simulink model "DYN_01x"  (R2018b)
(part 13 of 13)

 2*I6xy*de1*cos(e2)^2 - I6xy*de1 + 2*I6xy*de1*cos(e3)^2 + I6xy*de1*cos(e4)^2 + 2*I6xy*de1*cos(e6)^2 - (I6xx*de1*sin(2*e6))/2 + (I6yy*de1*sin(2*e6))/2 - de1*m6*x6*y6 + (de1*m6*x6^2*sin(2*e6))/2 - (de1*m6*y6^2*sin(2*e6))/2 - 4*I6xy*de1*cos(e2)^2*cos(e3)^2 - I6xy*de1*cos(e2)^2*cos(e4)^2 - I6xy*de1*cos(e2)^2*cos(e5)^2 - I6xy*de1*cos(e3)^2*cos(e4)^2 - 4*I6xy*de1*cos(e2)^2*cos(e6)^2 - I6xy*de1*cos(e3)^2*cos(e5)^2 - 4*I6xy*de1*cos(e3)^2*cos(e6)^2 + I6xy*de1*cos(e4)^2*cos(e5)^2 - 2*I6xy*de1*cos(e4)^2*cos(e6)^2 - I6xy*de4*cos(e2)*sin(e3) - I6xy*de4*cos(e3)*sin(e2) + 2*de1*m6*x6*y6*cos(e2)^2 + 2*de1*m6*x6*y6*cos(e3)^2 + de1*m6*x6*y6*cos(e4)^2 + 2*de1*m6*x6*y6*cos(e6)^2 + (I6xx*de2*cos(e2)*cos(e3)*cos(e5))/2 + (I6xx*de3*cos(e2)*cos(e3)*cos(e5))/2 - (I6yy*de2*cos(e2)*cos(e3)*cos(e5))/2 - (I6yy*de3*cos(e2)*cos(e3)*cos(e5))/2 - (I6zz*de2*cos(e2)*cos(e3)*cos(e5))/2 - (I6zz*de3*cos(e2)*cos(e3)*cos(e5))/2 - I6xx*de1*cos(e4)*cos(e5)*sin(e4) - I6xy*de5*cos(e2)*cos(e3)*sin(e4) + I6yy*de1*cos(e4)*cos(e5)*sin(e4) + 2*I6xy*de1*cos(e2)^2*cos(e3)^2*cos(e4)^2 + 2*I6xy*de1*cos(e2)^2*cos(e3)^2*cos(e5)^2 + 8*I6xy*de1*cos(e2)^2*cos(e3)^2*cos(e6)^2 - I6xy*de1*cos(e2)^2*cos(e4)^2*cos(e5)^2 + 2*I6xy*de1*cos(e2)^2*cos(e4)^2*cos(e6)^2 - I6xy*de1*cos(e3)^2*cos(e4)^2*cos(e5)^2 + 2*I6xy*de1*cos(e2)^2*cos(e5)^2*cos(e6)^2 + 2*I6xy*de1*cos(e3)^2*cos(e4)^2*cos(e6)^2 + 2*I6xy*de1*cos(e3)^2*cos(e5)^2*cos(e6)^2 - 2*I6xy*de1*cos(e4)^2*cos(e5)^2*cos(e6)^2 - (I6xx*de2*cos(e5)*sin(e2)*sin(e3))/2 - (I6xx*de3*cos(e5)*sin(e2)*sin(e3))/2 + (I6xx*de5*cos(e2)*sin(e3)*sin(e5))/2 + (I6xx*de5*cos(e3)*sin(e2)*sin(e5))/2 + (I6yy*de2*cos(e5)*sin(e2)*sin(e3))/2 + (I6yy*de3*cos(e5)*sin(e2)*sin(e3))/2 - (I6yy*de5*cos(e2)*sin(e3)*sin(e5))/2 - (I6yy*de5*cos(e3)*sin(e2)*sin(e5))/2 + (I6zz*de2*cos(e5)*sin(e2)*sin(e3))/2 + (I6zz*de3*cos(e5)*sin(e2)*sin(e3))/2 + (I6zz*de5*cos(e2)*sin(e3)*sin(e5))/2 + (I6zz*de5*cos(e3)*sin(e2)*sin(e5))/2 + I6xy*de5*sin(e2)*sin(e3)*sin(e4) + 2*I6xx*de1*cos(e2)^2*cos(e6)*sin(e6) + I6xy*de4*cos(e2)*cos(e5)^2*sin(e3) + I6xy*de4*cos(e3)*cos(e5)^2*sin(e2) + 2*I6xx*de1*cos(e3)^2*cos(e6)*sin(e6) + 2*I6xy*de4*cos(e2)*cos(e6)^2*sin(e3) + 2*I6xy*de4*cos(e3)*cos(e6)^2*sin(e2) + I6xx*de1*cos(e4)^2*cos(e6)*sin(e6) - 2*I6yy*de1*cos(e2)^2*cos(e6)*sin(e6) - 2*I6yy*de1*cos(e3)^2*cos(e6)*sin(e6) - I6yy*de1*cos(e4)^2*cos(e6)*sin(e6) - (I6xx*de5*cos(e2)*cos(e3)*cos(e4)*cos(e5))/2 + (I6yy*de5*cos(e2)*cos(e3)*cos(e4)*cos(e5))/2 + I6yz*de4*cos(e2)*cos(e3)*cos(e4)*cos(e6) - (I6zz*de5*cos(e2)*cos(e3)*cos(e4)*cos(e5))/2 - I6xy*de2*cos(e2)*cos(e3)*cos(e4)*sin(e4) - I6xy*de3*cos(e2)*cos(e3)*cos(e4)*sin(e4) + I6yz*de1*cos(e2)*cos(e4)*cos(e6)*sin(e2) + I6yz*de1*cos(e3)*cos(e4)*cos(e6)*sin(e3) + I6zx*de4*cos(e2)*cos(e3)*cos(e4)*sin(e6) + I6zx*de5*cos(e2)*cos(e5)*cos(e6)*sin(e3) + I6zx*de5*cos(e3)*cos(e5)*cos(e6)*sin(e2) + 4*I6xy*de1*cos(e2)*cos(e3)*sin(e2)*sin(e3) + (I6xx*de2*cos(e2)*cos(e4)*sin(e3)*sin(e5))/2 + (I6xx*de2*cos(e3)*cos(e4)*sin(e2)*sin(e5))/2 + (I6xx*de3*cos(e2)*cos(e4)*sin(e3)*sin(e5))/2 + (I6xx*de3*cos(e3)*cos(e4)*sin(e2)*sin(e5))/2 - (I6xx*de4*cos(e2)*cos(e3)*sin(e4)*sin(e5))/2 + (I6xx*de5*cos(e4)*cos(e5)*sin(e2)*sin(e3))/2 - I6xx*de4*cos(e2)*cos(e6)*sin(e3)*sin(e6) - I6xx*de4*cos(e3)*cos(e6)*sin(e2)*sin(e6) - (I6yy*de2*cos(e2)*cos(e4)*sin(e3)*sin(e5))/2 - (I6yy*de2*cos(e3)*cos(e4)*sin(e2)*sin(e5))/2 - (I6yy*de3*cos(e2)*cos(e4)*sin(e3)*sin(e5))/2 - (I6yy*de3*cos(e3)*cos(e4)*sin(e2)*sin(e5))/2 + (I6yy*de4*cos(e2)*cos(e3)*sin(e4)*sin(e5))/2 - (I6yy*de5*cos(e4)*cos(e5)*sin(e2)*sin(e3))/2 - I6yz*de4*cos(e4)*cos(e6)*sin(e2)*sin(e3) + I6yy*de4*cos(e2)*cos(e6)*sin(e3)*sin(e6) + I6yy*de4*cos(e3)*cos(e6)*sin(e2)*sin(e6) - I6yz*de5*cos(e2)*cos(e5)*sin(e3)*sin(e6) - I6yz*de5*cos(e3)*cos(e5)*sin(e2)*sin(e6) + I6zx*de1*cos(e2)*cos(e4)*sin(e2)*sin(e6) + I6zx*de1*cos(e3)*cos(e4)*sin(e3)*sin(e6) + (I6zz*de2*cos(e2)*cos(e4)*sin(e3)*sin(e5))/2 + (I6zz*de2*cos(e3)*cos(e4)*sin(e2)*sin(e5))/2 + (I6zz*de3*cos(e2)*cos(e4)*sin(e3)*sin(e5))/2 + (I6zz*de3*cos(e3)*cos(e4)*sin(e2)*sin(e5))/2 + I6zx*de1*cos(e4)*cos(e6)*sin(e4)*sin(e5) + (I6zz*de4*cos(e2)*cos(e3)*sin(e4)*sin(e5))/2 + (I6zz*de5*cos(e4)*cos(e5)*sin(e2)*sin(e3))/2 - I6xx*de1*cos(e2)*sin(e2)*sin(e4)*sin(e5) - I6xx*de1*cos(e3)*sin(e3)*sin(e4)*sin(e5) + I6xy*de2*cos(e4)*sin(e2)*sin(e3)*sin(e4) + I6xy*de3*cos(e4)*sin(e2)*sin(e3)*sin(e4) + I6yy*de1*cos(e2)*sin(e2)*sin(e4)*sin(e5) + I6yy*de1*cos(e3)*sin(e3)*sin(e4)*sin(e5) - I6yz*de1*cos(e4)*sin(e4)*sin(e5)*sin(e6) - I6zx*de4*cos(e4)*sin(e2)*sin(e3)*sin(e6) - de2*m6*x6^2*cos(e2)*cos(e3)*cos(e5) - de3*m6*x6^2*cos(e2)*cos(e3)*cos(e5) + (I6xx*de4*sin(e2)*sin(e3)*sin(e4)*sin(e5))/2 - (I6yy*de4*sin(e2)*sin(e3)*sin(e4)*sin(e5))/2 - (I6zz*de4*sin(e2)*sin(e3)*sin(e4)*sin(e5))/2 + de1*m6*x6^2*cos(e4)*cos(e5)*sin(e4) - 4*de1*m6*x6*y6*cos(e2)^2*cos(e3)^2 - de1*m6*x6*y6*cos(e2)^2*cos(e4)^2 - de1*m6*x6*y6*cos(e2)^2*cos(e5)^2 - de1*m6*x6*y6*cos(e3)^2*cos(e4)^2 - 4*de1*m6*x6*y6*cos(e2)^2*cos(e6)^2 - de1*m6*x6*y6*cos(e3)^2*cos(e5)^2 - 4*de1*m6*x6*y6*cos(e3)^2*cos(e6)^2 + de1*m6*x6*y6*cos(e4)^2*cos(e5)^2 - 2*de1*m6*x6*y6*cos(e4)^2*cos(e6)^2 - de1*m6*y6^2*cos(e4)*cos(e5)*sin(e4) + de2*m6*x6^2*cos(e5)*sin(e2)*sin(e3) + de3*m6*x6^2*cos(e5)*sin(e2)*sin(e3) + de5*m6*y6^2*cos(e2)*sin(e3)*sin(e5) + de5*m6*y6^2*cos(e3)*sin(e2)*sin(e5) - I6xx*de2*cos(e2)*cos(e3)*cos(e4)^2*cos(e5) - I6xx*de3*cos(e2)*cos(e3)*cos(e4)^2*cos(e5) - I6xx*de2*cos(e2)*cos(e3)*cos(e5)*cos(e6)^2 - I6xx*de3*cos(e2)*cos(e3)*cos(e5)*cos(e6)^2 + I6yy*de2*cos(e2)*cos(e3)*cos(e4)^2*cos(e5) + I6yy*de3*cos(e2)*cos(e3)*cos(e4)^2*cos(e5) + I6yy*de2*cos(e2)*cos(e3)*cos(e5)*cos(e6)^2 + I6yy*de3*cos(e2)*cos(e3)*cos(e5)*cos(e6)^2 + I6xx*de1*cos(e2)^2*cos(e4)*cos(e5)*sin(e4) + I6xx*de1*cos(e3)^2*cos(e4)*cos(e5)*sin(e4) + 2*I6xx*de1*cos(e4)*cos(e5)*cos(e6)^2*sin(e4) + 2*I6xy*de5*cos(e2)*cos(e3)*cos(e6)^2*sin(e4) - I6yy*de1*cos(e2)^2*cos(e4)*cos(e5)*sin(e4) - I6yy*de1*cos(e3)^2*cos(e4)*cos(e5)*sin(e4) - 2*I6yy*de1*cos(e4)*cos(e5)*cos(e6)^2*sin(e4) - I6yz*de1*cos(e2)^2*cos(e5)*cos(e6)*sin(e5) - I6yz*de1*cos(e3)^2*cos(e5)*cos(e6)*sin(e5) + I6yz*de1*cos(e4)^2*cos(e5)*cos(e6)*sin(e5) + 2*I6xy*de1*cos(e2)^2*cos(e3)^2*cos(e4)^2*cos(e5)^2 - 4*I6xy*de1*cos(e2)^2*cos(e3)^2*cos(e4)^2*cos(e6)^2 - 4*I6xy*de1*cos(e2)^2*cos(e3)^2*cos(e5)^2*cos(e6)^2 + 2*I6xy*de1*cos(e2)^2*cos(e4)^2*cos(e5)^2*cos(e6)^2 + 2*I6xy*de1*cos(e3)^2*cos(e4)^2*cos(e5)^2*cos(e6)^2 + I6xx*de2*cos(e4)^2*cos(e5)*sin(e2)*sin(e3) + I6xx*de3*cos(e4)^2*cos(e5)*sin(e2)*sin(e3) + I6xx*de2*cos(e5)*cos(e6)^2*sin(e2)*sin(e3) + I6xx*de3*cos(e5)*cos(e6)^2*sin(e2)*sin(e3) - I6xx*de5*cos(e2)*cos(e6)^2*sin(e3)*sin(e5) - I6xx*de5*cos(e3)*cos(e6)^2*sin(e2)*sin(e5) - I6yy*de2*cos(e4)^2*cos(e5)*sin(e2)*sin(e3) - I6yy*de3*cos(e4)^2*cos(e5)*sin(e2)*sin(e3) - I6yy*de2*cos(e5)*cos(e6)^2*sin(e2)*sin(e3) - I6yy*de3*cos(e5)*cos(e6)^2*sin(e2)*sin(e3) + I6yy*de5*cos(e2)*cos(e6)^2*sin(e3)*sin(e5) + I6yy*de5*cos(e3)*cos(e6)^2*sin(e2)*sin(e5) - I6zx*de1*cos(e2)^2*cos(e5)*sin(e5)*sin(e6) - I6zx*de1*cos(e3)^2*cos(e5)*sin(e5)*sin(e6) + I6zx*de1*cos(e4)^2*cos(e5)*sin(e5)*sin(e6) + d4*de1*m6*y6*cos(e6)*sin(e5) + d4*de1*m6*x6*sin(e5)*sin(e6) - 2*I6xy*de5*cos(e6)^2*sin(e2)*sin(e3)*sin(e4) - de4*m6*x6*y6*cos(e2)*sin(e3) - de4*m6*x6*y6*cos(e3)*sin(e2) - 2*de1*m6*x6^2*cos(e2)^2*cos(e6)*sin(e6) - 2*de1*m6*x6^2*cos(e3)^2*cos(e6)*sin(e6) - de1*m6*x6^2*cos(e4)^2*cos(e6)*sin(e6) + 2*de1*m6*y6^2*cos(e2)^2*cos(e6)*sin(e6) + 2*de1*m6*y6^2*cos(e3)^2*cos(e6)*sin(e6) + de1*m6*y6^2*cos(e4)^2*cos(e6)*sin(e6) - 4*I6xx*de1*cos(e2)^2*cos(e3)^2*cos(e6)*sin(e6) - I6xx*de1*cos(e2)^2*cos(e4)^2*cos(e6)*sin(e6) - I6xx*de1*cos(e2)^2*cos(e5)^2*cos(e6)*sin(e6) - I6xx*de1*cos(e3)^2*cos(e4)^2*cos(e6)*sin(e6) - I6xx*de1*cos(e3)^2*cos(e5)^2*cos(e6)*sin(e6) - 2*I6xy*de4*cos(e2)*cos(e5)^2*cos(e6)^2*sin(e3) - 2*I6xy*de4*cos(e3)*cos(e5)^2*cos(e6)^2*sin(e2) + I6xx*de1*cos(e4)^2*cos(e5)^2*cos(e6)*sin(e6) + 4*I6yy*de1*cos(e2)^2*cos(e3)^2*cos(e6)*sin(e6) + I6yy*de1*cos(e2)^2*cos(e4)^2*cos(e6)*sin(e6) + I6yy*de1*cos(e2)^2*cos(e5)^2*cos(e6)*sin(e6) + I6yy*de1*cos(e3)^2*cos(e4)^2*cos(e6)*sin(e6) + I6yy*de1*cos(e3)^2*cos(e5)^2*cos(e6)*sin(e6) - I6yy*de1*cos(e4)^2*cos(e5)^2*cos(e6)*sin(e6) + I6xy*de4*cos(e2)*cos(e3)*cos(e4)*cos(e5)*sin(e5) - 2*I6xy*de2*cos(e2)*cos(e3)*cos(e5)*cos(e6)*sin(e6) - 2*I6xy*de3*cos(e2)*cos(e3)*cos(e5)*cos(e6)*sin(e6) + I6zx*de2*cos(e2)*cos(e4)*cos(e5)*cos(e6)*sin(e3) + I6zx*de2*cos(e3)*cos(e4)*cos(e5)*cos(e6)*sin(e2) + I6zx*de3*cos(e2)*cos(e4)*cos(e5)*cos(e6)*sin(e3) + I6zx*de3*cos(e3)*cos(e4)*cos(e5)*cos(e6)*sin(e2) + I6zx*de5*cos(e2)*cos(e3)*cos(e4)*cos(e6)*sin(e5) + 2*I6xy*de1*cos(e2)*cos(e4)*cos(e5)*sin(e2)*sin(e5) + 2*I6xy*de1*cos(e3)*cos(e4)*cos(e5)*sin(e3)*sin(e5) - I6xx*de5*cos(e2)*cos(e3)*cos(e6)*sin(e4)*sin(e6) + 4*I6xy*de1*cos(e4)*cos(e5)*cos(e6)*sin(e4)*sin(e6) - I6yz*de2*cos(e2)*cos(e4)*cos(e5)*sin(e3)*sin(e6) - I6yz*de2*cos(e3)*cos(e4)*cos(e5)*sin(e2)*sin(e6) - I6yz*de3*cos(e2)*cos(e4)*cos(e5)*sin(e3)*sin(e6) - I6yz*de3*cos(e3)*cos(e4)*cos(e5)*sin(e2)*sin(e6) + I6yy*de5*cos(e2)*cos(e3)*cos(e6)*sin(e4)*sin(e6) + I6yz*de4*cos(e2)*cos(e5)*cos(e6)*sin(e3)*sin(e5) + I6yz*de4*cos(e3)*cos(e5)*cos(e6)*sin(e2)*sin(e5) - I6yz*de5*cos(e2)*cos(e3)*cos(e4)*sin(e5)*sin(e6) - I6zx*de1*cos(e2)*cos(e5)*cos(e6)*sin(e2)*sin(e4) - I6zx*de1*cos(e3)*cos(e5)*cos(e6)*sin(e3)*sin(e4) + 2*I6xx*de1*cos(e2)^2*cos(e3)^2*cos(e4)^2*cos(e6)*sin(e6) + 2*I6xx*de1*cos(e2)^2*cos(e3)^2*cos(e5)^2*cos(e6)*sin(e6) - I6xx*de1*cos(e2)^2*cos(e4)^2*cos(e5)^2*cos(e6)*sin(e6) - I6xx*de1*cos(e3)^2*cos(e4)^2*cos(e5)^2*cos(e6)*sin(e6) - 2*I6yy*de1*cos(e2)^2*cos(e3)^2*cos(e4)^2*cos(e6)*sin(e6) - 2*I6yy*de1*cos(e2)^2*cos(e3)^2*cos(e5)^2*cos(e6)*sin(e6) + I6yy*de1*cos(e2)^2*cos(e4)^2*cos(e5)^2*cos(e6)*sin(e6) + I6yy*de1*cos(e3)^2*cos(e4)^2*cos(e5)^2*cos(e6)*sin(e6) + I6xy*de2*cos(e2)*cos(e5)*sin(e3)*sin(e4)*sin(e5) + I6xy*de2*cos(e3)*cos(e5)*sin(e2)*sin(e4)*sin(e5) + I6xy*de3*cos(e2)*cos(e5)*sin(e3)*sin(e4)*sin(e5) + I6xy*de3*cos(e3)*cos(e5)*sin(e2)*sin(e4)*sin(e5) - I6xy*de4*cos(e4)*cos(e5)*sin(e2)*sin(e3)*sin(e5) + 2*I6xy*de2*cos(e5)*cos(e6)*sin(e2)*sin(e3)*sin(e6) + 2*I6xy*de3*cos(e5)*cos(e6)*sin(e2)*sin(e3)*sin(e6) - 2*I6xy*de5*cos(e2)*cos(e6)*sin(e3)*sin(e5)*sin(e6) - 2*I6xy*de5*cos(e3)*cos(e6)*sin(e2)*sin(e5)*sin(e6) + I6yz*de1*cos(e2)*cos(e5)*sin(e2)*sin(e4)*sin(e6) + I6yz*de1*cos(e3)*cos(e5)*sin(e3)*sin(e4)*sin(e6) + I6zx*de4*cos(e2)*cos(e5)*sin(e3)*sin(e5)*sin(e6) + I6zx*de4*cos(e3)*cos(e5)*sin(e2)*sin(e5)*sin(e6) - I6zx*de5*cos(e4)*cos(e6)*sin(e2)*sin(e3)*sin(e5) - de5*m6*y6^2*cos(e2)*cos(e3)*cos(e4)*cos(e5) + I6xx*de5*cos(e6)*sin(e2)*sin(e3)*sin(e4)*sin(e6) - I6yy*de5*cos(e6)*sin(e2)*sin(e3)*sin(e4)*sin(e6) + I6yz*de5*cos(e4)*sin(e2)*sin(e3)*sin(e5)*sin(e6) + de4*m6*x6^2*cos(e2)*cos(e3)*sin(e4)*sin(e5) + de4*m6*x6^2*cos(e2)*cos(e6)*sin(e3)*sin(e6) + de4*m6*x6^2*cos(e3)*cos(e6)*sin(e2)*sin(e6) + de2*m6*y6^2*cos(e2)*cos(e4)*sin(e3)*sin(e5) + de2*m6*y6^2*cos(e3)*cos(e4)*sin(e2)*sin(e5) + de3*m6*y6^2*cos(e2)*cos(e4)*sin(e3)*sin(e5) + de3*m6*y6^2*cos(e3)*cos(e4)*sin(e2)*sin(e5) + de5*m6*y6^2*cos(e4)*cos(e5)*sin(e2)*sin(e3) - de4*m6*y6^2*cos(e2)*cos(e6)*sin(e3)*sin(e6) - de4*m6*y6^2*cos(e3)*cos(e6)*sin(e2)*sin(e6) + I6xx*de5*cos(e2)*cos(e3)*cos(e4)*cos(e5)*cos(e6)^2 - I6yy*de5*cos(e2)*cos(e3)*cos(e4)*cos(e5)*cos(e6)^2 - I6yz*de4*cos(e2)*cos(e3)*cos(e4)*cos(e5)^2*cos(e6) + de1*m6*x6^2*cos(e2)*sin(e2)*sin(e4)*sin(e5) + de1*m6*x6^2*cos(e3)*sin(e3)*sin(e4)*sin(e5) - de1*m6*y6^2*cos(e2)*sin(e2)*sin(e4)*sin(e5) - de1*m6*y6^2*cos(e3)*sin(e3)*sin(e4)*sin(e5) - a2*de2*m6*x6*cos(e2)*cos(e4)*cos(e6) - I6xy*de2*cos(e2)*cos(e3)*cos(e4)*cos(e5)^2*sin(e4) + 2*I6xy*de2*cos(e2)*cos(e3)*cos(e4)*cos(e6)^2*sin(e4) - I6xy*de3*cos(e2)*cos(e3)*cos(e4)*cos(e5)^2*sin(e4) + 2*I6xy*de3*cos(e2)*cos(e3)*cos(e4)*cos(e6)^2*sin(e4) - 2*I6yz*de1*cos(e2)*cos(e3)^2*cos(e4)*cos(e6)*sin(e2) - 2*I6yz*de1*cos(e2)^2*cos(e3)*cos(e4)*cos(e6)*sin(e3) - 2*I6yz*de1*cos(e2)*cos(e4)*cos(e5)^2*cos(e6)*sin(e2) - 2*I6yz*de1*cos(e3)*cos(e4)*cos(e5)^2*cos(e6)*sin(e3) + I6zx*de2*cos(e2)*cos(e3)*cos(e4)^2*cos(e6)*sin(e5) + I6zx*de3*cos(e2)*cos(e3)*cos(e4)^2*cos(e6)*sin(e5) - I6zx*de4*cos(e2)*cos(e3)*cos(e4)*cos(e5)^2*sin(e6) - de4*m6*x6^2*sin(e2)*sin(e3)*sin(e4)*sin(e5) + a2*de1*m6*x6*cos(e3)*cos(e6)*sin(e4) + a2*de2*m6*y6*cos(e2)*cos(e4)*sin(e6) - 2*I6xy*de1*cos(e2)*cos(e3)*cos(e4)^2*sin(e2)*sin(e3) - 2*I6xy*de1*cos(e2)*cos(e3)*cos(e5)^2*sin(e2)*sin(e3) - 8*I6xy*de1*cos(e2)*cos(e3)*cos(e6)^2*sin(e2)*sin(e3) - I6xx*de2*cos(e2)*cos(e4)*cos(e6)^2*sin(e3)*sin(e5) - I6xx*de2*cos(e3)*cos(e4)*cos(e6)^2*sin(e2)*sin(e5) - I6xx*de3*cos(e2)*cos(e4)*cos(e6)^2*sin(e3)*sin(e5) - I6xx*de3*cos(e3)*cos(e4)*cos(e6)^2*sin(e2)*sin(e5) + I6xx*de4*cos(e2)*cos(e3)*cos(e6)^2*sin(e4)*sin(e5) - I6xx*de5*cos(e4)*cos(e5)*cos(e6)^2*sin(e2)*sin(e3) + I6xx*de4*cos(e2)*cos(e5)^2*cos(e6)*sin(e3)*sin(e6) + I6xx*de4*cos(e3)*cos(e5)^2*cos(e6)*sin(e2)*sin(e6) + I6yy*de2*cos(e2)*cos(e4)*cos(e6)^2*sin(e3)*sin(e5) + I6yy*de2*cos(e3)*cos(e4)*cos(e6)^2*sin(e2)*sin(e5) + I6yy*de3*cos(e2)*cos(e4)*cos(e6)^2*sin(e3)*sin(e5) + I6yy*de3*cos(e3)*cos(e4)*cos(e6)^2*sin(e2)*sin(e5) - I6yz*de2*cos(e2)*cos(e3)*cos(e4)^2*sin(e5)*sin(e6) - I6yz*de2*cos(e2)*cos(e5)^2*cos(e6)*sin(e3)*sin(e4) - I6yz*de2*cos(e3)*cos(e5)^2*cos(e6)*sin(e2)*sin(e4) - I6yy*de4*cos(e2)*cos(e3)*cos(e6)^2*sin(e4)*sin(e5) - I6yz*de3*cos(e2)*cos(e3)*cos(e4)^2*sin(e5)*sin(e6) - I6yz*de3*cos(e2)*cos(e5)^2*cos(e6)*sin(e3)*sin(e4) - I6yz*de3*cos(e3)*cos(e5)^2*cos(e6)*sin(e2)*sin(e4) + I6yy*de5*cos(e4)*cos(e5)*cos(e6)^2*sin(e2)*sin(e3) + I6yz*de4*cos(e4)*cos(e5)^2*cos(e6)*sin(e2)*sin(e3) - I6yy*de4*cos(e2)*cos(e5)^2*cos(e6)*sin(e3)*sin(e6) - I6yy*de4*cos(e3)*cos(e5)^2*cos(e6)*sin(e2)*sin(e6) - 2*I6zx*de1*cos(e2)*cos(e3)^2*cos(e4)*sin(e2)*sin(e6) - 2*I6zx*de1*cos(e2)^2*cos(e3)*cos(e4)*sin(e3)*sin(e6) - 2*I6zx*de1*cos(e2)*cos(e4)*cos(e5)^2*sin(e2)*sin(e6) - 2*I6zx*de1*cos(e3)*cos(e4)*cos(e5)^2*sin(e3)*sin(e6) - I6zx*de1*cos(e2)^2*cos(e4)*cos(e6)*sin(e4)*sin(e5) - I6zx*de1*cos(e3)^2*cos(e4)*cos(e6)*sin(e4)*sin(e5) - a2*de1*m6*y6*cos(e3)*sin(e4)*sin(e6) - a2*de1*m6*y6*cos(e6)*sin(e3)*sin(e5) + 2*I6xx*de1*cos(e2)*cos(e3)^2*sin(e2)*sin(e4)*sin(e5) + 2*I6xx*de1*cos(e2)^2*cos(e3)*sin(e3)*sin(e4)*sin(e5) + 2*I6xx*de1*cos(e2)*cos(e6)^2*sin(e2)*sin(e4)*sin(e5) + I6xy*de2*cos(e4)*cos(e5)^2*sin(e2)*sin(e3)*sin(e4) + 2*I6xx*de1*cos(e3)*cos(e6)^2*sin(e3)*sin(e4)*sin(e5) - 2*I6xy*de2*cos(e4)*cos(e6)^2*sin(e2)*sin(e3)*sin(e4) + I6xy*de3*cos(e4)*cos(e5)^2*sin(e2)*sin(e3)*sin(e4) - 2*I6xy*de3*cos(e4)*cos(e6)^2*sin(e2)*sin(e3)*sin(e4) - 2*I6yy*de1*cos(e2)*cos(e3)^2*sin(e2)*sin(e4)*sin(e5) - 2*I6yy*de1*cos(e2)^2*cos(e3)*sin(e3)*sin(e4)*sin(e5) - 2*I6yy*de1*cos(e2)*cos(e6)^2*sin(e2)*sin(e4)*sin(e5) - 2*I6yy*de1*cos(e3)*cos(e6)^2*sin(e3)*sin(e4)*sin(e5) + I6yz*de1*cos(e2)^2*cos(e4)*sin(e4)*sin(e5)*sin(e6) + I6yz*de1*cos(e3)^2*cos(e4)*sin(e4)*sin(e5)*sin(e6) - I6zx*de2*cos(e2)*cos(e5)^2*sin(e3)*sin(e4)*sin(e6) - I6zx*de2*cos(e3)*cos(e5)^2*sin(e2)*sin(e4)*sin(e6) - I6zx*de2*cos(e4)^2*cos(e6)*sin(e2)*sin(e3)*sin(e5) - I6zx*de3*cos(e2)*cos(e5)^2*sin(e3)*sin(e4)*sin(e6) - I6zx*de3*cos(e3)*cos(e5)^2*sin(e2)*sin(e4)*sin(e6) - I6zx*de3*cos(e4)^2*cos(e6)*sin(e2)*sin(e3)*sin(e5) + I6zx*de4*cos(e4)*cos(e5)^2*sin(e2)*sin(e3)*sin(e6) + de2*m6*x6^2*cos(e2)*cos(e3)*cos(e4)^2*cos(e5) + de3*m6*x6^2*cos(e2)*cos(e3)*cos(e4)^2*cos(e5) + de2*m6*x6^2*cos(e2)*cos(e3)*cos(e5)*cos(e6)^2 + de3*m6*x6^2*cos(e2)*cos(e3)*cos(e5)*cos(e6)^2 - de2*m6*y6^2*cos(e2)*cos(e3)*cos(e4)^2*cos(e5) - de3*m6*y6^2*cos(e2)*cos(e3)*cos(e4)^2*cos(e5) - de2*m6*y6^2*cos(e2)*cos(e3)*cos(e5)*cos(e6)^2 - de3*m6*y6^2*cos(e2)*cos(e3)*cos(e5)*cos(e6)^2 - de5*m6*x6*y6*cos(e2)*cos(e3)*sin(e4) - a2*de1*m6*x6*sin(e3)*sin(e5)*sin(e6) - I6xx*de4*cos(e6)^2*sin(e2)*sin(e3)*sin(e4)*sin(e5) + I6yz*de2*cos(e4)^2*sin(e2)*sin(e3)*sin(e5)*sin(e6) + I6yy*de4*cos(e6)^2*sin(e2)*sin(e3)*sin(e4)*sin(e5) + I6yz*de3*cos(e4)^2*sin(e2)*sin(e3)*sin(e5)*sin(e6) - de1*m6*x6^2*cos(e2)^2*cos(e4)*cos(e5)*sin(e4) - de1*m6*x6^2*cos(e3)^2*cos(e4)*cos(e5)*sin(e4) - 2*de1*m6*x6^2*cos(e4)*cos(e5)*cos(e6)^2*sin(e4) + 2*de1*m6*x6*y6*cos(e2)^2*cos(e3)^2*cos(e4)^2 + 2*de1*m6*x6*y6*cos(e2)^2*cos(e3)^2*cos(e5)^2 + 8*de1*m6*x6*y6*cos(e2)^2*cos(e3)^2*cos(e6)^2 - de1*m6*x6*y6*cos(e2)^2*cos(e4)^2*cos(e5)^2 + 2*de1*m6*x6*y6*cos(e2)^2*cos(e4)^2*cos(e6)^2 - de1*m6*x6*y6*cos(e3)^2*cos(e4)^2*cos(e5)^2 + 2*de1*m6*x6*y6*cos(e2)^2*cos(e5)^2*cos(e6)^2 + 2*de1*m6*x6*y6*cos(e3)^2*cos(e4)^2*cos(e6)^2 + 2*de1*m6*x6*y6*cos(e3)^2*cos(e5)^2*cos(e6)^2 - 2*de1*m6*x6*y6*cos(e4)^2*cos(e5)^2*cos(e6)^2 + de1*m6*y6^2*cos(e2)^2*cos(e4)*cos(e5)*sin(e4) + de1*m6*y6^2*cos(e3)^2*cos(e4)*cos(e5)*sin(e4) + 2*de1*m6*y6^2*cos(e4)*cos(e5)*cos(e6)^2*sin(e4) - de2*m6*x6^2*cos(e4)^2*cos(e5)*sin(e2)*sin(e3) - de3*m6*x6^2*cos(e4)^2*cos(e5)*sin(e2)*sin(e3) - de2*m6*x6^2*cos(e5)*cos(e6)^2*sin(e2)*sin(e3) - de3*m6*x6^2*cos(e5)*cos(e6)^2*sin(e2)*sin(e3) + de5*m6*x6^2*cos(e2)*cos(e6)^2*sin(e3)*sin(e5) + de5*m6*x6^2*cos(e3)*cos(e6)^2*sin(e2)*sin(e5) + de2*m6*y6^2*cos(e4)^2*cos(e5)*sin(e2)*sin(e3) + de3*m6*y6^2*cos(e4)^2*cos(e5)*sin(e2)*sin(e3) + de2*m6*y6^2*cos(e5)*cos(e6)^2*sin(e2)*sin(e3) + de3*m6*y6^2*cos(e5)*cos(e6)^2*sin(e2)*sin(e3) - de5*m6*y6^2*cos(e2)*cos(e6)^2*sin(e3)*sin(e5) - de5*m6*y6^2*cos(e3)*cos(e6)^2*sin(e2)*sin(e5) + de5*m6*x6*y6*sin(e2)*sin(e3)*sin(e4) + 2*I6xx*de2*cos(e2)*cos(e3)*cos(e4)^2*cos(e5)*cos(e6)^2 + 2*I6xx*de3*cos(e2)*cos(e3)*cos(e4)^2*cos(e5)*cos(e6)^2 - 2*I6yy*de2*cos(e2)*cos(e3)*cos(e4)^2*cos(e5)*cos(e6)^2 - 2*I6yy*de3*cos(e2)*cos(e3)*cos(e4)^2*cos(e5)*cos(e6)^2 - 2*I6xx*de1*cos(e2)^2*cos(e3)^2*cos(e4)*cos(e5)*sin(e4) - 2*I6xx*de1*cos(e2)^2*cos(e4)*cos(e5)*cos(e6)^2*sin(e4) - 2*I6xx*de1*cos(e3)^2*cos(e4)*cos(e5)*cos(e6)^2*sin(e4) + 2*I6yy*de1*cos(e2)^2*cos(e3)^2*cos(e4)*cos(e5)*sin(e4) + 2*I6yy*de1*cos(e2)^2*cos(e4)*cos(e5)*cos(e6)^2*sin(e4) + 2*I6yy*de1*cos(e3)^2*cos(e4)*cos(e5)*cos(e6)^2*sin(e4) + 2*I6yz*de1*cos(e2)^2*cos(e3)^2*cos(e5)*cos(e6)*sin(e5) - I6yz*de1*cos(e2)^2*cos(e4)^2*cos(e5)*cos(e6)*sin(e5) - I6yz*de1*cos(e3)^2*cos(e4)^2*cos(e5)*cos(e6)*sin(e5) + a3*de1*m6*x6*cos(e2)^2*cos(e6)*sin(e4) + a3*de1*m6*x6*cos(e3)^2*cos(e6)*sin(e4) - 4*I6xy*de1*cos(e2)^2*cos(e3)^2*cos(e4)^2*cos(e5)^2*cos(e6)^2 - 2*I6xx*de2*cos(e4)^2*cos(e5)*cos(e6)^2*sin(e2)*sin(e3) - 2*I6xx*de3*cos(e4)^2*cos(e5)*cos(e6)^2*sin(e2)*sin(e3) + 2*I6yy*de2*cos(e4)^2*cos(e5)*cos(e6)^2*sin(e2)*sin(e3) + 2*I6yy*de3*cos(e4)^2*cos(e5)*cos(e6)^2*sin(e2)*sin(e3) + 2*I6zx*de1*cos(e2)^2*cos(e3)^2*cos(e5)*sin(e5)*sin(e6) - I6zx*de1*cos(e2)^2*cos(e4)^2*cos(e5)*sin(e5)*sin(e6) - I6zx*de1*cos(e3)^2*cos(e4)^2*cos(e5)*sin(e5)*sin(e6) - d4*de1*m6*y6*cos(e2)^2*cos(e6)*sin(e5) - d4*de1*m6*y6*cos(e3)^2*cos(e6)*sin(e5) - a3*de1*m6*y6*cos(e2)^2*sin(e4)*sin(e6) - a3*de1*m6*y6*cos(e3)^2*sin(e4)*sin(e6) - d4*de1*m6*x6*cos(e2)^2*sin(e5)*sin(e6) - d4*de1*m6*x6*cos(e3)^2*sin(e5)*sin(e6) + de4*m6*x6*y6*cos(e2)*cos(e5)^2*sin(e3) + de4*m6*x6*y6*cos(e3)*cos(e5)^2*sin(e2) + 2*de4*m6*x6*y6*cos(e2)*cos(e6)^2*sin(e3) + 2*de4*m6*x6*y6*cos(e3)*cos(e6)^2*sin(e2) + 4*de1*m6*x6^2*cos(e2)^2*cos(e3)^2*cos(e6)*sin(e6) + de1*m6*x6^2*cos(e2)^2*cos(e4)^2*cos(e6)*sin(e6) + de1*m6*x6^2*cos(e2)^2*cos(e5)^2*cos(e6)*sin(e6) + de1*m6*x6^2*cos(e3)^2*cos(e4)^2*cos(e6)*sin(e6) + de1*m6*x6^2*cos(e3)^2*cos(e5)^2*cos(e6)*sin(e6) - de1*m6*x6^2*cos(e4)^2*cos(e5)^2*cos(e6)*sin(e6) - 4*de1*m6*y6^2*cos(e2)^2*cos(e3)^2*cos(e6)*sin(e6) - de1*m6*y6^2*cos(e2)^2*cos(e4)^2*cos(e6)*sin(e6) - de1*m6*y6^2*cos(e2)^2*cos(e5)^2*cos(e6)*sin(e6) - de1*m6*y6^2*cos(e3)^2*cos(e4)^2*cos(e6)*sin(e6) - de1*m6*y6^2*cos(e3)^2*cos(e5)^2*cos(e6)*sin(e6) + de1*m6*y6^2*cos(e4)^2*cos(e5)^2*cos(e6)*sin(e6) + 2*a3*de1*m6*y6*cos(e2)^2*cos(e3)^2*sin(e4)*sin(e6) + 2*d4*de1*m6*x6*cos(e2)^2*cos(e3)^2*sin(e5)*sin(e6) - 2*I6xy*de4*cos(e6)*sin(e2)*sin(e3)*sin(e4)*sin(e5)*sin(e6) + de5*m6*x6^2*cos(e2)*cos(e3)*cos(e6)*sin(e4)*sin(e6) - 2*de4*m6*x6*y6*cos(e2)*cos(e5)^2*cos(e6)^2*sin(e3) - 2*de4*m6*x6*y6*cos(e3)*cos(e5)^2*cos(e6)^2*sin(e2) - de5*m6*y6^2*cos(e2)*cos(e3)*cos(e6)*sin(e4)*sin(e6) - 2*de1*m6*x6^2*cos(e2)^2*cos(e3)^2*cos(e4)^2*cos(e6)*sin(e6) - 2*de1*m6*x6^2*cos(e2)^2*cos(e3)^2*cos(e5)^2*cos(e6)*sin(e6) + de1*m6*x6^2*cos(e2)^2*cos(e4)^2*cos(e5)^2*cos(e6)*sin(e6) + de1*m6*x6^2*cos(e3)^2*cos(e4)^2*cos(e5)^2*cos(e6)*sin(e6) + 2*de1*m6*y6^2*cos(e2)^2*cos(e3)^2*cos(e4)^2*cos(e6)*sin(e6) + 2*de1*m6*y6^2*cos(e2)^2*cos(e3)^2*cos(e5)^2*cos(e6)*sin(e6) - de1*m6*y6^2*cos(e2)^2*cos(e4)^2*cos(e5)^2*cos(e6)*sin(e6) - de1*m6*y6^2*cos(e3)^2*cos(e4)^2*cos(e5)^2*cos(e6)*sin(e6) - a3*de2*m6*x6*cos(e2)*cos(e3)*cos(e4)*cos(e6) - a3*de3*m6*x6*cos(e2)*cos(e3)*cos(e4)*cos(e6) + a2*de1*m6*y6*cos(e3)*cos(e4)*cos(e5)*cos(e6) + 4*I6xy*de2*cos(e2)*cos(e3)*cos(e4)^2*cos(e5)*cos(e6)*sin(e6) + 4*I6xy*de3*cos(e2)*cos(e3)*cos(e4)^2*cos(e5)*cos(e6)*sin(e6) - 2*I6xy*de4*cos(e2)*cos(e3)*cos(e4)*cos(e5)*cos(e6)^2*sin(e5) - de5*m6*x6^2*cos(e6)*sin(e2)*sin(e3)*sin(e4)*sin(e6) + de5*m6*y6^2*cos(e6)*sin(e2)*sin(e3)*sin(e4)*sin(e6) + a2*de1*m6*x6*cos(e3)*cos(e4)*cos(e5)*sin(e6) + a1*de1*m6*y6*cos(e2)*cos(e3)*cos(e6)*sin(e5) + a3*de2*m6*y6*cos(e2)*cos(e3)*cos(e4)*sin(e6) + a2*de2*m6*y6*cos(e2)*cos(e5)*cos(e6)*sin(e4) + a3*de3*m6*y6*cos(e2)*cos(e3)*cos(e4)*sin(e6) + d4*de2*m6*x6*cos(e2)*cos(e4)*cos(e6)*sin(e3) + d4*de2*m6*x6*cos(e3)*cos(e4)*cos(e6)*sin(e2) + d4*de3*m6*x6*cos(e2)*cos(e4)*cos(e6)*sin(e3) + d4*de3*m6*x6*cos(e3)*cos(e4)*cos(e6)*sin(e2) - 4*I6xy*de1*cos(e2)*cos(e3)^2*cos(e4)*cos(e5)*sin(e2)*sin(e5) - 4*I6xy*de1*cos(e2)^2*cos(e3)*cos(e4)*cos(e5)*sin(e3)*sin(e5) - 4*I6xy*de1*cos(e2)*cos(e4)*cos(e5)*cos(e6)^2*sin(e2)*sin(e5) - 4*I6xy*de1*cos(e3)*cos(e4)*cos(e5)*cos(e6)^2*sin(e3)*sin(e5) - 4*I6xy*de1*cos(e2)^2*cos(e4)*cos(e5)*cos(e6)*sin(e4)*sin(e6) - 4*I6xy*de1*cos(e3)^2*cos(e4)*cos(e5)*cos(e6)*sin(e4)*sin(e6) + 2*I6zx*de1*cos(e2)*cos(e3)^2*cos(e5)*cos(e6)*sin(e2)*sin(e4) + 2*I6zx*de1*cos(e2)^2*cos(e3)*cos(e5)*cos(e6)*sin(e3)*sin(e4) + de4*m6*y6*z6*cos(e2)*cos(e3)*cos(e4)*cos(e6) + a1*de1*m6*x6*cos(e2)*cos(e6)*sin(e3)*sin(e4) + a1*de1*m6*x6*cos(e3)*cos(e6)*sin(e2)*sin(e4) + a1*de1*m6*x6*cos(e2)*cos(e3)*sin(e5)*sin(e6) + a3*de2*m6*x6*cos(e4)*cos(e6)*sin(e2)*sin(e3) + a2*de2*m6*x6*cos(e2)*cos(e5)*sin(e4)*sin(e6) + a3*de3*m6*x6*cos(e4)*cos(e6)*sin(e2)*sin(e3) - a3*de1*m6*y6*cos(e2)*cos(e6)*sin(e2)*sin(e5) - a3*de1*m6*y6*cos(e3)*cos(e6)*sin(e3)*sin(e5) + 2*I6xx*de1*cos(e2)^2*cos(e3)^2*cos(e4)^2*cos(e5)^2*cos(e6)*sin(e6) - 2*I6yy*de1*cos(e2)^2*cos(e3)^2*cos(e4)^2*cos(e5)^2*cos(e6)*sin(e6) - d4*de1*m6*x6*cos(e2)*cos(e6)*sin(e2)*sin(e4) - d4*de1*m6*x6*cos(e3)*cos(e6)*sin(e3)*sin(e4) - 2*I6xy*de2*cos(e2)*cos(e5)*cos(e6)^2*sin(e3)*sin(e4)*sin(e5) - 2*I6xy*de2*cos(e3)*cos(e5)*cos(e6)^2*sin(e2)*sin(e4)*sin(e5) - 4*I6xy*de2*cos(e4)^2*cos(e5)*cos(e6)*sin(e2)*sin(e3)*sin(e6) - 2*I6xy*de3*cos(e2)*cos(e5)*cos(e6)^2*sin(e3)*sin(e4)*sin(e5) - 2*I6xy*de3*cos(e3)*cos(e5)*cos(e6)^2*sin(e2)*sin(e4)*sin(e5) - 4*I6xy*de3*cos(e4)^2*cos(e5)*cos(e6)*sin(e2)*sin(e3)*sin(e6) + 2*I6xy*de4*cos(e4)*cos(e5)*cos(e6)^2*sin(e2)*sin(e3)*sin(e5) - 2*I6yz*de1*cos(e2)*cos(e3)^2*cos(e5)*sin(e2)*sin(e4)*sin(e6) - 2*I6yz*de1*cos(e2)^2*cos(e3)*cos(e5)*sin(e3)*sin(e4)*sin(e6) - d4*de2*m6*y6*cos(e2)*cos(e4)*sin(e3)*sin(e6) - d4*de2*m6*y6*cos(e3)*cos(e4)*sin(e2)*sin(e6) - d4*de3*m6*y6*cos(e2)*cos(e4)*sin(e3)*sin(e6) - d4*de3*m6*y6*cos(e3)*cos(e4)*sin(e2)*sin(e6) - de5*m6*x6^2*cos(e2)*cos(e3)*cos(e4)*cos(e5)*cos(e6)^2 + de5*m6*y6^2*cos(e2)*cos(e3)*cos(e4)*cos(e5)*cos(e6)^2 - de2*m6*x6*y6*cos(e2)*cos(e3)*cos(e4)*sin(e4) - de3*m6*x6*y6*cos(e2)*cos(e3)*cos(e4)*sin(e4) + de4*m6*x6*z6*cos(e2)*cos(e3)*cos(e4)*sin(e6) + de5*m6*x6*z6*cos(e2)*cos(e5)*cos(e6)*sin(e3) + de5*m6*x6*z6*cos(e3)*cos(e5)*cos(e6)*sin(e2) + de1*m6*y6*z6*cos(e2)*cos(e4)*cos(e6)*sin(e2) + de1*m6*y6*z6*cos(e3)*cos(e4)*cos(e6)*sin(e3) - a3*de1*m6*x6*cos(e2)*sin(e2)*sin(e5)*sin(e6) - a3*de1*m6*x6*cos(e3)*sin(e3)*sin(e5)*sin(e6) - a1*de1*m6*y6*cos(e2)*sin(e3)*sin(e4)*sin(e6) - a1*de1*m6*y6*cos(e3)*sin(e2)*sin(e4)*sin(e6) - a1*de1*m6*y6*cos(e6)*sin(e2)*sin(e3)*sin(e5) - a3*de2*m6*y6*cos(e4)*sin(e2)*sin(e3)*sin(e6) - a3*de3*m6*y6*cos(e4)*sin(e2)*sin(e3)*sin(e6) + d4*de1*m6*y6*cos(e2)*sin(e2)*sin(e4)*sin(e6) + d4*de1*m6*y6*cos(e3)*sin(e3)*sin(e4)*sin(e6) + 4*de1*m6*x6*y6*cos(e2)*cos(e3)*sin(e2)*sin(e3) + de1*m6*x6*z6*cos(e2)*cos(e4)*sin(e2)*sin(e6) + de1*m6*x6*z6*cos(e3)*cos(e4)*sin(e3)*sin(e6) + de1*m6*x6*z6*cos(e4)*cos(e6)*sin(e4)*sin(e5) - de4*m6*y6*z6*cos(e4)*cos(e6)*sin(e2)*sin(e3) - de5*m6*y6*z6*cos(e2)*cos(e5)*sin(e3)*sin(e6) - de5*m6*y6*z6*cos(e3)*cos(e5)*sin(e2)*sin(e6) - a1*de1*m6*x6*sin(e2)*sin(e3)*sin(e5)*sin(e6) + de2*m6*x6^2*cos(e2)*cos(e4)*cos(e6)^2*sin(e3)*sin(e5) + de2*m6*x6^2*cos(e3)*cos(e4)*cos(e6)^2*sin(e2)*sin(e5) + de3*m6*x6^2*cos(e2)*cos(e4)*cos(e6)^2*sin(e3)*sin(e5) + de3*m6*x6^2*cos(e3)*cos(e4)*cos(e6)^2*sin(e2)*sin(e5) - de4*m6*x6^2*cos(e2)*cos(e3)*cos(e6)^2*sin(e4)*sin(e5) + de5*m6*x6^2*cos(e4)*cos(e5)*cos(e6)^2*sin(e2)*sin(e3) - de4*m6*x6^2*cos(e2)*cos(e5)^2*cos(e6)*sin(e3)*sin(e6) - de4*m6*x6^2*cos(e3)*cos(e5)^2*cos(e6)*sin(e2)*sin(e6) - de2*m6*y6^2*cos(e2)*cos(e4)*cos(e6)^2*sin(e3)*sin(e5) - de2*m6*y6^2*cos(e3)*cos(e4)*cos(e6)^2*sin(e2)*sin(e5) - de3*m6*y6^2*cos(e2)*cos(e4)*cos(e6)^2*sin(e3)*sin(e5) - de3*m6*y6^2*cos(e3)*cos(e4)*cos(e6)^2*sin(e2)*sin(e5) + de4*m6*y6^2*cos(e2)*cos(e3)*cos(e6)^2*sin(e4)*sin(e5) - de5*m6*y6^2*cos(e4)*cos(e5)*cos(e6)^2*sin(e2)*sin(e3) + de4*m6*y6^2*cos(e2)*cos(e5)^2*cos(e6)*sin(e3)*sin(e6) + de4*m6*y6^2*cos(e3)*cos(e5)^2*cos(e6)*sin(e2)*sin(e6) + de2*m6*x6*y6*cos(e4)*sin(e2)*sin(e3)*sin(e4) + de3*m6*x6*y6*cos(e4)*sin(e2)*sin(e3)*sin(e4) - de4*m6*x6*z6*cos(e4)*sin(e2)*sin(e3)*sin(e6) - de1*m6*y6*z6*cos(e4)*sin(e4)*sin(e5)*sin(e6) - 2*de1*m6*x6^2*cos(e2)*cos(e3)^2*sin(e2)*sin(e4)*sin(e5) - 2*de1*m6*x6^2*cos(e2)^2*cos(e3)*sin(e3)*sin(e4)*sin(e5) - 2*de1*m6*x6^2*cos(e2)*cos(e6)^2*sin(e2)*sin(e4)*sin(e5) - 2*de1*m6*x6^2*cos(e3)*cos(e6)^2*sin(e3)*sin(e4)*sin(e5) + 2*de1*m6*y6^2*cos(e2)*cos(e3)^2*sin(e2)*sin(e4)*sin(e5) + 2*de1*m6*y6^2*cos(e2)^2*cos(e3)*sin(e3)*sin(e4)*sin(e5) + 2*de1*m6*y6^2*cos(e2)*cos(e6)^2*sin(e2)*sin(e4)*sin(e5) + 2*de1*m6*y6^2*cos(e3)*cos(e6)^2*sin(e3)*sin(e4)*sin(e5) + a3*de1*m6*y6*cos(e2)^2*cos(e4)*cos(e5)*cos(e6) + a3*de1*m6*y6*cos(e3)^2*cos(e4)*cos(e5)*cos(e6) + 2*I6xy*de2*cos(e2)*cos(e3)*cos(e4)*cos(e5)^2*cos(e6)^2*sin(e4) + 2*I6xy*de3*cos(e2)*cos(e3)*cos(e4)*cos(e5)^2*cos(e6)^2*sin(e4) + 4*I6yz*de1*cos(e2)*cos(e3)^2*cos(e4)*cos(e5)^2*cos(e6)*sin(e2) + 4*I6yz*de1*cos(e2)^2*cos(e3)*cos(e4)*cos(e5)^2*cos(e6)*sin(e3) + de4*m6*x6^2*cos(e6)^2*sin(e2)*sin(e3)*sin(e4)*sin(e5) - de4*m6*y6^2*cos(e6)^2*sin(e2)*sin(e3)*sin(e4)*sin(e5) - a2*de1*m6*x6*cos(e2)^2*cos(e3)*cos(e6)*sin(e4) + a3*de1*m6*x6*cos(e2)^2*cos(e4)*cos(e5)*sin(e6) + a3*de1*m6*x6*cos(e3)^2*cos(e4)*cos(e5)*sin(e6) - 2*I6xy*de1*cos(e2)*cos(e3)*cos(e4)^2*cos(e5)^2*sin(e2)*sin(e3) + 4*I6xy*de1*cos(e2)*cos(e3)*cos(e4)^2*cos(e6)^2*sin(e2)*sin(e3) + 4*I6xy*de1*cos(e2)*cos(e3)*cos(e5)^2*cos(e6)^2*sin(e2)*sin(e3) + 4*I6zx*de1*cos(e2)*cos(e3)^2*cos(e4)*cos(e5)^2*sin(e2)*sin(e6) + 4*I6zx*de1*cos(e2)^2*cos(e3)*cos(e4)*cos(e5)^2*sin(e3)*sin(e6) + 2*I6zx*de1*cos(e2)^2*cos(e3)^2*cos(e4)*cos(e6)*sin(e4)*sin(e5) + a2*de1*m6*y6*cos(e2)^2*cos(e3)*sin(e4)*sin(e6) + a2*de1*m6*y6*cos(e2)^2*cos(e6)*sin(e3)*sin(e5) - 4*I6xx*de1*cos(e2)*cos(e3)^2*cos(e6)^2*sin(e2)*sin(e4)*sin(e5) - 4*I6xx*de1*cos(e2)^2*cos(e3)*cos(e6)^2*sin(e3)*sin(e4)*sin(e5) - 2*I6xy*de2*cos(e4)*cos(e5)^2*cos(e6)^2*sin(e2)*sin(e3)*sin(e4) - 2*I6xy*de3*cos(e4)*cos(e5)^2*cos(e6)^2*sin(e2)*sin(e3)*sin(e4) + 4*I6yy*de1*cos(e2)*cos(e3)^2*cos(e6)^2*sin(e2)*sin(e4)*sin(e5) + 4*I6yy*de1*cos(e2)^2*cos(e3)*cos(e6)^2*sin(e3)*sin(e4)*sin(e5) - 2*I6yz*de1*cos(e2)^2*cos(e3)^2*cos(e4)*sin(e4)*sin(e5)*sin(e6) - 2*de2*m6*x6^2*cos(e2)*cos(e3)*cos(e4)^2*cos(e5)*cos(e6)^2 - 2*de3*m6*x6^2*cos(e2)*cos(e3)*cos(e4)^2*cos(e5)*cos(e6)^2 + 2*de2*m6*y6^2*cos(e2)*cos(e3)*cos(e4)^2*cos(e5)*cos(e6)^2 + 2*de3*m6*y6^2*cos(e2)*cos(e3)*cos(e4)^2*cos(e5)*cos(e6)^2 + 2*de5*m6*x6*y6*cos(e2)*cos(e3)*cos(e6)^2*sin(e4) - de1*m6*y6*z6*cos(e2)^2*cos(e5)*cos(e6)*sin(e5) - de1*m6*y6*z6*cos(e3)^2*cos(e5)*cos(e6)*sin(e5) + de1*m6*y6*z6*cos(e4)^2*cos(e5)*cos(e6)*sin(e5) + a2*de1*m6*x6*cos(e2)^2*sin(e3)*sin(e5)*sin(e6) + 2*de1*m6*x6^2*cos(e2)^2*cos(e3)^2*cos(e4)*cos(e5)*sin(e4) + 2*de1*m6*x6^2*cos(e2)^2*cos(e4)*cos(e5)*cos(e6)^2*sin(e4) + 2*de1*m6*x6^2*cos(e3)^2*cos(e4)*cos(e5)*cos(e6)^2*sin(e4) + 2*de1*m6*x6*y6*cos(e2)^2*cos(e3)^2*cos(e4)^2*cos(e5)^2 - 4*de1*m6*x6*y6*cos(e2)^2*cos(e3)^2*cos(e4)^2*cos(e6)^2 - 4*de1*m6*x6*y6*cos(e2)^2*cos(e3)^2*cos(e5)^2*cos(e6)^2 + 2*de1*m6*x6*y6*cos(e2)^2*cos(e4)^2*cos(e5)^2*cos(e6)^2 + 2*de1*m6*x6*y6*cos(e3)^2*cos(e4)^2*cos(e5)^2*cos(e6)^2 - 2*de1*m6*y6^2*cos(e2)^2*cos(e3)^2*cos(e4)*cos(e5)*sin(e4) - 2*de1*m6*y6^2*cos(e2)^2*cos(e4)*cos(e5)*cos(e6)^2*sin(e4) - 2*de1*m6*y6^2*cos(e3)^2*cos(e4)*cos(e5)*cos(e6)^2*sin(e4) - de1*m6*x6*z6*cos(e2)^2*cos(e5)*sin(e5)*sin(e6) - de1*m6*x6*z6*cos(e3)^2*cos(e5)*sin(e5)*sin(e6) + de1*m6*x6*z6*cos(e4)^2*cos(e5)*sin(e5)*sin(e6) + 2*I6xy*de5*cos(e2)*cos(e3)*cos(e4)*cos(e5)*cos(e6)*sin(e6) + 2*de2*m6*x6^2*cos(e4)^2*cos(e5)*cos(e6)^2*sin(e2)*sin(e3) + 2*de3*m6*x6^2*cos(e4)^2*cos(e5)*cos(e6)^2*sin(e2)*sin(e3) - 2*de2*m6*y6^2*cos(e4)^2*cos(e5)*cos(e6)^2*sin(e2)*sin(e3) - 2*de3*m6*y6^2*cos(e4)^2*cos(e5)*cos(e6)^2*sin(e2)*sin(e3) - 2*de5*m6*x6*y6*cos(e6)^2*sin(e2)*sin(e3)*sin(e4) - I6xx*de2*cos(e2)*cos(e3)*cos(e4)*cos(e6)*sin(e4)*sin(e6) - I6xx*de3*cos(e2)*cos(e3)*cos(e4)*cos(e6)*sin(e4)*sin(e6) + I6yy*de2*cos(e2)*cos(e3)*cos(e4)*cos(e6)*sin(e4)*sin(e6) + I6yy*de3*cos(e2)*cos(e3)*cos(e4)*cos(e6)*sin(e4)*sin(e6) + 4*I6xx*de1*cos(e2)^2*cos(e3)^2*cos(e4)*cos(e5)*cos(e6)^2*sin(e4) - 4*I6yy*de1*cos(e2)^2*cos(e3)^2*cos(e4)*cos(e5)*cos(e6)^2*sin(e4) + 2*I6yz*de1*cos(e2)^2*cos(e3)^2*cos(e4)^2*cos(e5)*cos(e6)*sin(e5) + 4*I6xx*de1*cos(e2)*cos(e3)*cos(e6)*sin(e2)*sin(e3)*sin(e6) - 2*I6xy*de2*cos(e2)*cos(e4)*cos(e6)*sin(e3)*sin(e5)*sin(e6) - 2*I6xy*de2*cos(e3)*cos(e4)*cos(e6)*sin(e2)*sin(e5)*sin(e6) - 2*I6xy*de3*cos(e2)*cos(e4)*cos(e6)*sin(e3)*sin(e5)*sin(e6) - 2*I6xy*de3*cos(e3)*cos(e4)*cos(e6)*sin(e2)*sin(e5)*sin(e6) + 2*I6xy*de4*cos(e2)*cos(e3)*cos(e6)*sin(e4)*sin(e5)*sin(e6) - 2*I6xy*de5*cos(e4)*cos(e5)*cos(e6)*sin(e2)*sin(e3)*sin(e6) - 4*I6yy*de1*cos(e2)*cos(e3)*cos(e6)*sin(e2)*sin(e3)*sin(e6) - 2*a3*de1*m6*x6*cos(e2)^2*cos(e3)^2*cos(e6)*sin(e4) + 2*I6zx*de1*cos(e2)^2*cos(e3)^2*cos(e4)^2*cos(e5)*sin(e5)*sin(e6) + 2*d4*de1*m6*y6*cos(e2)^2*cos(e3)^2*cos(e6)*sin(e5) + I6xx*de2*cos(e4)*cos(e6)*sin(e2)*sin(e3)*sin(e4)*sin(e6) + 4*I6xy*de1*cos(e2)*cos(e6)*sin(e2)*sin(e4)*sin(e5)*sin(e6) + I6xx*de3*cos(e4)*cos(e6)*sin(e2)*sin(e3)*sin(e4)*sin(e6) + 4*I6xy*de1*cos(e3)*cos(e6)*sin(e3)*sin(e4)*sin(e5)*sin(e6) - I6yy*de2*cos(e4)*cos(e6)*sin(e2)*sin(e3)*sin(e4)*sin(e6) - I6yy*de3*cos(e4)*cos(e6)*sin(e2)*sin(e3)*sin(e4)*sin(e6) + a1*de1*m6*y6*cos(e2)*cos(e4)*cos(e5)*cos(e6)*sin(e3) + a1*de1*m6*y6*cos(e3)*cos(e4)*cos(e5)*cos(e6)*sin(e2) + a3*de2*m6*y6*cos(e2)*cos(e3)*cos(e5)*cos(e6)*sin(e4) + a3*de3*m6*y6*cos(e2)*cos(e3)*cos(e5)*cos(e6)*sin(e4) - I6xx*de2*cos(e2)*cos(e3)*cos(e4)*cos(e5)^2*cos(e6)*sin(e4)*sin(e6) - I6xx*de3*cos(e2)*cos(e3)*cos(e4)*cos(e5)^2*cos(e6)*sin(e4)*sin(e6) + I6yy*de2*cos(e2)*cos(e3)*cos(e4)*cos(e5)^2*cos(e6)*sin(e4)*sin(e6) + I6yy*de3*cos(e2)*cos(e3)*cos(e4)*cos(e5)^2*cos(e6)*sin(e4)*sin(e6) - d4*de1*m6*y6*cos(e2)*cos(e4)*cos(e5)*cos(e6)*sin(e2) - d4*de1*m6*y6*cos(e3)*cos(e4)*cos(e5)*cos(e6)*sin(e3) + a1*de1*m6*x6*cos(e2)*cos(e4)*cos(e5)*sin(e3)*sin(e6) + a1*de1*m6*x6*cos(e3)*cos(e4)*cos(e5)*sin(e2)*sin(e6) + a3*de2*m6*x6*cos(e2)*cos(e3)*cos(e5)*sin(e4)*sin(e6) + a3*de3*m6*x6*cos(e2)*cos(e3)*cos(e5)*sin(e4)*sin(e6) + a2*de1*m6*y6*cos(e2)*cos(e3)*cos(e6)*sin(e2)*sin(e5) - d4*de1*m6*x6*cos(e2)*cos(e4)*cos(e5)*sin(e2)*sin(e6) - d4*de1*m6*x6*cos(e3)*cos(e4)*cos(e5)*sin(e3)*sin(e6) - 2*I6xx*de1*cos(e2)*cos(e3)*cos(e4)^2*cos(e6)*sin(e2)*sin(e3)*sin(e6) - 2*I6xx*de1*cos(e2)*cos(e3)*cos(e5)^2*cos(e6)*sin(e2)*sin(e3)*sin(e6) + 2*I6yy*de1*cos(e2)*cos(e3)*cos(e4)^2*cos(e6)*sin(e2)*sin(e3)*sin(e6) + 2*I6yy*de1*cos(e2)*cos(e3)*cos(e5)^2*cos(e6)*sin(e2)*sin(e3)*sin(e6) - d4*de2*m6*y6*cos(e2)*cos(e5)*cos(e6)*sin(e3)*sin(e4) - d4*de2*m6*y6*cos(e3)*cos(e5)*cos(e6)*sin(e2)*sin(e4) - d4*de3*m6*y6*cos(e2)*cos(e5)*cos(e6)*sin(e3)*sin(e4) - d4*de3*m6*y6*cos(e3)*cos(e5)*cos(e6)*sin(e2)*sin(e4) + de4*m6*x6*y6*cos(e2)*cos(e3)*cos(e4)*cos(e5)*sin(e5) - 2*de2*m6*x6*y6*cos(e2)*cos(e3)*cos(e5)*cos(e6)*sin(e6) - 2*de3*m6*x6*y6*cos(e2)*cos(e3)*cos(e5)*cos(e6)*sin(e6) + de2*m6*x6*z6*cos(e2)*cos(e4)*cos(e5)*cos(e6)*sin(e3) + de2*m6*x6*z6*cos(e3)*cos(e4)*cos(e5)*cos(e6)*sin(e2) + de3*m6*x6*z6*cos(e2)*cos(e4)*cos(e5)*cos(e6)*sin(e3) + de3*m6*x6*z6*cos(e3)*cos(e4)*cos(e5)*cos(e6)*sin(e2) + de5*m6*x6*z6*cos(e2)*cos(e3)*cos(e4)*cos(e6)*sin(e5) + a2*de1*m6*x6*cos(e2)*cos(e6)*sin(e2)*sin(e3)*sin(e4) + a2*de1*m6*x6*cos(e2)*cos(e3)*sin(e2)*sin(e5)*sin(e6) - a3*de2*m6*y6*cos(e5)*cos(e6)*sin(e2)*sin(e3)*sin(e4) - a3*de3*m6*y6*cos(e5)*cos(e6)*sin(e2)*sin(e3)*sin(e4) - d4*de2*m6*x6*cos(e2)*cos(e5)*sin(e3)*sin(e4)*sin(e6) - d4*de2*m6*x6*cos(e3)*cos(e5)*sin(e2)*sin(e4)*sin(e6) - d4*de3*m6*x6*cos(e2)*cos(e5)*sin(e3)*sin(e4)*sin(e6) - d4*de3*m6*x6*cos(e3)*cos(e5)*sin(e2)*sin(e4)*sin(e6) - 8*I6xy*de1*cos(e2)*cos(e3)^2*cos(e6)*sin(e2)*sin(e4)*sin(e5)*sin(e6) - 8*I6xy*de1*cos(e2)^2*cos(e3)*cos(e6)*sin(e3)*sin(e4)*sin(e5)*sin(e6) + I6xx*de2*cos(e4)*cos(e5)^2*cos(e6)*sin(e2)*sin(e3)*sin(e4)*sin(e6) + I6xx*de3*cos(e4)*cos(e5)^2*cos(e6)*sin(e2)*sin(e3)*sin(e4)*sin(e6) - I6yy*de2*cos(e4)*cos(e5)^2*cos(e6)*sin(e2)*sin(e3)*sin(e4)*sin(e6) - I6yy*de3*cos(e4)*cos(e5)^2*cos(e6)*sin(e2)*sin(e3)*sin(e4)*sin(e6) + 2*de1*m6*x6*y6*cos(e2)*cos(e4)*cos(e5)*sin(e2)*sin(e5) + 2*de1*m6*x6*y6*cos(e3)*cos(e4)*cos(e5)*sin(e3)*sin(e5) + 4*de1*m6*x6*y6*cos(e4)*cos(e5)*cos(e6)*sin(e4)*sin(e6) - de1*m6*x6*z6*cos(e2)*cos(e5)*cos(e6)*sin(e2)*sin(e4) - de1*m6*x6*z6*cos(e3)*cos(e5)*cos(e6)*sin(e3)*sin(e4) - de2*m6*y6*z6*cos(e2)*cos(e4)*cos(e5)*sin(e3)*sin(e6) - de2*m6*y6*z6*cos(e3)*cos(e4)*cos(e5)*sin(e2)*sin(e6) - de3*m6*y6*z6*cos(e2)*cos(e4)*cos(e5)*sin(e3)*sin(e6) - de3*m6*y6*z6*cos(e3)*cos(e4)*cos(e5)*sin(e2)*sin(e6) + de4*m6*y6*z6*cos(e2)*cos(e5)*cos(e6)*sin(e3)*sin(e5) + de4*m6*y6*z6*cos(e3)*cos(e5)*cos(e6)*sin(e2)*sin(e5) - de5*m6*y6*z6*cos(e2)*cos(e3)*cos(e4)*sin(e5)*sin(e6) - a3*de2*m6*x6*cos(e5)*sin(e2)*sin(e3)*sin(e4)*sin(e6) - a3*de3*m6*x6*cos(e5)*sin(e2)*sin(e3)*sin(e4)*sin(e6) - a2*de1*m6*y6*cos(e2)*sin(e2)*sin(e3)*sin(e4)*sin(e6) + de2*m6*x6*y6*cos(e2)*cos(e5)*sin(e3)*sin(e4)*sin(e5) + de2*m6*x6*y6*cos(e3)*cos(e5)*sin(e2)*sin(e4)*sin(e5) + de3*m6*x6*y6*cos(e2)*cos(e5)*sin(e3)*sin(e4)*sin(e5) + de3*m6*x6*y6*cos(e3)*cos(e5)*sin(e2)*sin(e4)*sin(e5) - de4*m6*x6*y6*cos(e4)*cos(e5)*sin(e2)*sin(e3)*sin(e5) + 2*de2*m6*x6*y6*cos(e5)*cos(e6)*sin(e2)*sin(e3)*sin(e6) + 2*de3*m6*x6*y6*cos(e5)*cos(e6)*sin(e2)*sin(e3)*sin(e6) - 2*de5*m6*x6*y6*cos(e2)*cos(e6)*sin(e3)*sin(e5)*sin(e6) - 2*de5*m6*x6*y6*cos(e3)*cos(e6)*sin(e2)*sin(e5)*sin(e6) + de4*m6*x6*z6*cos(e2)*cos(e5)*sin(e3)*sin(e5)*sin(e6) + de4*m6*x6*z6*cos(e3)*cos(e5)*sin(e2)*sin(e5)*sin(e6) - de5*m6*x6*z6*cos(e4)*cos(e6)*sin(e2)*sin(e3)*sin(e5) + de1*m6*y6*z6*cos(e2)*cos(e5)*sin(e2)*sin(e4)*sin(e6) + de1*m6*y6*z6*cos(e3)*cos(e5)*sin(e3)*sin(e4)*sin(e6) - 2*de1*m6*x6^2*cos(e2)^2*cos(e3)^2*cos(e4)^2*cos(e5)^2*cos(e6)*sin(e6) + 2*de1*m6*y6^2*cos(e2)^2*cos(e3)^2*cos(e4)^2*cos(e5)^2*cos(e6)*sin(e6) + de5*m6*y6*z6*cos(e4)*sin(e2)*sin(e3)*sin(e5)*sin(e6) - a2*de1*m6*y6*cos(e2)^2*cos(e3)*cos(e4)*cos(e5)*cos(e6) - a2*de1*m6*x6*cos(e2)^2*cos(e3)*cos(e4)*cos(e5)*sin(e6) + 8*I6xy*de1*cos(e2)*cos(e3)^2*cos(e4)*cos(e5)*cos(e6)^2*sin(e2)*sin(e5) + 8*I6xy*de1*cos(e2)^2*cos(e3)*cos(e4)*cos(e5)*cos(e6)^2*sin(e3)*sin(e5) + 8*I6xy*de1*cos(e2)^2*cos(e3)^2*cos(e4)*cos(e5)*cos(e6)*sin(e4)*sin(e6) - de4*m6*y6*z6*cos(e2)*cos(e3)*cos(e4)*cos(e5)^2*cos(e6) + 2*a3*de1*m6*y6*cos(e2)*cos(e3)^2*cos(e6)*sin(e2)*sin(e5) + 2*a3*de1*m6*y6*cos(e2)^2*cos(e3)*cos(e6)*sin(e3)*sin(e5) + 2*d4*de1*m6*x6*cos(e2)*cos(e3)^2*cos(e6)*sin(e2)*sin(e4) + 2*d4*de1*m6*x6*cos(e2)^2*cos(e3)*cos(e6)*sin(e3)*sin(e4) - de2*m6*x6*y6*cos(e2)*cos(e3)*cos(e4)*cos(e5)^2*sin(e4) + 2*de2*m6*x6*y6*cos(e2)*cos(e3)*cos(e4)*cos(e6)^2*sin(e4) - de3*m6*x6*y6*cos(e2)*cos(e3)*cos(e4)*cos(e5)^2*sin(e4) + 2*de3*m6*x6*y6*cos(e2)*cos(e3)*cos(e4)*cos(e6)^2*sin(e4) + de2*m6*x6*z6*cos(e2)*cos(e3)*cos(e4)^2*cos(e6)*sin(e5) + de3*m6*x6*z6*cos(e2)*cos(e3)*cos(e4)^2*cos(e6)*sin(e5) - de4*m6*x6*z6*cos(e2)*cos(e3)*cos(e4)*cos(e5)^2*sin(e6) - 2*de1*m6*y6*z6*cos(e2)*cos(e3)^2*cos(e4)*cos(e6)*sin(e2) - 2*de1*m6*y6*z6*cos(e2)^2*cos(e3)*cos(e4)*cos(e6)*sin(e3) - 2*de1*m6*y6*z6*cos(e2)*cos(e4)*cos(e5)^2*cos(e6)*sin(e2) - 2*de1*m6*y6*z6*cos(e3)*cos(e4)*cos(e5)^2*cos(e6)*sin(e3) + 2*a3*de1*m6*x6*cos(e2)*cos(e3)^2*sin(e2)*sin(e5)*sin(e6) + 2*a3*de1*m6*x6*cos(e2)^2*cos(e3)*sin(e3)*sin(e5)*sin(e6) - 2*d4*de1*m6*y6*cos(e2)*cos(e3)^2*sin(e2)*sin(e4)*sin(e6) - 2*d4*de1*m6*y6*cos(e2)^2*cos(e3)*sin(e3)*sin(e4)*sin(e6) - 2*de1*m6*x6*y6*cos(e2)*cos(e3)*cos(e4)^2*sin(e2)*sin(e3) - 2*de1*m6*x6*y6*cos(e2)*cos(e3)*cos(e5)^2*sin(e2)*sin(e3) - 8*de1*m6*x6*y6*cos(e2)*cos(e3)*cos(e6)^2*sin(e2)*sin(e3) - 2*de1*m6*x6*z6*cos(e2)*cos(e3)^2*cos(e4)*sin(e2)*sin(e6) - 2*de1*m6*x6*z6*cos(e2)^2*cos(e3)*cos(e4)*sin(e3)*sin(e6) - 2*de1*m6*x6*z6*cos(e2)*cos(e4)*cos(e5)^2*sin(e2)*sin(e6) - 2*de1*m6*x6*z6*cos(e3)*cos(e4)*cos(e5)^2*sin(e3)*sin(e6) - de1*m6*x6*z6*cos(e2)^2*cos(e4)*cos(e6)*sin(e4)*sin(e5) - de1*m6*x6*z6*cos(e3)^2*cos(e4)*cos(e6)*sin(e4)*sin(e5) - de2*m6*y6*z6*cos(e2)*cos(e3)*cos(e4)^2*sin(e5)*sin(e6) - de2*m6*y6*z6*cos(e2)*cos(e5)^2*cos(e6)*sin(e3)*sin(e4) - de2*m6*y6*z6*cos(e3)*cos(e5)^2*cos(e6)*sin(e2)*sin(e4) - de3*m6*y6*z6*cos(e2)*cos(e3)*cos(e4)^2*sin(e5)*sin(e6) - de3*m6*y6*z6*cos(e2)*cos(e5)^2*cos(e6)*sin(e3)*sin(e4) - de3*m6*y6*z6*cos(e3)*cos(e5)^2*cos(e6)*sin(e2)*sin(e4) + de4*m6*y6*z6*cos(e4)*cos(e5)^2*cos(e6)*sin(e2)*sin(e3) + de2*m6*x6*y6*cos(e4)*cos(e5)^2*sin(e2)*sin(e3)*sin(e4) - 2*de2*m6*x6*y6*cos(e4)*cos(e6)^2*sin(e2)*sin(e3)*sin(e4) + de3*m6*x6*y6*cos(e4)*cos(e5)^2*sin(e2)*sin(e3)*sin(e4) - 2*de3*m6*x6*y6*cos(e4)*cos(e6)^2*sin(e2)*sin(e3)*sin(e4) - de2*m6*x6*z6*cos(e2)*cos(e5)^2*sin(e3)*sin(e4)*sin(e6) - de2*m6*x6*z6*cos(e3)*cos(e5)^2*sin(e2)*sin(e4)*sin(e6) - de2*m6*x6*z6*cos(e4)^2*cos(e6)*sin(e2)*sin(e3)*sin(e5) - de3*m6*x6*z6*cos(e2)*cos(e5)^2*sin(e3)*sin(e4)*sin(e6) - de3*m6*x6*z6*cos(e3)*cos(e5)^2*sin(e2)*sin(e4)*sin(e6) - de3*m6*x6*z6*cos(e4)^2*cos(e6)*sin(e2)*sin(e3)*sin(e5) + de4*m6*x6*z6*cos(e4)*cos(e5)^2*sin(e2)*sin(e3)*sin(e6) + de1*m6*y6*z6*cos(e2)^2*cos(e4)*sin(e4)*sin(e5)*sin(e6) + de1*m6*y6*z6*cos(e3)^2*cos(e4)*sin(e4)*sin(e5)*sin(e6) + I6xx*de4*cos(e2)*cos(e3)*cos(e4)*cos(e5)*cos(e6)*sin(e5)*sin(e6) - I6yz*de2*cos(e2)*cos(e3)*cos(e4)*cos(e5)*cos(e6)*sin(e4)*sin(e5) - I6yz*de3*cos(e2)*cos(e3)*cos(e4)*cos(e5)*cos(e6)*sin(e4)*sin(e5) - I6yy*de4*cos(e2)*cos(e3)*cos(e4)*cos(e5)*cos(e6)*sin(e5)*sin(e6) + 4*de1*m6*x6^2*cos(e2)*cos(e3)^2*cos(e6)^2*sin(e2)*sin(e4)*sin(e5) + 4*de1*m6*x6^2*cos(e2)^2*cos(e3)*cos(e6)^2*sin(e3)*sin(e4)*sin(e5) - 4*de1*m6*y6^2*cos(e2)*cos(e3)^2*cos(e6)^2*sin(e2)*sin(e4)*sin(e5) - 4*de1*m6*y6^2*cos(e2)^2*cos(e3)*cos(e6)^2*sin(e3)*sin(e4)*sin(e5) + de2*m6*y6*z6*cos(e4)^2*sin(e2)*sin(e3)*sin(e5)*sin(e6) + de3*m6*y6*z6*cos(e4)^2*sin(e2)*sin(e3)*sin(e5)*sin(e6) - 2*a3*de1*m6*y6*cos(e2)^2*cos(e3)^2*cos(e4)*cos(e5)*cos(e6) + 2*I6xx*de1*cos(e2)*cos(e3)*cos(e4)*cos(e5)*sin(e2)*sin(e3)*sin(e4) + 2*I6xx*de1*cos(e2)*cos(e4)*cos(e5)*cos(e6)*sin(e2)*sin(e5)*sin(e6) + 2*I6xx*de1*cos(e3)*cos(e4)*cos(e5)*cos(e6)*sin(e3)*sin(e5)*sin(e6) - 2*I6yy*de1*cos(e2)*cos(e3)*cos(e4)*cos(e5)*sin(e2)*sin(e3)*sin(e4) - 2*I6yz*de1*cos(e2)*cos(e3)*cos(e5)*cos(e6)*sin(e2)*sin(e3)*sin(e5) - 2*I6yy*de1*cos(e2)*cos(e4)*cos(e5)*cos(e6)*sin(e2)*sin(e5)*sin(e6) - 2*I6yy*de1*cos(e3)*cos(e4)*cos(e5)*cos(e6)*sin(e3)*sin(e5)*sin(e6) - I6zx*de2*cos(e2)*cos(e3)*cos(e4)*cos(e5)*sin(e4)*sin(e5)*sin(e6) - I6zx*de3*cos(e2)*cos(e3)*cos(e4)*cos(e5)*sin(e4)*sin(e5)*sin(e6) - 2*a3*de1*m6*x6*cos(e2)^2*cos(e3)^2*cos(e4)*cos(e5)*sin(e6) + 4*I6xy*de1*cos(e2)*cos(e3)*cos(e4)^2*cos(e5)^2*cos(e6)^2*sin(e2)*sin(e3) + I6xx*de2*cos(e2)*cos(e5)*cos(e6)*sin(e3)*sin(e4)*sin(e5)*sin(e6) + I6xx*de2*cos(e3)*cos(e5)*cos(e6)*sin(e2)*sin(e4)*sin(e5)*sin(e6) + I6xx*de3*cos(e2)*cos(e5)*cos(e6)*sin(e3)*sin(e4)*sin(e5)*sin(e6) + I6xx*de3*cos(e3)*cos(e5)*cos(e6)*sin(e2)*sin(e4)*sin(e5)*sin(e6) - I6xx*de4*cos(e4)*cos(e5)*cos(e6)*sin(e2)*sin(e3)*sin(e5)*sin(e6) + I6yz*de2*cos(e4)*cos(e5)*cos(e6)*sin(e2)*sin(e3)*sin(e4)*sin(e5) - I6yy*de2*cos(e2)*cos(e5)*cos(e6)*sin(e3)*sin(e4)*sin(e5)*sin(e6) - I6yy*de2*cos(e3)*cos(e5)*cos(e6)*sin(e2)*sin(e4)*sin(e5)*sin(e6) + I6yz*de3*cos(e4)*cos(e5)*cos(e6)*sin(e2)*sin(e3)*sin(e4)*sin(e5) - I6yy*de3*cos(e2)*cos(e5)*cos(e6)*sin(e3)*sin(e4)*sin(e5)*sin(e6) - I6yy*de3*cos(e3)*cos(e5)*cos(e6)*sin(e2)*sin(e4)*sin(e5)*sin(e6) + I6yy*de4*cos(e4)*cos(e5)*cos(e6)*sin(e2)*sin(e3)*sin(e5)*sin(e6) - 2*I6zx*de1*cos(e2)*cos(e3)*cos(e5)*sin(e2)*sin(e3)*sin(e5)*sin(e6) + I6zx*de2*cos(e4)*cos(e5)*sin(e2)*sin(e3)*sin(e4)*sin(e5)*sin(e6) + I6zx*de3*cos(e4)*cos(e5)*sin(e2)*sin(e3)*sin(e4)*sin(e5)*sin(e6) + de2*m6*x6^2*cos(e2)*cos(e3)*cos(e4)*cos(e6)*sin(e4)*sin(e6) + de3*m6*x6^2*cos(e2)*cos(e3)*cos(e4)*cos(e6)*sin(e4)*sin(e6) - de2*m6*y6^2*cos(e2)*cos(e3)*cos(e4)*cos(e6)*sin(e4)*sin(e6) - de3*m6*y6^2*cos(e2)*cos(e3)*cos(e4)*cos(e6)*sin(e4)*sin(e6) + 2*de1*m6*y6*z6*cos(e2)^2*cos(e3)^2*cos(e5)*cos(e6)*sin(e5) - de1*m6*y6*z6*cos(e2)^2*cos(e4)^2*cos(e5)*cos(e6)*sin(e5) - de1*m6*y6*z6*cos(e3)^2*cos(e4)^2*cos(e5)*cos(e6)*sin(e5) - 4*de1*m6*x6^2*cos(e2)^2*cos(e3)^2*cos(e4)*cos(e5)*cos(e6)^2*sin(e4) - 4*de1*m6*x6*y6*cos(e2)^2*cos(e3)^2*cos(e4)^2*cos(e5)^2*cos(e6)^2 + 4*de1*m6*y6^2*cos(e2)^2*cos(e3)^2*cos(e4)*cos(e5)*cos(e6)^2*sin(e4) - 4*de1*m6*x6^2*cos(e2)*cos(e3)*cos(e6)*sin(e2)*sin(e3)*sin(e6) + 4*de1*m6*y6^2*cos(e2)*cos(e3)*cos(e6)*sin(e2)*sin(e3)*sin(e6) + 2*de1*m6*x6*z6*cos(e2)^2*cos(e3)^2*cos(e5)*sin(e5)*sin(e6) - de1*m6*x6*z6*cos(e2)^2*cos(e4)^2*cos(e5)*sin(e5)*sin(e6) - de1*m6*x6*z6*cos(e3)^2*cos(e4)^2*cos(e5)*sin(e5)*sin(e6) - de2*m6*x6^2*cos(e4)*cos(e6)*sin(e2)*sin(e3)*sin(e4)*sin(e6) - de3*m6*x6^2*cos(e4)*cos(e6)*sin(e2)*sin(e3)*sin(e4)*sin(e6) + de2*m6*y6^2*cos(e4)*cos(e6)*sin(e2)*sin(e3)*sin(e4)*sin(e6) + de3*m6*y6^2*cos(e4)*cos(e6)*sin(e2)*sin(e3)*sin(e4)*sin(e6) + de2*m6*x6^2*cos(e2)*cos(e3)*cos(e4)*cos(e5)^2*cos(e6)*sin(e4)*sin(e6) + de3*m6*x6^2*cos(e2)*cos(e3)*cos(e4)*cos(e5)^2*cos(e6)*sin(e4)*sin(e6) - de2*m6*y6^2*cos(e2)*cos(e3)*cos(e4)*cos(e5)^2*cos(e6)*sin(e4)*sin(e6) - de3*m6*y6^2*cos(e2)*cos(e3)*cos(e4)*cos(e5)^2*cos(e6)*sin(e4)*sin(e6) - 2*de2*m6*x6*y6*cos(e2)*cos(e4)*cos(e6)*sin(e3)*sin(e5)*sin(e6) - 2*de2*m6*x6*y6*cos(e3)*cos(e4)*cos(e6)*sin(e2)*sin(e5)*sin(e6) - 2*de3*m6*x6*y6*cos(e2)*cos(e4)*cos(e6)*sin(e3)*sin(e5)*sin(e6) - 2*de3*m6*x6*y6*cos(e3)*cos(e4)*cos(e6)*sin(e2)*sin(e5)*sin(e6) + 2*de4*m6*x6*y6*cos(e2)*cos(e3)*cos(e6)*sin(e4)*sin(e5)*sin(e6) - 2*de5*m6*x6*y6*cos(e4)*cos(e5)*cos(e6)*sin(e2)*sin(e3)*sin(e6) + 2*de1*m6*y6*z6*cos(e2)^2*cos(e3)^2*cos(e4)^2*cos(e5)*cos(e6)*sin(e5) + 2*de1*m6*x6^2*cos(e2)*cos(e3)*cos(e4)^2*cos(e6)*sin(e2)*sin(e3)*sin(e6) + 2*de1*m6*x6^2*cos(e2)*cos(e3)*cos(e5)^2*cos(e6)*sin(e2)*sin(e3)*sin(e6) - 2*de1*m6*y6^2*cos(e2)*cos(e3)*cos(e4)^2*cos(e6)*sin(e2)*sin(e3)*sin(e6) - 2*de1*m6*y6^2*cos(e2)*cos(e3)*cos(e5)^2*cos(e6)*sin(e2)*sin(e3)*sin(e6) + 2*de1*m6*x6*z6*cos(e2)^2*cos(e3)^2*cos(e4)^2*cos(e5)*sin(e5)*sin(e6) + 4*de1*m6*x6*y6*cos(e2)*cos(e6)*sin(e2)*sin(e4)*sin(e5)*sin(e6) + 4*de1*m6*x6*y6*cos(e3)*cos(e6)*sin(e3)*sin(e4)*sin(e5)*sin(e6) - de2*m6*x6^2*cos(e4)*cos(e5)^2*cos(e6)*sin(e2)*sin(e3)*sin(e4)*sin(e6) - de3*m6*x6^2*cos(e4)*cos(e5)^2*cos(e6)*sin(e2)*sin(e3)*sin(e4)*sin(e6) + de2*m6*y6^2*cos(e4)*cos(e5)^2*cos(e6)*sin(e2)*sin(e3)*sin(e4)*sin(e6) + de3*m6*y6^2*cos(e4)*cos(e5)^2*cos(e6)*sin(e2)*sin(e3)*sin(e4)*sin(e6) - 2*de4*m6*x6*y6*cos(e6)*sin(e2)*sin(e3)*sin(e4)*sin(e5)*sin(e6) + 2*d4*de1*m6*y6*cos(e2)*cos(e3)^2*cos(e4)*cos(e5)*cos(e6)*sin(e2) + 2*d4*de1*m6*y6*cos(e2)^2*cos(e3)*cos(e4)*cos(e5)*cos(e6)*sin(e3) + 2*d4*de1*m6*x6*cos(e2)*cos(e3)^2*cos(e4)*cos(e5)*sin(e2)*sin(e6) + 2*d4*de1*m6*x6*cos(e2)^2*cos(e3)*cos(e4)*cos(e5)*sin(e3)*sin(e6) - 2*I6xx*de1*cos(e2)*cos(e3)*cos(e4)^2*cos(e5)^2*cos(e6)*sin(e2)*sin(e3)*sin(e6) + 2*I6yy*de1*cos(e2)*cos(e3)*cos(e4)^2*cos(e5)^2*cos(e6)*sin(e2)*sin(e3)*sin(e6) + 4*de2*m6*x6*y6*cos(e2)*cos(e3)*cos(e4)^2*cos(e5)*cos(e6)*sin(e6) + 4*de3*m6*x6*y6*cos(e2)*cos(e3)*cos(e4)^2*cos(e5)*cos(e6)*sin(e6) - 2*de4*m6*x6*y6*cos(e2)*cos(e3)*cos(e4)*cos(e5)*cos(e6)^2*sin(e5) - 4*de1*m6*x6*y6*cos(e2)*cos(e3)^2*cos(e4)*cos(e5)*sin(e2)*sin(e5) - 4*de1*m6*x6*y6*cos(e2)^2*cos(e3)*cos(e4)*cos(e5)*sin(e3)*sin(e5) - 4*de1*m6*x6*y6*cos(e2)*cos(e4)*cos(e5)*cos(e6)^2*sin(e2)*sin(e5) - 4*de1*m6*x6*y6*cos(e3)*cos(e4)*cos(e5)*cos(e6)^2*sin(e3)*sin(e5) - 4*de1*m6*x6*y6*cos(e2)^2*cos(e4)*cos(e5)*cos(e6)*sin(e4)*sin(e6) - 4*de1*m6*x6*y6*cos(e3)^2*cos(e4)*cos(e5)*cos(e6)*sin(e4)*sin(e6) + 2*de1*m6*x6*z6*cos(e2)*cos(e3)^2*cos(e5)*cos(e6)*sin(e2)*sin(e4) + 2*de1*m6*x6*z6*cos(e2)^2*cos(e3)*cos(e5)*cos(e6)*sin(e3)*sin(e4) - 2*de2*m6*x6*y6*cos(e2)*cos(e5)*cos(e6)^2*sin(e3)*sin(e4)*sin(e5) - 2*de2*m6*x6*y6*cos(e3)*cos(e5)*cos(e6)^2*sin(e2)*sin(e4)*sin(e5) - 4*de2*m6*x6*y6*cos(e4)^2*cos(e5)*cos(e6)*sin(e2)*sin(e3)*sin(e6) - 2*de3*m6*x6*y6*cos(e2)*cos(e5)*cos(e6)^2*sin(e3)*sin(e4)*sin(e5) - 2*de3*m6*x6*y6*cos(e3)*cos(e5)*cos(e6)^2*sin(e2)*sin(e4)*sin(e5) - 4*de3*m6*x6*y6*cos(e4)^2*cos(e5)*cos(e6)*sin(e2)*sin(e3)*sin(e6) + 2*de4*m6*x6*y6*cos(e4)*cos(e5)*cos(e6)^2*sin(e2)*sin(e3)*sin(e5) - 2*de1*m6*y6*z6*cos(e2)*cos(e3)^2*cos(e5)*sin(e2)*sin(e4)*sin(e6) - 2*de1*m6*y6*z6*cos(e2)^2*cos(e3)*cos(e5)*sin(e3)*sin(e4)*sin(e6) - 2*I6zx*de1*cos(e2)*cos(e3)*cos(e4)*cos(e6)*sin(e2)*sin(e3)*sin(e4)*sin(e5) + 2*I6yz*de1*cos(e2)*cos(e3)*cos(e4)*sin(e2)*sin(e3)*sin(e4)*sin(e5)*sin(e6) - de4*m6*x6^2*cos(e2)*cos(e3)*cos(e4)*cos(e5)*cos(e6)*sin(e5)*sin(e6) + 2*de2*m6*x6*y6*cos(e2)*cos(e3)*cos(e4)*cos(e5)^2*cos(e6)^2*sin(e4) + 2*de3*m6*x6*y6*cos(e2)*cos(e3)*cos(e4)*cos(e5)^2*cos(e6)^2*sin(e4) + de4*m6*y6^2*cos(e2)*cos(e3)*cos(e4)*cos(e5)*cos(e6)*sin(e5)*sin(e6) + 4*de1*m6*y6*z6*cos(e2)*cos(e3)^2*cos(e4)*cos(e5)^2*cos(e6)*sin(e2) + 4*de1*m6*y6*z6*cos(e2)^2*cos(e3)*cos(e4)*cos(e5)^2*cos(e6)*sin(e3) - 2*de1*m6*x6^2*cos(e2)*cos(e3)*cos(e4)*cos(e5)*sin(e2)*sin(e3)*sin(e4) - 2*de1*m6*x6^2*cos(e2)*cos(e4)*cos(e5)*cos(e6)*sin(e2)*sin(e5)*sin(e6) - 2*de1*m6*x6^2*cos(e3)*cos(e4)*cos(e5)*cos(e6)*sin(e3)*sin(e5)*sin(e6) - 2*de1*m6*x6*y6*cos(e2)*cos(e3)*cos(e4)^2*cos(e5)^2*sin(e2)*sin(e3) + 4*de1*m6*x6*y6*cos(e2)*cos(e3)*cos(e4)^2*cos(e6)^2*sin(e2)*sin(e3) + 4*de1*m6*x6*y6*cos(e2)*cos(e3)*cos(e5)^2*cos(e6)^2*sin(e2)*sin(e3) + 2*de1*m6*y6^2*cos(e2)*cos(e3)*cos(e4)*cos(e5)*sin(e2)*sin(e3)*sin(e4) + 2*de1*m6*y6^2*cos(e2)*cos(e4)*cos(e5)*cos(e6)*sin(e2)*sin(e5)*sin(e6) + 2*de1*m6*y6^2*cos(e3)*cos(e4)*cos(e5)*cos(e6)*sin(e3)*sin(e5)*sin(e6) + 4*de1*m6*x6*z6*cos(e2)*cos(e3)^2*cos(e4)*cos(e5)^2*sin(e2)*sin(e6) + 4*de1*m6*x6*z6*cos(e2)^2*cos(e3)*cos(e4)*cos(e5)^2*sin(e3)*sin(e6) + 2*de1*m6*x6*z6*cos(e2)^2*cos(e3)^2*cos(e4)*cos(e6)*sin(e4)*sin(e5) - de2*m6*x6^2*cos(e2)*cos(e5)*cos(e6)*sin(e3)*sin(e4)*sin(e5)*sin(e6) - de2*m6*x6^2*cos(e3)*cos(e5)*cos(e6)*sin(e2)*sin(e4)*sin(e5)*sin(e6) - de3*m6*x6^2*cos(e2)*cos(e5)*cos(e6)*sin(e3)*sin(e4)*sin(e5)*sin(e6) - de3*m6*x6^2*cos(e3)*cos(e5)*cos(e6)*sin(e2)*sin(e4)*sin(e5)*sin(e6) + de4*m6*x6^2*cos(e4)*cos(e5)*cos(e6)*sin(e2)*sin(e3)*sin(e5)*sin(e6) - 2*de2*m6*x6*y6*cos(e4)*cos(e5)^2*cos(e6)^2*sin(e2)*sin(e3)*sin(e4) - 2*de3*m6*x6*y6*cos(e4)*cos(e5)^2*cos(e6)^2*sin(e2)*sin(e3)*sin(e4) + de2*m6*y6^2*cos(e2)*cos(e5)*cos(e6)*sin(e3)*sin(e4)*sin(e5)*sin(e6) + de2*m6*y6^2*cos(e3)*cos(e5)*cos(e6)*sin(e2)*sin(e4)*sin(e5)*sin(e6) + de3*m6*y6^2*cos(e2)*cos(e5)*cos(e6)*sin(e3)*sin(e4)*sin(e5)*sin(e6) + de3*m6*y6^2*cos(e3)*cos(e5)*cos(e6)*sin(e2)*sin(e4)*sin(e5)*sin(e6) - de4*m6*y6^2*cos(e4)*cos(e5)*cos(e6)*sin(e2)*sin(e3)*sin(e5)*sin(e6) - 2*de1*m6*y6*z6*cos(e2)^2*cos(e3)^2*cos(e4)*sin(e4)*sin(e5)*sin(e6) + a2*de1*m6*y6*cos(e2)*cos(e4)*cos(e5)*cos(e6)*sin(e2)*sin(e3) - 4*I6xx*de1*cos(e2)*cos(e3)*cos(e4)*cos(e5)*cos(e6)^2*sin(e2)*sin(e3)*sin(e4) - 4*I6xx*de1*cos(e2)*cos(e3)^2*cos(e4)*cos(e5)*cos(e6)*sin(e2)*sin(e5)*sin(e6) - 4*I6xx*de1*cos(e2)^2*cos(e3)*cos(e4)*cos(e5)*cos(e6)*sin(e3)*sin(e5)*sin(e6) + 4*I6yy*de1*cos(e2)*cos(e3)*cos(e4)*cos(e5)*cos(e6)^2*sin(e2)*sin(e3)*sin(e4) - 2*I6yz*de1*cos(e2)*cos(e3)*cos(e4)^2*cos(e5)*cos(e6)*sin(e2)*sin(e3)*sin(e5) + 4*I6yy*de1*cos(e2)*cos(e3)^2*cos(e4)*cos(e5)*cos(e6)*sin(e2)*sin(e5)*sin(e6) + 4*I6yy*de1*cos(e2)^2*cos(e3)*cos(e4)*cos(e5)*cos(e6)*sin(e3)*sin(e5)*sin(e6) + 2*de5*m6*x6*y6*cos(e2)*cos(e3)*cos(e4)*cos(e5)*cos(e6)*sin(e6) + 2*a3*de1*m6*x6*cos(e2)*cos(e3)*cos(e6)*sin(e2)*sin(e3)*sin(e4) + a2*de1*m6*x6*cos(e2)*cos(e4)*cos(e5)*sin(e2)*sin(e3)*sin(e6) - 2*I6zx*de1*cos(e2)*cos(e3)*cos(e4)^2*cos(e5)*sin(e2)*sin(e3)*sin(e5)*sin(e6) - 2*d4*de1*m6*y6*cos(e2)*cos(e3)*cos(e6)*sin(e2)*sin(e3)*sin(e5) - 2*a3*de1*m6*y6*cos(e2)*cos(e3)*sin(e2)*sin(e3)*sin(e4)*sin(e6) - 2*d4*de1*m6*x6*cos(e2)*cos(e3)*sin(e2)*sin(e3)*sin(e5)*sin(e6) + 2*de1*m6*x6^2*cos(e2)*cos(e3)*cos(e4)^2*cos(e5)^2*cos(e6)*sin(e2)*sin(e3)*sin(e6) - 2*de1*m6*y6^2*cos(e2)*cos(e3)*cos(e4)^2*cos(e5)^2*cos(e6)*sin(e2)*sin(e3)*sin(e6) - 8*de1*m6*x6*y6*cos(e2)*cos(e3)^2*cos(e6)*sin(e2)*sin(e4)*sin(e5)*sin(e6) - 8*de1*m6*x6*y6*cos(e2)^2*cos(e3)*cos(e6)*sin(e3)*sin(e4)*sin(e5)*sin(e6) - 8*I6xy*de1*cos(e2)*cos(e3)*cos(e4)*cos(e5)*cos(e6)*sin(e2)*sin(e3)*sin(e4)*sin(e6) + 8*de1*m6*x6*y6*cos(e2)*cos(e3)^2*cos(e4)*cos(e5)*cos(e6)^2*sin(e2)*sin(e5) + 8*de1*m6*x6*y6*cos(e2)^2*cos(e3)*cos(e4)*cos(e5)*cos(e6)^2*sin(e3)*sin(e5) + 8*de1*m6*x6*y6*cos(e2)^2*cos(e3)^2*cos(e4)*cos(e5)*cos(e6)*sin(e4)*sin(e6) + 2*a3*de1*m6*y6*cos(e2)*cos(e3)*cos(e4)*cos(e5)*cos(e6)*sin(e2)*sin(e3) + 2*a3*de1*m6*x6*cos(e2)*cos(e3)*cos(e4)*cos(e5)*sin(e2)*sin(e3)*sin(e6) - de2*m6*y6*z6*cos(e2)*cos(e3)*cos(e4)*cos(e5)*cos(e6)*sin(e4)*sin(e5) - de3*m6*y6*z6*cos(e2)*cos(e3)*cos(e4)*cos(e5)*cos(e6)*sin(e4)*sin(e5) - de2*m6*x6*z6*cos(e2)*cos(e3)*cos(e4)*cos(e5)*sin(e4)*sin(e5)*sin(e6) - de3*m6*x6*z6*cos(e2)*cos(e3)*cos(e4)*cos(e5)*sin(e4)*sin(e5)*sin(e6) - 2*de1*m6*y6*z6*cos(e2)*cos(e3)*cos(e5)*cos(e6)*sin(e2)*sin(e3)*sin(e5) + 4*de1*m6*x6^2*cos(e2)*cos(e3)*cos(e4)*cos(e5)*cos(e6)^2*sin(e2)*sin(e3)*sin(e4) + 4*de1*m6*x6^2*cos(e2)*cos(e3)^2*cos(e4)*cos(e5)*cos(e6)*sin(e2)*sin(e5)*sin(e6) + 4*de1*m6*x6^2*cos(e2)^2*cos(e3)*cos(e4)*cos(e5)*cos(e6)*sin(e3)*sin(e5)*sin(e6) + 4*de1*m6*x6*y6*cos(e2)*cos(e3)*cos(e4)^2*cos(e5)^2*cos(e6)^2*sin(e2)*sin(e3) - 4*de1*m6*y6^2*cos(e2)*cos(e3)*cos(e4)*cos(e5)*cos(e6)^2*sin(e2)*sin(e3)*sin(e4) - 4*de1*m6*y6^2*cos(e2)*cos(e3)^2*cos(e4)*cos(e5)*cos(e6)*sin(e2)*sin(e5)*sin(e6) - 4*de1*m6*y6^2*cos(e2)^2*cos(e3)*cos(e4)*cos(e5)*cos(e6)*sin(e3)*sin(e5)*sin(e6) - 2*de1*m6*x6*z6*cos(e2)*cos(e3)*cos(e5)*sin(e2)*sin(e3)*sin(e5)*sin(e6) + de2*m6*y6*z6*cos(e4)*cos(e5)*cos(e6)*sin(e2)*sin(e3)*sin(e4)*sin(e5) + de3*m6*y6*z6*cos(e4)*cos(e5)*cos(e6)*sin(e2)*sin(e3)*sin(e4)*sin(e5) + de2*m6*x6*z6*cos(e4)*cos(e5)*sin(e2)*sin(e3)*sin(e4)*sin(e5)*sin(e6) + de3*m6*x6*z6*cos(e4)*cos(e5)*sin(e2)*sin(e3)*sin(e4)*sin(e5)*sin(e6) - 2*de1*m6*x6*z6*cos(e2)*cos(e3)*cos(e4)^2*cos(e5)*sin(e2)*sin(e3)*sin(e5)*sin(e6) - 2*de1*m6*x6*z6*cos(e2)*cos(e3)*cos(e4)*cos(e6)*sin(e2)*sin(e3)*sin(e4)*sin(e5) + 2*de1*m6*y6*z6*cos(e2)*cos(e3)*cos(e4)*sin(e2)*sin(e3)*sin(e4)*sin(e5)*sin(e6) - 2*de1*m6*y6*z6*cos(e2)*cos(e3)*cos(e4)^2*cos(e5)*cos(e6)*sin(e2)*sin(e3)*sin(e5) - 8*de1*m6*x6*y6*cos(e2)*cos(e3)*cos(e4)*cos(e5)*cos(e6)*sin(e2)*sin(e3)*sin(e4)*sin(e6),I6xy*de2*cos(e5)^2 - I6xy*de2*cos(e4)^2 - I6xy*de3*cos(e4)^2 + I6xy*de3*cos(e5)^2 - I6xy*de5*cos(e4) - I6xy*de2*cos(e4)^2*cos(e5)^2 + 2*I6xy*de2*cos(e4)^2*cos(e6)^2 - I6xy*de3*cos(e4)^2*cos(e5)^2 - 2*I6xy*de2*cos(e5)^2*cos(e6)^2 + 2*I6xy*de3*cos(e4)^2*cos(e6)^2 - 2*I6xy*de3*cos(e5)^2*cos(e6)^2 - (I6xx*de4*cos(e4)*sin(e5))/2 + (I6xx*de5*cos(e5)*sin(e4))/2 + (I6yy*de4*cos(e4)*sin(e5))/2 - (I6yy*de5*cos(e5)*sin(e4))/2 - I6yz*de4*cos(e6)*sin(e4) + (I6zz*de4*cos(e4)*sin(e5))/2 + (I6zz*de5*cos(e5)*sin(e4))/2 - I6zx*de4*sin(e4)*sin(e6) + 2*I6xy*de5*cos(e4)*cos(e6)^2 - de2*m6*x6*y6*cos(e4)^2 + de2*m6*x6*y6*cos(e5)^2 - de3*m6*x6*y6*cos(e4)^2 + de3*m6*x6*y6*cos(e5)^2 + (I6xx*de1*cos(e2)*cos(e3)*cos(e5))/2 - (I6yy*de1*cos(e2)*cos(e3)*cos(e5))/2 - (I6zz*de1*cos(e2)*cos(e3)*cos(e5))/2 + I6xx*de2*cos(e4)*cos(e5)*sin(e4) + I6xx*de3*cos(e4)*cos(e5)*sin(e4) - I6xx*de5*cos(e4)*cos(e6)*sin(e6) - I6yy*de2*cos(e4)*cos(e5)*sin(e4) - I6yy*de3*cos(e4)*cos(e5)*sin(e4) + I6yz*de2*cos(e5)*cos(e6)*sin(e5) + I6yz*de3*cos(e5)*cos(e6)*sin(e5) + I6yy*de5*cos(e4)*cos(e6)*sin(e6) + 2*I6xy*de2*cos(e4)^2*cos(e5)^2*cos(e6)^2 + 2*I6xy*de3*cos(e4)^2*cos(e5)^2*cos(e6)^2 - (I6xx*de1*cos(e5)*sin(e2)*sin(e3))/2 - I6xy*de4*cos(e5)*sin(e4)*sin(e5) + (I6yy*de1*cos(e5)*sin(e2)*sin(e3))/2 + (I6zz*de1*cos(e5)*sin(e2)*sin(e3))/2 + I6zx*de2*cos(e5)*sin(e5)*sin(e6) + I6zx*de3*cos(e5)*sin(e5)*sin(e6) - I6zx*de5*cos(e6)*sin(e4)*sin(e5) + I6yz*de5*sin(e4)*sin(e5)*sin(e6) + de4*m6*x6^2*cos(e4)*sin(e5) + de5*m6*y6^2*cos(e5)*sin(e4) - I6xx*de2*cos(e4)^2*cos(e6)*sin(e6) + I6xx*de2*cos(e5)^2*cos(e6)*sin(e6) - I6xx*de3*cos(e4)^2*cos(e6)*sin(e6) + I6xx*de4*cos(e4)*cos(e6)^2*sin(e5) + I6xx*de3*cos(e5)^2*cos(e6)*sin(e6) - I6xx*de5*cos(e5)*cos(e6)^2*sin(e4) + I6yy*de2*cos(e4)^2*cos(e6)*sin(e6) - I6yy*de2*cos(e5)^2*cos(e6)*sin(e6) + I6yy*de3*cos(e4)^2*cos(e6)*sin(e6) - I6yy*de4*cos(e4)*cos(e6)^2*sin(e5) - I6yy*de3*cos(e5)^2*cos(e6)*sin(e6) + I6yy*de5*cos(e5)*cos(e6)^2*sin(e4) + I6yz*de4*cos(e5)^2*cos(e6)*sin(e4) + I6zx*de4*cos(e5)^2*sin(e4)*sin(e6) - de5*m6*x6*y6*cos(e4) + 2*de5*m6*x6*y6*cos(e4)*cos(e6)^2 - I6xy*de1*cos(e2)*cos(e3)*cos(e4)*sin(e4) + (I6xx*de1*cos(e2)*cos(e4)*sin(e3)*sin(e5))/2 + (I6xx*de1*cos(e3)*cos(e4)*sin(e2)*sin(e5))/2 + 2*I6xy*de4*cos(e4)*cos(e6)*sin(e5)*sin(e6) - 2*I6xy*de5*cos(e5)*cos(e6)*sin(e4)*sin(e6) - (I6yy*de1*cos(e2)*cos(e4)*sin(e3)*sin(e5))/2 - (I6yy*de1*cos(e3)*cos(e4)*sin(e2)*sin(e5))/2 + (I6zz*de1*cos(e2)*cos(e4)*sin(e3)*sin(e5))/2 + (I6zz*de1*cos(e3)*cos(e4)*sin(e2)*sin(e5))/2 - I6zx*de2*cos(e4)*cos(e6)*sin(e4)*sin(e5) - I6zx*de3*cos(e4)*cos(e6)*sin(e4)*sin(e5) + I6xy*de1*cos(e4)*sin(e2)*sin(e3)*sin(e4) + I6yz*de2*cos(e4)*sin(e4)*sin(e5)*sin(e6) + I6yz*de3*cos(e4)*sin(e4)*sin(e5)*sin(e6) - de1*m6*x6^2*cos(e2)*cos(e3)*cos(e5) - de2*m6*x6^2*cos(e4)*cos(e5)*sin(e4) - de3*m6*x6^2*cos(e4)*cos(e5)*sin(e4) + de5*m6*x6^2*cos(e4)*cos(e6)*sin(e6) - de2*m6*x6*y6*cos(e4)^2*cos(e5)^2 + 2*de2*m6*x6*y6*cos(e4)^2*cos(e6)^2 - de3*m6*x6*y6*cos(e4)^2*cos(e5)^2 - 2*de2*m6*x6*y6*cos(e5)^2*cos(e6)^2 + 2*de3*m6*x6*y6*cos(e4)^2*cos(e6)^2 - 2*de3*m6*x6*y6*cos(e5)^2*cos(e6)^2 + de2*m6*y6^2*cos(e4)*cos(e5)*sin(e4) + de3*m6*y6^2*cos(e4)*cos(e5)*sin(e4) - de5*m6*y6^2*cos(e4)*cos(e6)*sin(e6) + de1*m6*x6^2*cos(e5)*sin(e2)*sin(e3) - I6xx*de1*cos(e2)*cos(e3)*cos(e4)^2*cos(e5) - I6xx*de1*cos(e2)*cos(e3)*cos(e5)*cos(e6)^2 + I6yy*de1*cos(e2)*cos(e3)*cos(e4)^2*cos(e5) + I6yy*de1*cos(e2)*cos(e3)*cos(e5)*cos(e6)^2 - 2*I6xx*de2*cos(e4)*cos(e5)*cos(e6)^2*sin(e4) - 2*I6xx*de3*cos(e4)*cos(e5)*cos(e6)^2*sin(e4) + 2*I6yy*de2*cos(e4)*cos(e5)*cos(e6)^2*sin(e4) + 2*I6yy*de3*cos(e4)*cos(e5)*cos(e6)^2*sin(e4) - I6yz*de2*cos(e4)^2*cos(e5)*cos(e6)*sin(e5) - I6yz*de3*cos(e4)^2*cos(e5)*cos(e6)*sin(e5) + a3*de2*m6*x6*cos(e6)*sin(e4) + a3*de3*m6*x6*cos(e6)*sin(e4) + I6xx*de1*cos(e4)^2*cos(e5)*sin(e2)*sin(e3) + I6xx*de1*cos(e5)*cos(e6)^2*sin(e2)*sin(e3) + 2*I6xy*de4*cos(e5)*cos(e6)^2*sin(e4)*sin(e5) - I6yy*de1*cos(e4)^2*cos(e5)*sin(e2)*sin(e3) - I6yy*de1*cos(e5)*cos(e6)^2*sin(e2)*sin(e3) - I6zx*de2*cos(e4)^2*cos(e5)*sin(e5)*sin(e6) - I6zx*de3*cos(e4)^2*cos(e5)*sin(e5)*sin(e6) + d4*de2*m6*y6*cos(e6)*sin(e5) + d4*de3*m6*y6*cos(e6)*sin(e5) - a3*de2*m6*y6*sin(e4)*sin(e6) - a3*de3*m6*y6*sin(e4)*sin(e6) + d4*de2*m6*x6*sin(e5)*sin(e6) + d4*de3*m6*x6*sin(e5)*sin(e6) - de4*m6*y6*z6*cos(e6)*sin(e4) + de2*m6*x6^2*cos(e4)^2*cos(e6)*sin(e6) - de2*m6*x6^2*cos(e5)^2*cos(e6)*sin(e6) + de3*m6*x6^2*cos(e4)^2*cos(e6)*sin(e6) - de4*m6*x6^2*cos(e4)*cos(e6)^2*sin(e5) - de3*m6*x6^2*cos(e5)^2*cos(e6)*sin(e6) + de5*m6*x6^2*cos(e5)*cos(e6)^2*sin(e4) - de2*m6*y6^2*cos(e4)^2*cos(e6)*sin(e6) + de2*m6*y6^2*cos(e5)^2*cos(e6)*sin(e6) - de3*m6*y6^2*cos(e4)^2*cos(e6)*sin(e6) + de4*m6*y6^2*cos(e4)*cos(e6)^2*sin(e5) + de3*m6*y6^2*cos(e5)^2*cos(e6)*sin(e6) - de5*m6*y6^2*cos(e5)*cos(e6)^2*sin(e4) - de4*m6*x6*z6*sin(e4)*sin(e6) - I6xx*de2*cos(e4)^2*cos(e5)^2*cos(e6)*sin(e6) - I6xx*de3*cos(e4)^2*cos(e5)^2*cos(e6)*sin(e6) + I6yy*de2*cos(e4)^2*cos(e5)^2*cos(e6)*sin(e6) + I6yy*de3*cos(e4)^2*cos(e5)^2*cos(e6)*sin(e6) - 2*I6xy*de1*cos(e2)*cos(e3)*cos(e5)*cos(e6)*sin(e6) + I6zx*de1*cos(e2)*cos(e4)*cos(e5)*cos(e6)*sin(e3) + I6zx*de1*cos(e3)*cos(e4)*cos(e5)*cos(e6)*sin(e2) - 4*I6xy*de2*cos(e4)*cos(e5)*cos(e6)*sin(e4)*sin(e6) - 4*I6xy*de3*cos(e4)*cos(e5)*cos(e6)*sin(e4)*sin(e6) - I6yz*de1*cos(e2)*cos(e4)*cos(e5)*sin(e3)*sin(e6) - I6yz*de1*cos(e3)*cos(e4)*cos(e5)*sin(e2)*sin(e6) + I6xy*de1*cos(e2)*cos(e5)*sin(e3)*sin(e4)*sin(e5) + I6xy*de1*cos(e3)*cos(e5)*sin(e2)*sin(e4)*sin(e5) + 2*I6xy*de1*cos(e5)*cos(e6)*sin(e2)*sin(e3)*sin(e6) - I6xx*de4*cos(e5)*cos(e6)*sin(e4)*sin(e5)*sin(e6) + I6yy*de4*cos(e5)*cos(e6)*sin(e4)*sin(e5)*sin(e6) + de1*m6*y6^2*cos(e2)*cos(e4)*sin(e3)*sin(e5) + de1*m6*y6^2*cos(e3)*cos(e4)*sin(e2)*sin(e5) - a2*de1*m6*x6*cos(e2)*cos(e4)*cos(e6) + a3*de2*m6*y6*cos(e4)*cos(e5)*cos(e6) + a3*de3*m6*y6*cos(e4)*cos(e5)*cos(e6) - I6xy*de1*cos(e2)*cos(e3)*cos(e4)*cos(e5)^2*sin(e4) + 2*I6xy*de1*cos(e2)*cos(e3)*cos(e4)*cos(e6)^2*sin(e4) + I6zx*de1*cos(e2)*cos(e3)*cos(e4)^2*cos(e6)*sin(e5) + a2*de2*m6*x6*cos(e3)*cos(e6)*sin(e4) + a3*de2*m6*x6*cos(e4)*cos(e5)*sin(e6) + a3*de3*m6*x6*cos(e4)*cos(e5)*sin(e6) + a2*de1*m6*y6*cos(e2)*cos(e4)*sin(e6) - I6xx*de1*cos(e2)*cos(e4)*cos(e6)^2*sin(e3)*sin(e5) - I6xx*de1*cos(e3)*cos(e4)*cos(e6)^2*sin(e2)*sin(e5) + I6yy*de1*cos(e2)*cos(e4)*cos(e6)^2*sin(e3)*sin(e5) + I6yy*de1*cos(e3)*cos(e4)*cos(e6)^2*sin(e2)*sin(e5) - I6yz*de1*cos(e2)*cos(e3)*cos(e4)^2*sin(e5)*sin(e6) - I6yz*de1*cos(e2)*cos(e5)^2*cos(e6)*sin(e3)*sin(e4) - I6yz*de1*cos(e3)*cos(e5)^2*cos(e6)*sin(e2)*sin(e4) - a2*de2*m6*y6*cos(e3)*sin(e4)*sin(e6) - a2*de2*m6*y6*cos(e6)*sin(e3)*sin(e5) + I6xy*de1*cos(e4)*cos(e5)^2*sin(e2)*sin(e3)*sin(e4) - 2*I6xy*de1*cos(e4)*cos(e6)^2*sin(e2)*sin(e3)*sin(e4) - I6zx*de1*cos(e2)*cos(e5)^2*sin(e3)*sin(e4)*sin(e6) - I6zx*de1*cos(e3)*cos(e5)^2*sin(e2)*sin(e4)*sin(e6) - I6zx*de1*cos(e4)^2*cos(e6)*sin(e2)*sin(e3)*sin(e5) + de1*m6*x6^2*cos(e2)*cos(e3)*cos(e4)^2*cos(e5) + de1*m6*x6^2*cos(e2)*cos(e3)*cos(e5)*cos(e6)^2 - de1*m6*y6^2*cos(e2)*cos(e3)*cos(e4)^2*cos(e5) - de1*m6*y6^2*cos(e2)*cos(e3)*cos(e5)*cos(e6)^2 + de2*m6*y6*z6*cos(e5)*cos(e6)*sin(e5) + de3*m6*y6*z6*cos(e5)*cos(e6)*sin(e5) - a2*de2*m6*x6*sin(e3)*sin(e5)*sin(e6) + I6yz*de1*cos(e4)^2*sin(e2)*sin(e3)*sin(e5)*sin(e6) + 2*de2*m6*x6^2*cos(e4)*cos(e5)*cos(e6)^2*sin(e4) + 2*de3*m6*x6^2*cos(e4)*cos(e5)*cos(e6)^2*sin(e4) + 2*de2*m6*x6*y6*cos(e4)^2*cos(e5)^2*cos(e6)^2 + 2*de3*m6*x6*y6*cos(e4)^2*cos(e5)^2*cos(e6)^2 - 2*de2*m6*y6^2*cos(e4)*cos(e5)*cos(e6)^2*sin(e4) - 2*de3*m6*y6^2*cos(e4)*cos(e5)*cos(e6)^2*sin(e4) - de4*m6*x6*y6*cos(e5)*sin(e4)*sin(e5) + de2*m6*x6*z6*cos(e5)*sin(e5)*sin(e6) + de3*m6*x6*z6*cos(e5)*sin(e5)*sin(e6) - de5*m6*x6*z6*cos(e6)*sin(e4)*sin(e5) - de1*m6*x6^2*cos(e4)^2*cos(e5)*sin(e2)*sin(e3) - de1*m6*x6^2*cos(e5)*cos(e6)^2*sin(e2)*sin(e3) + de1*m6*y6^2*cos(e4)^2*cos(e5)*sin(e2)*sin(e3) + de1*m6*y6^2*cos(e5)*cos(e6)^2*sin(e2)*sin(e3) + de5*m6*y6*z6*sin(e4)*sin(e5)*sin(e6) + 2*I6xx*de1*cos(e2)*cos(e3)*cos(e4)^2*cos(e5)*cos(e6)^2 - 2*I6yy*de1*cos(e2)*cos(e3)*cos(e4)^2*cos(e5)*cos(e6)^2 - 2*I6xx*de1*cos(e4)^2*cos(e5)*cos(e6)^2*sin(e2)*sin(e3) + 2*I6yy*de1*cos(e4)^2*cos(e5)*cos(e6)^2*sin(e2)*sin(e3) + de4*m6*y6*z6*cos(e5)^2*cos(e6)*sin(e4) + de2*m6*x6^2*cos(e4)^2*cos(e5)^2*cos(e6)*sin(e6) + de3*m6*x6^2*cos(e4)^2*cos(e5)^2*cos(e6)*sin(e6) - de2*m6*y6^2*cos(e4)^2*cos(e5)^2*cos(e6)*sin(e6) - de3*m6*y6^2*cos(e4)^2*cos(e5)^2*cos(e6)*sin(e6) + de4*m6*x6*z6*cos(e5)^2*sin(e4)*sin(e6) + de4*m6*x6^2*cos(e5)*cos(e6)*sin(e4)*sin(e5)*sin(e6) - de4*m6*y6^2*cos(e5)*cos(e6)*sin(e4)*sin(e5)*sin(e6) - a3*de1*m6*x6*cos(e2)*cos(e3)*cos(e4)*cos(e6) + a2*de2*m6*y6*cos(e3)*cos(e4)*cos(e5)*cos(e6) + 4*I6xy*de1*cos(e2)*cos(e3)*cos(e4)^2*cos(e5)*cos(e6)*sin(e6) + a2*de2*m6*x6*cos(e3)*cos(e4)*cos(e5)*sin(e6) + a3*de1*m6*y6*cos(e2)*cos(e3)*cos(e4)*sin(e6) + a2*de1*m6*y6*cos(e2)*cos(e5)*cos(e6)*sin(e4) + d4*de1*m6*x6*cos(e2)*cos(e4)*cos(e6)*sin(e3) + d4*de1*m6*x6*cos(e3)*cos(e4)*cos(e6)*sin(e2) + a3*de1*m6*x6*cos(e4)*cos(e6)*sin(e2)*sin(e3) + a2*de1*m6*x6*cos(e2)*cos(e5)*sin(e4)*sin(e6) - 2*I6xy*de1*cos(e2)*cos(e5)*cos(e6)^2*sin(e3)*sin(e4)*sin(e5) - 2*I6xy*de1*cos(e3)*cos(e5)*cos(e6)^2*sin(e2)*sin(e4)*sin(e5) - 4*I6xy*de1*cos(e4)^2*cos(e5)*cos(e6)*sin(e2)*sin(e3)*sin(e6) - d4*de1*m6*y6*cos(e2)*cos(e4)*sin(e3)*sin(e6) - d4*de1*m6*y6*cos(e3)*cos(e4)*sin(e2)*sin(e6) - de1*m6*x6*y6*cos(e2)*cos(e3)*cos(e4)*sin(e4) - a3*de1*m6*y6*cos(e4)*sin(e2)*sin(e3)*sin(e6) + 2*de4*m6*x6*y6*cos(e4)*cos(e6)*sin(e5)*sin(e6) - 2*de5*m6*x6*y6*cos(e5)*cos(e6)*sin(e4)*sin(e6) - de2*m6*x6*z6*cos(e4)*cos(e6)*sin(e4)*sin(e5) - de3*m6*x6*z6*cos(e4)*cos(e6)*sin(e4)*sin(e5) + de1*m6*x6^2*cos(e2)*cos(e4)*cos(e6)^2*sin(e3)*sin(e5) + de1*m6*x6^2*cos(e3)*cos(e4)*cos(e6)^2*sin(e2)*sin(e5) - de1*m6*y6^2*cos(e2)*cos(e4)*cos(e6)^2*sin(e3)*sin(e5) - de1*m6*y6^2*cos(e3)*cos(e4)*cos(e6)^2*sin(e2)*sin(e5) + de1*m6*x6*y6*cos(e4)*sin(e2)*sin(e3)*sin(e4) + de2*m6*y6*z6*cos(e4)*sin(e4)*sin(e5)*sin(e6) + de3*m6*y6*z6*cos(e4)*sin(e4)*sin(e5)*sin(e6) + 2*I6xy*de1*cos(e2)*cos(e3)*cos(e4)*cos(e5)^2*cos(e6)^2*sin(e4) - 2*I6xy*de1*cos(e4)*cos(e5)^2*cos(e6)^2*sin(e2)*sin(e3)*sin(e4) - 2*de1*m6*x6^2*cos(e2)*cos(e3)*cos(e4)^2*cos(e5)*cos(e6)^2 + 2*de1*m6*y6^2*cos(e2)*cos(e3)*cos(e4)^2*cos(e5)*cos(e6)^2 - de2*m6*y6*z6*cos(e4)^2*cos(e5)*cos(e6)*sin(e5) - de3*m6*y6*z6*cos(e4)^2*cos(e5)*cos(e6)*sin(e5) + 2*de4*m6*x6*y6*cos(e5)*cos(e6)^2*sin(e4)*sin(e5) - de2*m6*x6*z6*cos(e4)^2*cos(e5)*sin(e5)*sin(e6) - de3*m6*x6*z6*cos(e4)^2*cos(e5)*sin(e5)*sin(e6) + 2*de1*m6*x6^2*cos(e4)^2*cos(e5)*cos(e6)^2*sin(e2)*sin(e3) - 2*de1*m6*y6^2*cos(e4)^2*cos(e5)*cos(e6)^2*sin(e2)*sin(e3) - I6xx*de1*cos(e2)*cos(e3)*cos(e4)*cos(e6)*sin(e4)*sin(e6) + I6yy*de1*cos(e2)*cos(e3)*cos(e4)*cos(e6)*sin(e4)*sin(e6) - 2*I6xy*de1*cos(e2)*cos(e4)*cos(e6)*sin(e3)*sin(e5)*sin(e6) - 2*I6xy*de1*cos(e3)*cos(e4)*cos(e6)*sin(e2)*sin(e5)*sin(e6) + I6xx*de1*cos(e4)*cos(e6)*sin(e2)*sin(e3)*sin(e4)*sin(e6) - I6yy*de1*cos(e4)*cos(e6)*sin(e2)*sin(e3)*sin(e4)*sin(e6) + a3*de1*m6*y6*cos(e2)*cos(e3)*cos(e5)*cos(e6)*sin(e4) - I6xx*de1*cos(e2)*cos(e3)*cos(e4)*cos(e5)^2*cos(e6)*sin(e4)*sin(e6) + I6yy*de1*cos(e2)*cos(e3)*cos(e4)*cos(e5)^2*cos(e6)*sin(e4)*sin(e6) + a3*de1*m6*x6*cos(e2)*cos(e3)*cos(e5)*sin(e4)*sin(e6) - d4*de1*m6*y6*cos(e2)*cos(e5)*cos(e6)*sin(e3)*sin(e4) - d4*de1*m6*y6*cos(e3)*cos(e5)*cos(e6)*sin(e2)*sin(e4) - 2*de1*m6*x6*y6*cos(e2)*cos(e3)*cos(e5)*cos(e6)*sin(e6) + de1*m6*x6*z6*cos(e2)*cos(e4)*cos(e5)*cos(e6)*sin(e3) + de1*m6*x6*z6*cos(e3)*cos(e4)*cos(e5)*cos(e6)*sin(e2) - a3*de1*m6*y6*cos(e5)*cos(e6)*sin(e2)*sin(e3)*sin(e4) - d4*de1*m6*x6*cos(e2)*cos(e5)*sin(e3)*sin(e4)*sin(e6) - d4*de1*m6*x6*cos(e3)*cos(e5)*sin(e2)*sin(e4)*sin(e6) + I6xx*de1*cos(e4)*cos(e5)^2*cos(e6)*sin(e2)*sin(e3)*sin(e4)*sin(e6) - I6yy*de1*cos(e4)*cos(e5)^2*cos(e6)*sin(e2)*sin(e3)*sin(e4)*sin(e6) - 4*de2*m6*x6*y6*cos(e4)*cos(e5)*cos(e6)*sin(e4)*sin(e6) - 4*de3*m6*x6*y6*cos(e4)*cos(e5)*cos(e6)*sin(e4)*sin(e6) - de1*m6*y6*z6*cos(e2)*cos(e4)*cos(e5)*sin(e3)*sin(e6) - de1*m6*y6*z6*cos(e3)*cos(e4)*cos(e5)*sin(e2)*sin(e6) - a3*de1*m6*x6*cos(e5)*sin(e2)*sin(e3)*sin(e4)*sin(e6) + de1*m6*x6*y6*cos(e2)*cos(e5)*sin(e3)*sin(e4)*sin(e5) + de1*m6*x6*y6*cos(e3)*cos(e5)*sin(e2)*sin(e4)*sin(e5) + 2*de1*m6*x6*y6*cos(e5)*cos(e6)*sin(e2)*sin(e3)*sin(e6) - de1*m6*x6*y6*cos(e2)*cos(e3)*cos(e4)*cos(e5)^2*sin(e4) + 2*de1*m6*x6*y6*cos(e2)*cos(e3)*cos(e4)*cos(e6)^2*sin(e4) + de1*m6*x6*z6*cos(e2)*cos(e3)*cos(e4)^2*cos(e6)*sin(e5) - de1*m6*y6*z6*cos(e2)*cos(e3)*cos(e4)^2*sin(e5)*sin(e6) - de1*m6*y6*z6*cos(e2)*cos(e5)^2*cos(e6)*sin(e3)*sin(e4) - de1*m6*y6*z6*cos(e3)*cos(e5)^2*cos(e6)*sin(e2)*sin(e4) + de1*m6*x6*y6*cos(e4)*cos(e5)^2*sin(e2)*sin(e3)*sin(e4) - 2*de1*m6*x6*y6*cos(e4)*cos(e6)^2*sin(e2)*sin(e3)*sin(e4) - de1*m6*x6*z6*cos(e2)*cos(e5)^2*sin(e3)*sin(e4)*sin(e6) - de1*m6*x6*z6*cos(e3)*cos(e5)^2*sin(e2)*sin(e4)*sin(e6) - de1*m6*x6*z6*cos(e4)^2*cos(e6)*sin(e2)*sin(e3)*sin(e5) - I6yz*de1*cos(e2)*cos(e3)*cos(e4)*cos(e5)*cos(e6)*sin(e4)*sin(e5) + de1*m6*y6*z6*cos(e4)^2*sin(e2)*sin(e3)*sin(e5)*sin(e6) - I6zx*de1*cos(e2)*cos(e3)*cos(e4)*cos(e5)*sin(e4)*sin(e5)*sin(e6) + I6xx*de1*cos(e2)*cos(e5)*cos(e6)*sin(e3)*sin(e4)*sin(e5)*sin(e6) + I6xx*de1*cos(e3)*cos(e5)*cos(e6)*sin(e2)*sin(e4)*sin(e5)*sin(e6) + I6yz*de1*cos(e4)*cos(e5)*cos(e6)*sin(e2)*sin(e3)*sin(e4)*sin(e5) - I6yy*de1*cos(e2)*cos(e5)*cos(e6)*sin(e3)*sin(e4)*sin(e5)*sin(e6) - I6yy*de1*cos(e3)*cos(e5)*cos(e6)*sin(e2)*sin(e4)*sin(e5)*sin(e6) + I6zx*de1*cos(e4)*cos(e5)*sin(e2)*sin(e3)*sin(e4)*sin(e5)*sin(e6) + de1*m6*x6^2*cos(e2)*cos(e3)*cos(e4)*cos(e6)*sin(e4)*sin(e6) - de1*m6*y6^2*cos(e2)*cos(e3)*cos(e4)*cos(e6)*sin(e4)*sin(e6) - de1*m6*x6^2*cos(e4)*cos(e6)*sin(e2)*sin(e3)*sin(e4)*sin(e6) + de1*m6*y6^2*cos(e4)*cos(e6)*sin(e2)*sin(e3)*sin(e4)*sin(e6) + de1*m6*x6^2*cos(e2)*cos(e3)*cos(e4)*cos(e5)^2*cos(e6)*sin(e4)*sin(e6) - de1*m6*y6^2*cos(e2)*cos(e3)*cos(e4)*cos(e5)^2*cos(e6)*sin(e4)*sin(e6) - 2*de1*m6*x6*y6*cos(e2)*cos(e4)*cos(e6)*sin(e3)*sin(e5)*sin(e6) - 2*de1*m6*x6*y6*cos(e3)*cos(e4)*cos(e6)*sin(e2)*sin(e5)*sin(e6) - de1*m6*x6^2*cos(e4)*cos(e5)^2*cos(e6)*sin(e2)*sin(e3)*sin(e4)*sin(e6) + de1*m6*y6^2*cos(e4)*cos(e5)^2*cos(e6)*sin(e2)*sin(e3)*sin(e4)*sin(e6) + 4*de1*m6*x6*y6*cos(e2)*cos(e3)*cos(e4)^2*cos(e5)*cos(e6)*sin(e6) - 2*de1*m6*x6*y6*cos(e2)*cos(e5)*cos(e6)^2*sin(e3)*sin(e4)*sin(e5) - 2*de1*m6*x6*y6*cos(e3)*cos(e5)*cos(e6)^2*sin(e2)*sin(e4)*sin(e5) - 4*de1*m6*x6*y6*cos(e4)^2*cos(e5)*cos(e6)*sin(e2)*sin(e3)*sin(e6) + 2*de1*m6*x6*y6*cos(e2)*cos(e3)*cos(e4)*cos(e5)^2*cos(e6)^2*sin(e4) - de1*m6*x6^2*cos(e2)*cos(e5)*cos(e6)*sin(e3)*sin(e4)*sin(e5)*sin(e6) - de1*m6*x6^2*cos(e3)*cos(e5)*cos(e6)*sin(e2)*sin(e4)*sin(e5)*sin(e6) - 2*de1*m6*x6*y6*cos(e4)*cos(e5)^2*cos(e6)^2*sin(e2)*sin(e3)*sin(e4) + de1*m6*y6^2*cos(e2)*cos(e5)*cos(e6)*sin(e3)*sin(e4)*sin(e5)*sin(e6) + de1*m6*y6^2*cos(e3)*cos(e5)*cos(e6)*sin(e2)*sin(e4)*sin(e5)*sin(e6) - de1*m6*y6*z6*cos(e2)*cos(e3)*cos(e4)*cos(e5)*cos(e6)*sin(e4)*sin(e5) - de1*m6*x6*z6*cos(e2)*cos(e3)*cos(e4)*cos(e5)*sin(e4)*sin(e5)*sin(e6) + de1*m6*y6*z6*cos(e4)*cos(e5)*cos(e6)*sin(e2)*sin(e3)*sin(e4)*sin(e5) + de1*m6*x6*z6*cos(e4)*cos(e5)*sin(e2)*sin(e3)*sin(e4)*sin(e5)*sin(e6),I6xy*de2*cos(e5)^2 - I6xy*de2*cos(e4)^2 - I6xy*de3*cos(e4)^2 + I6xy*de3*cos(e5)^2 - I6xy*de5*cos(e4) - I6xy*de2*cos(e4)^2*cos(e5)^2 + 2*I6xy*de2*cos(e4)^2*cos(e6)^2 - I6xy*de3*cos(e4)^2*cos(e5)^2 - 2*I6xy*de2*cos(e5)^2*cos(e6)^2 + 2*I6xy*de3*cos(e4)^2*cos(e6)^2 - 2*I6xy*de3*cos(e5)^2*cos(e6)^2 - (I6xx*de4*cos(e4)*sin(e5))/2 + (I6xx*de5*cos(e5)*sin(e4))/2 + (I6yy*de4*cos(e4)*sin(e5))/2 - (I6yy*de5*cos(e5)*sin(e4))/2 - I6yz*de4*cos(e6)*sin(e4) + (I6zz*de4*cos(e4)*sin(e5))/2 + (I6zz*de5*cos(e5)*sin(e4))/2 - I6zx*de4*sin(e4)*sin(e6) + 2*I6xy*de5*cos(e4)*cos(e6)^2 - de2*m6*x6*y6*cos(e4)^2 + de2*m6*x6*y6*cos(e5)^2 - de3*m6*x6*y6*cos(e4)^2 + de3*m6*x6*y6*cos(e5)^2 + (I6xx*de1*cos(e2)*cos(e3)*cos(e5))/2 - (I6yy*de1*cos(e2)*cos(e3)*cos(e5))/2 - (I6zz*de1*cos(e2)*cos(e3)*cos(e5))/2 + I6xx*de2*cos(e4)*cos(e5)*sin(e4) + I6xx*de3*cos(e4)*cos(e5)*sin(e4) - I6xx*de5*cos(e4)*cos(e6)*sin(e6) - I6yy*de2*cos(e4)*cos(e5)*sin(e4) - I6yy*de3*cos(e4)*cos(e5)*sin(e4) + I6yz*de2*cos(e5)*cos(e6)*sin(e5) + I6yz*de3*cos(e5)*cos(e6)*sin(e5) + I6yy*de5*cos(e4)*cos(e6)*sin(e6) + 2*I6xy*de2*cos(e4)^2*cos(e5)^2*cos(e6)^2 + 2*I6xy*de3*cos(e4)^2*cos(e5)^2*cos(e6)^2 - (I6xx*de1*cos(e5)*sin(e2)*sin(e3))/2 - I6xy*de4*cos(e5)*sin(e4)*sin(e5) + (I6yy*de1*cos(e5)*sin(e2)*sin(e3))/2 + (I6zz*de1*cos(e5)*sin(e2)*sin(e3))/2 + I6zx*de2*cos(e5)*sin(e5)*sin(e6) + I6zx*de3*cos(e5)*sin(e5)*sin(e6) - I6zx*de5*cos(e6)*sin(e4)*sin(e5) + I6yz*de5*sin(e4)*sin(e5)*sin(e6) + de4*m6*x6^2*cos(e4)*sin(e5) + de5*m6*y6^2*cos(e5)*sin(e4) - I6xx*de2*cos(e4)^2*cos(e6)*sin(e6) + I6xx*de2*cos(e5)^2*cos(e6)*sin(e6) - I6xx*de3*cos(e4)^2*cos(e6)*sin(e6) + I6xx*de4*cos(e4)*cos(e6)^2*sin(e5) + I6xx*de3*cos(e5)^2*cos(e6)*sin(e6) - I6xx*de5*cos(e5)*cos(e6)^2*sin(e4) + I6yy*de2*cos(e4)^2*cos(e6)*sin(e6) - I6yy*de2*cos(e5)^2*cos(e6)*sin(e6) + I6yy*de3*cos(e4)^2*cos(e6)*sin(e6) - I6yy*de4*cos(e4)*cos(e6)^2*sin(e5) - I6yy*de3*cos(e5)^2*cos(e6)*sin(e6) + I6yy*de5*cos(e5)*cos(e6)^2*sin(e4) + I6yz*de4*cos(e5)^2*cos(e6)*sin(e4) + I6zx*de4*cos(e5)^2*sin(e4)*sin(e6) - de5*m6*x6*y6*cos(e4) + 2*de5*m6*x6*y6*cos(e4)*cos(e6)^2 - I6xy*de1*cos(e2)*cos(e3)*cos(e4)*sin(e4) + (I6xx*de1*cos(e2)*cos(e4)*sin(e3)*sin(e5))/2 + (I6xx*de1*cos(e3)*cos(e4)*sin(e2)*sin(e5))/2 + 2*I6xy*de4*cos(e4)*cos(e6)*sin(e5)*sin(e6) - 2*I6xy*de5*cos(e5)*cos(e6)*sin(e4)*sin(e6) - (I6yy*de1*cos(e2)*cos(e4)*sin(e3)*sin(e5))/2 - (I6yy*de1*cos(e3)*cos(e4)*sin(e2)*sin(e5))/2 + (I6zz*de1*cos(e2)*cos(e4)*sin(e3)*sin(e5))/2 + (I6zz*de1*cos(e3)*cos(e4)*sin(e2)*sin(e5))/2 - I6zx*de2*cos(e4)*cos(e6)*sin(e4)*sin(e5) - I6zx*de3*cos(e4)*cos(e6)*sin(e4)*sin(e5) + I6xy*de1*cos(e4)*sin(e2)*sin(e3)*sin(e4) + I6yz*de2*cos(e4)*sin(e4)*sin(e5)*sin(e6) + I6yz*de3*cos(e4)*sin(e4)*sin(e5)*sin(e6) - de1*m6*x6^2*cos(e2)*cos(e3)*cos(e5) - de2*m6*x6^2*cos(e4)*cos(e5)*sin(e4) - de3*m6*x6^2*cos(e4)*cos(e5)*sin(e4) + de5*m6*x6^2*cos(e4)*cos(e6)*sin(e6) - de2*m6*x6*y6*cos(e4)^2*cos(e5)^2 + 2*de2*m6*x6*y6*cos(e4)^2*cos(e6)^2 - de3*m6*x6*y6*cos(e4)^2*cos(e5)^2 - 2*de2*m6*x6*y6*cos(e5)^2*cos(e6)^2 + 2*de3*m6*x6*y6*cos(e4)^2*cos(e6)^2 - 2*de3*m6*x6*y6*cos(e5)^2*cos(e6)^2 + de2*m6*y6^2*cos(e4)*cos(e5)*sin(e4) + de3*m6*y6^2*cos(e4)*cos(e5)*sin(e4) - de5*m6*y6^2*cos(e4)*cos(e6)*sin(e6) + de1*m6*x6^2*cos(e5)*sin(e2)*sin(e3) - I6xx*de1*cos(e2)*cos(e3)*cos(e4)^2*cos(e5) - I6xx*de1*cos(e2)*cos(e3)*cos(e5)*cos(e6)^2 + I6yy*de1*cos(e2)*cos(e3)*cos(e4)^2*cos(e5) + I6yy*de1*cos(e2)*cos(e3)*cos(e5)*cos(e6)^2 - 2*I6xx*de2*cos(e4)*cos(e5)*cos(e6)^2*sin(e4) - 2*I6xx*de3*cos(e4)*cos(e5)*cos(e6)^2*sin(e4) + 2*I6yy*de2*cos(e4)*cos(e5)*cos(e6)^2*sin(e4) + 2*I6yy*de3*cos(e4)*cos(e5)*cos(e6)^2*sin(e4) - I6yz*de2*cos(e4)^2*cos(e5)*cos(e6)*sin(e5) - I6yz*de3*cos(e4)^2*cos(e5)*cos(e6)*sin(e5) + a3*de2*m6*x6*cos(e6)*sin(e4) + a3*de3*m6*x6*cos(e6)*sin(e4) + I6xx*de1*cos(e4)^2*cos(e5)*sin(e2)*sin(e3) + I6xx*de1*cos(e5)*cos(e6)^2*sin(e2)*sin(e3) + 2*I6xy*de4*cos(e5)*cos(e6)^2*sin(e4)*sin(e5) - I6yy*de1*cos(e4)^2*cos(e5)*sin(e2)*sin(e3) - I6yy*de1*cos(e5)*cos(e6)^2*sin(e2)*sin(e3) - I6zx*de2*cos(e4)^2*cos(e5)*sin(e5)*sin(e6) - I6zx*de3*cos(e4)^2*cos(e5)*sin(e5)*sin(e6) + d4*de2*m6*y6*cos(e6)*sin(e5) + d4*de3*m6*y6*cos(e6)*sin(e5) - a3*de2*m6*y6*sin(e4)*sin(e6) - a3*de3*m6*y6*sin(e4)*sin(e6) + d4*de2*m6*x6*sin(e5)*sin(e6) + d4*de3*m6*x6*sin(e5)*sin(e6) - de4*m6*y6*z6*cos(e6)*sin(e4) + de2*m6*x6^2*cos(e4)^2*cos(e6)*sin(e6) - de2*m6*x6^2*cos(e5)^2*cos(e6)*sin(e6) + de3*m6*x6^2*cos(e4)^2*cos(e6)*sin(e6) - de4*m6*x6^2*cos(e4)*cos(e6)^2*sin(e5) - de3*m6*x6^2*cos(e5)^2*cos(e6)*sin(e6) + de5*m6*x6^2*cos(e5)*cos(e6)^2*sin(e4) - de2*m6*y6^2*cos(e4)^2*cos(e6)*sin(e6) + de2*m6*y6^2*cos(e5)^2*cos(e6)*sin(e6) - de3*m6*y6^2*cos(e4)^2*cos(e6)*sin(e6) + de4*m6*y6^2*cos(e4)*cos(e6)^2*sin(e5) + de3*m6*y6^2*cos(e5)^2*cos(e6)*sin(e6) - de5*m6*y6^2*cos(e5)*cos(e6)^2*sin(e4) - de4*m6*x6*z6*sin(e4)*sin(e6) - I6xx*de2*cos(e4)^2*cos(e5)^2*cos(e6)*sin(e6) - I6xx*de3*cos(e4)^2*cos(e5)^2*cos(e6)*sin(e6) + I6yy*de2*cos(e4)^2*cos(e5)^2*cos(e6)*sin(e6) + I6yy*de3*cos(e4)^2*cos(e5)^2*cos(e6)*sin(e6) - 2*I6xy*de1*cos(e2)*cos(e3)*cos(e5)*cos(e6)*sin(e6) + I6zx*de1*cos(e2)*cos(e4)*cos(e5)*cos(e6)*sin(e3) + I6zx*de1*cos(e3)*cos(e4)*cos(e5)*cos(e6)*sin(e2) - 4*I6xy*de2*cos(e4)*cos(e5)*cos(e6)*sin(e4)*sin(e6) - 4*I6xy*de3*cos(e4)*cos(e5)*cos(e6)*sin(e4)*sin(e6) - I6yz*de1*cos(e2)*cos(e4)*cos(e5)*sin(e3)*sin(e6) - I6yz*de1*cos(e3)*cos(e4)*cos(e5)*sin(e2)*sin(e6) + I6xy*de1*cos(e2)*cos(e5)*sin(e3)*sin(e4)*sin(e5) + I6xy*de1*cos(e3)*cos(e5)*sin(e2)*sin(e4)*sin(e5) + 2*I6xy*de1*cos(e5)*cos(e6)*sin(e2)*sin(e3)*sin(e6) - I6xx*de4*cos(e5)*cos(e6)*sin(e4)*sin(e5)*sin(e6) + I6yy*de4*cos(e5)*cos(e6)*sin(e4)*sin(e5)*sin(e6) + de1*m6*y6^2*cos(e2)*cos(e4)*sin(e3)*sin(e5) + de1*m6*y6^2*cos(e3)*cos(e4)*sin(e2)*sin(e5) + a3*de2*m6*y6*cos(e4)*cos(e5)*cos(e6) + a3*de3*m6*y6*cos(e4)*cos(e5)*cos(e6) - I6xy*de1*cos(e2)*cos(e3)*cos(e4)*cos(e5)^2*sin(e4) + 2*I6xy*de1*cos(e2)*cos(e3)*cos(e4)*cos(e6)^2*sin(e4) + I6zx*de1*cos(e2)*cos(e3)*cos(e4)^2*cos(e6)*sin(e5) + a3*de2*m6*x6*cos(e4)*cos(e5)*sin(e6) + a3*de3*m6*x6*cos(e4)*cos(e5)*sin(e6) - I6xx*de1*cos(e2)*cos(e4)*cos(e6)^2*sin(e3)*sin(e5) - I6xx*de1*cos(e3)*cos(e4)*cos(e6)^2*sin(e2)*sin(e5) + I6yy*de1*cos(e2)*cos(e4)*cos(e6)^2*sin(e3)*sin(e5) + I6yy*de1*cos(e3)*cos(e4)*cos(e6)^2*sin(e2)*sin(e5) - I6yz*de1*cos(e2)*cos(e3)*cos(e4)^2*sin(e5)*sin(e6) - I6yz*de1*cos(e2)*cos(e5)^2*cos(e6)*sin(e3)*sin(e4) - I6yz*de1*cos(e3)*cos(e5)^2*cos(e6)*sin(e2)*sin(e4) + I6xy*de1*cos(e4)*cos(e5)^2*sin(e2)*sin(e3)*sin(e4) - 2*I6xy*de1*cos(e4)*cos(e6)^2*sin(e2)*sin(e3)*sin(e4) - I6zx*de1*cos(e2)*cos(e5)^2*sin(e3)*sin(e4)*sin(e6) - I6zx*de1*cos(e3)*cos(e5)^2*sin(e2)*sin(e4)*sin(e6) - I6zx*de1*cos(e4)^2*cos(e6)*sin(e2)*sin(e3)*sin(e5) + de1*m6*x6^2*cos(e2)*cos(e3)*cos(e4)^2*cos(e5) + de1*m6*x6^2*cos(e2)*cos(e3)*cos(e5)*cos(e6)^2 - de1*m6*y6^2*cos(e2)*cos(e3)*cos(e4)^2*cos(e5) - de1*m6*y6^2*cos(e2)*cos(e3)*cos(e5)*cos(e6)^2 + de2*m6*y6*z6*cos(e5)*cos(e6)*sin(e5) + de3*m6*y6*z6*cos(e5)*cos(e6)*sin(e5) + I6yz*de1*cos(e4)^2*sin(e2)*sin(e3)*sin(e5)*sin(e6) + 2*de2*m6*x6^2*cos(e4)*cos(e5)*cos(e6)^2*sin(e4) + 2*de3*m6*x6^2*cos(e4)*cos(e5)*cos(e6)^2*sin(e4) + 2*de2*m6*x6*y6*cos(e4)^2*cos(e5)^2*cos(e6)^2 + 2*de3*m6*x6*y6*cos(e4)^2*cos(e5)^2*cos(e6)^2 - 2*de2*m6*y6^2*cos(e4)*cos(e5)*cos(e6)^2*sin(e4) - 2*de3*m6*y6^2*cos(e4)*cos(e5)*cos(e6)^2*sin(e4) - de4*m6*x6*y6*cos(e5)*sin(e4)*sin(e5) + de2*m6*x6*z6*cos(e5)*sin(e5)*sin(e6) + de3*m6*x6*z6*cos(e5)*sin(e5)*sin(e6) - de5*m6*x6*z6*cos(e6)*sin(e4)*sin(e5) - de1*m6*x6^2*cos(e4)^2*cos(e5)*sin(e2)*sin(e3) - de1*m6*x6^2*cos(e5)*cos(e6)^2*sin(e2)*sin(e3) + de1*m6*y6^2*cos(e4)^2*cos(e5)*sin(e2)*sin(e3) + de1*m6*y6^2*cos(e5)*cos(e6)^2*sin(e2)*sin(e3) + de5*m6*y6*z6*sin(e4)*sin(e5)*sin(e6) + 2*I6xx*de1*cos(e2)*cos(e3)*cos(e4)^2*cos(e5)*cos(e6)^2 - 2*I6yy*de1*cos(e2)*cos(e3)*cos(e4)^2*cos(e5)*cos(e6)^2 - 2*I6xx*de1*cos(e4)^2*cos(e5)*cos(e6)^2*sin(e2)*sin(e3) + 2*I6yy*de1*cos(e4)^2*cos(e5)*cos(e6)^2*sin(e2)*sin(e3) + de4*m6*y6*z6*cos(e5)^2*cos(e6)*sin(e4) + de2*m6*x6^2*cos(e4)^2*cos(e5)^2*cos(e6)*sin(e6) + de3*m6*x6^2*cos(e4)^2*cos(e5)^2*cos(e6)*sin(e6) - de2*m6*y6^2*cos(e4)^2*cos(e5)^2*cos(e6)*sin(e6) - de3*m6*y6^2*cos(e4)^2*cos(e5)^2*cos(e6)*sin(e6) + de4*m6*x6*z6*cos(e5)^2*sin(e4)*sin(e6) + de4*m6*x6^2*cos(e5)*cos(e6)*sin(e4)*sin(e5)*sin(e6) - de4*m6*y6^2*cos(e5)*cos(e6)*sin(e4)*sin(e5)*sin(e6) - a3*de1*m6*x6*cos(e2)*cos(e3)*cos(e4)*cos(e6) + 4*I6xy*de1*cos(e2)*cos(e3)*cos(e4)^2*cos(e5)*cos(e6)*sin(e6) + a3*de1*m6*y6*cos(e2)*cos(e3)*cos(e4)*sin(e6) + d4*de1*m6*x6*cos(e2)*cos(e4)*cos(e6)*sin(e3) + d4*de1*m6*x6*cos(e3)*cos(e4)*cos(e6)*sin(e2) + a3*de1*m6*x6*cos(e4)*cos(e6)*sin(e2)*sin(e3) - 2*I6xy*de1*cos(e2)*cos(e5)*cos(e6)^2*sin(e3)*sin(e4)*sin(e5) - 2*I6xy*de1*cos(e3)*cos(e5)*cos(e6)^2*sin(e2)*sin(e4)*sin(e5) - 4*I6xy*de1*cos(e4)^2*cos(e5)*cos(e6)*sin(e2)*sin(e3)*sin(e6) - d4*de1*m6*y6*cos(e2)*cos(e4)*sin(e3)*sin(e6) - d4*de1*m6*y6*cos(e3)*cos(e4)*sin(e2)*sin(e6) - de1*m6*x6*y6*cos(e2)*cos(e3)*cos(e4)*sin(e4) - a3*de1*m6*y6*cos(e4)*sin(e2)*sin(e3)*sin(e6) + 2*de4*m6*x6*y6*cos(e4)*cos(e6)*sin(e5)*sin(e6) - 2*de5*m6*x6*y6*cos(e5)*cos(e6)*sin(e4)*sin(e6) - de2*m6*x6*z6*cos(e4)*cos(e6)*sin(e4)*sin(e5) - de3*m6*x6*z6*cos(e4)*cos(e6)*sin(e4)*sin(e5) + de1*m6*x6^2*cos(e2)*cos(e4)*cos(e6)^2*sin(e3)*sin(e5) + de1*m6*x6^2*cos(e3)*cos(e4)*cos(e6)^2*sin(e2)*sin(e5) - de1*m6*y6^2*cos(e2)*cos(e4)*cos(e6)^2*sin(e3)*sin(e5) - de1*m6*y6^2*cos(e3)*cos(e4)*cos(e6)^2*sin(e2)*sin(e5) + de1*m6*x6*y6*cos(e4)*sin(e2)*sin(e3)*sin(e4) + de2*m6*y6*z6*cos(e4)*sin(e4)*sin(e5)*sin(e6) + de3*m6*y6*z6*cos(e4)*sin(e4)*sin(e5)*sin(e6) + 2*I6xy*de1*cos(e2)*cos(e3)*cos(e4)*cos(e5)^2*cos(e6)^2*sin(e4) - 2*I6xy*de1*cos(e4)*cos(e5)^2*cos(e6)^2*sin(e2)*sin(e3)*sin(e4) - 2*de1*m6*x6^2*cos(e2)*cos(e3)*cos(e4)^2*cos(e5)*cos(e6)^2 + 2*de1*m6*y6^2*cos(e2)*cos(e3)*cos(e4)^2*cos(e5)*cos(e6)^2 - de2*m6*y6*z6*cos(e4)^2*cos(e5)*cos(e6)*sin(e5) - de3*m6*y6*z6*cos(e4)^2*cos(e5)*cos(e6)*sin(e5) + 2*de4*m6*x6*y6*cos(e5)*cos(e6)^2*sin(e4)*sin(e5) - de2*m6*x6*z6*cos(e4)^2*cos(e5)*sin(e5)*sin(e6) - de3*m6*x6*z6*cos(e4)^2*cos(e5)*sin(e5)*sin(e6) + 2*de1*m6*x6^2*cos(e4)^2*cos(e5)*cos(e6)^2*sin(e2)*sin(e3) - 2*de1*m6*y6^2*cos(e4)^2*cos(e5)*cos(e6)^2*sin(e2)*sin(e3) - I6xx*de1*cos(e2)*cos(e3)*cos(e4)*cos(e6)*sin(e4)*sin(e6) + I6yy*de1*cos(e2)*cos(e3)*cos(e4)*cos(e6)*sin(e4)*sin(e6) - 2*I6xy*de1*cos(e2)*cos(e4)*cos(e6)*sin(e3)*sin(e5)*sin(e6) - 2*I6xy*de1*cos(e3)*cos(e4)*cos(e6)*sin(e2)*sin(e5)*sin(e6) + I6xx*de1*cos(e4)*cos(e6)*sin(e2)*sin(e3)*sin(e4)*sin(e6) - I6yy*de1*cos(e4)*cos(e6)*sin(e2)*sin(e3)*sin(e4)*sin(e6) + a3*de1*m6*y6*cos(e2)*cos(e3)*cos(e5)*cos(e6)*sin(e4) - I6xx*de1*cos(e2)*cos(e3)*cos(e4)*cos(e5)^2*cos(e6)*sin(e4)*sin(e6) + I6yy*de1*cos(e2)*cos(e3)*cos(e4)*cos(e5)^2*cos(e6)*sin(e4)*sin(e6) + a3*de1*m6*x6*cos(e2)*cos(e3)*cos(e5)*sin(e4)*sin(e6) - d4*de1*m6*y6*cos(e2)*cos(e5)*cos(e6)*sin(e3)*sin(e4) - d4*de1*m6*y6*cos(e3)*cos(e5)*cos(e6)*sin(e2)*sin(e4) - 2*de1*m6*x6*y6*cos(e2)*cos(e3)*cos(e5)*cos(e6)*sin(e6) + de1*m6*x6*z6*cos(e2)*cos(e4)*cos(e5)*cos(e6)*sin(e3) + de1*m6*x6*z6*cos(e3)*cos(e4)*cos(e5)*cos(e6)*sin(e2) - a3*de1*m6*y6*cos(e5)*cos(e6)*sin(e2)*sin(e3)*sin(e4) - d4*de1*m6*x6*cos(e2)*cos(e5)*sin(e3)*sin(e4)*sin(e6) - d4*de1*m6*x6*cos(e3)*cos(e5)*sin(e2)*sin(e4)*sin(e6) + I6xx*de1*cos(e4)*cos(e5)^2*cos(e6)*sin(e2)*sin(e3)*sin(e4)*sin(e6) - I6yy*de1*cos(e4)*cos(e5)^2*cos(e6)*sin(e2)*sin(e3)*sin(e4)*sin(e6) - 4*de2*m6*x6*y6*cos(e4)*cos(e5)*cos(e6)*sin(e4)*sin(e6) - 4*de3*m6*x6*y6*cos(e4)*cos(e5)*cos(e6)*sin(e4)*sin(e6) - de1*m6*y6*z6*cos(e2)*cos(e4)*cos(e5)*sin(e3)*sin(e6) - de1*m6*y6*z6*cos(e3)*cos(e4)*cos(e5)*sin(e2)*sin(e6) - a3*de1*m6*x6*cos(e5)*sin(e2)*sin(e3)*sin(e4)*sin(e6) + de1*m6*x6*y6*cos(e2)*cos(e5)*sin(e3)*sin(e4)*sin(e5) + de1*m6*x6*y6*cos(e3)*cos(e5)*sin(e2)*sin(e4)*sin(e5) + 2*de1*m6*x6*y6*cos(e5)*cos(e6)*sin(e2)*sin(e3)*sin(e6) - de1*m6*x6*y6*cos(e2)*cos(e3)*cos(e4)*cos(e5)^2*sin(e4) + 2*de1*m6*x6*y6*cos(e2)*cos(e3)*cos(e4)*cos(e6)^2*sin(e4) + de1*m6*x6*z6*cos(e2)*cos(e3)*cos(e4)^2*cos(e6)*sin(e5) - de1*m6*y6*z6*cos(e2)*cos(e3)*cos(e4)^2*sin(e5)*sin(e6) - de1*m6*y6*z6*cos(e2)*cos(e5)^2*cos(e6)*sin(e3)*sin(e4) - de1*m6*y6*z6*cos(e3)*cos(e5)^2*cos(e6)*sin(e2)*sin(e4) + de1*m6*x6*y6*cos(e4)*cos(e5)^2*sin(e2)*sin(e3)*sin(e4) - 2*de1*m6*x6*y6*cos(e4)*cos(e6)^2*sin(e2)*sin(e3)*sin(e4) - de1*m6*x6*z6*cos(e2)*cos(e5)^2*sin(e3)*sin(e4)*sin(e6) - de1*m6*x6*z6*cos(e3)*cos(e5)^2*sin(e2)*sin(e4)*sin(e6) - de1*m6*x6*z6*cos(e4)^2*cos(e6)*sin(e2)*sin(e3)*sin(e5) - I6yz*de1*cos(e2)*cos(e3)*cos(e4)*cos(e5)*cos(e6)*sin(e4)*sin(e5) + de1*m6*y6*z6*cos(e4)^2*sin(e2)*sin(e3)*sin(e5)*sin(e6) - I6zx*de1*cos(e2)*cos(e3)*cos(e4)*cos(e5)*sin(e4)*sin(e5)*sin(e6) + I6xx*de1*cos(e2)*cos(e5)*cos(e6)*sin(e3)*sin(e4)*sin(e5)*sin(e6) + I6xx*de1*cos(e3)*cos(e5)*cos(e6)*sin(e2)*sin(e4)*sin(e5)*sin(e6) + I6yz*de1*cos(e4)*cos(e5)*cos(e6)*sin(e2)*sin(e3)*sin(e4)*sin(e5) - I6yy*de1*cos(e2)*cos(e5)*cos(e6)*sin(e3)*sin(e4)*sin(e5)*sin(e6) - I6yy*de1*cos(e3)*cos(e5)*cos(e6)*sin(e2)*sin(e4)*sin(e5)*sin(e6) + I6zx*de1*cos(e4)*cos(e5)*sin(e2)*sin(e3)*sin(e4)*sin(e5)*sin(e6) + de1*m6*x6^2*cos(e2)*cos(e3)*cos(e4)*cos(e6)*sin(e4)*sin(e6) - de1*m6*y6^2*cos(e2)*cos(e3)*cos(e4)*cos(e6)*sin(e4)*sin(e6) - de1*m6*x6^2*cos(e4)*cos(e6)*sin(e2)*sin(e3)*sin(e4)*sin(e6) + de1*m6*y6^2*cos(e4)*cos(e6)*sin(e2)*sin(e3)*sin(e4)*sin(e6) + de1*m6*x6^2*cos(e2)*cos(e3)*cos(e4)*cos(e5)^2*cos(e6)*sin(e4)*sin(e6) - de1*m6*y6^2*cos(e2)*cos(e3)*cos(e4)*cos(e5)^2*cos(e6)*sin(e4)*sin(e6) - 2*de1*m6*x6*y6*cos(e2)*cos(e4)*cos(e6)*sin(e3)*sin(e5)*sin(e6) - 2*de1*m6*x6*y6*cos(e3)*cos(e4)*cos(e6)*sin(e2)*sin(e5)*sin(e6) - de1*m6*x6^2*cos(e4)*cos(e5)^2*cos(e6)*sin(e2)*sin(e3)*sin(e4)*sin(e6) + de1*m6*y6^2*cos(e4)*cos(e5)^2*cos(e6)*sin(e2)*sin(e3)*sin(e4)*sin(e6) + 4*de1*m6*x6*y6*cos(e2)*cos(e3)*cos(e4)^2*cos(e5)*cos(e6)*sin(e6) - 2*de1*m6*x6*y6*cos(e2)*cos(e5)*cos(e6)^2*sin(e3)*sin(e4)*sin(e5) - 2*de1*m6*x6*y6*cos(e3)*cos(e5)*cos(e6)^2*sin(e2)*sin(e4)*sin(e5) - 4*de1*m6*x6*y6*cos(e4)^2*cos(e5)*cos(e6)*sin(e2)*sin(e3)*sin(e6) + 2*de1*m6*x6*y6*cos(e2)*cos(e3)*cos(e4)*cos(e5)^2*cos(e6)^2*sin(e4) - de1*m6*x6^2*cos(e2)*cos(e5)*cos(e6)*sin(e3)*sin(e4)*sin(e5)*sin(e6) - de1*m6*x6^2*cos(e3)*cos(e5)*cos(e6)*sin(e2)*sin(e4)*sin(e5)*sin(e6) - 2*de1*m6*x6*y6*cos(e4)*cos(e5)^2*cos(e6)^2*sin(e2)*sin(e3)*sin(e4) + de1*m6*y6^2*cos(e2)*cos(e5)*cos(e6)*sin(e3)*sin(e4)*sin(e5)*sin(e6) + de1*m6*y6^2*cos(e3)*cos(e5)*cos(e6)*sin(e2)*sin(e4)*sin(e5)*sin(e6) - de1*m6*y6*z6*cos(e2)*cos(e3)*cos(e4)*cos(e5)*cos(e6)*sin(e4)*sin(e5) - de1*m6*x6*z6*cos(e2)*cos(e3)*cos(e4)*cos(e5)*sin(e4)*sin(e5)*sin(e6) + de1*m6*y6*z6*cos(e4)*cos(e5)*cos(e6)*sin(e2)*sin(e3)*sin(e4)*sin(e5) + de1*m6*x6*z6*cos(e4)*cos(e5)*sin(e2)*sin(e3)*sin(e4)*sin(e5)*sin(e6),I6xy*de4 - I6xy*de4*cos(e5)^2 - 2*I6xy*de4*cos(e6)^2 + (I6xx*de4*sin(2*e6))/2 - (I6yy*de4*sin(2*e6))/2 - (I6xx*de5*sin(e5))/2 + (I6yy*de5*sin(e5))/2 - (I6zz*de5*sin(e5))/2 + I6xx*de5*cos(e6)^2*sin(e5) - I6yy*de5*cos(e6)^2*sin(e5) + de4*m6*x6*y6 - (de4*m6*x6^2*sin(2*e6))/2 + (de4*m6*y6^2*sin(2*e6))/2 + 2*I6xy*de4*cos(e5)^2*cos(e6)^2 - I6zx*de5*cos(e5)*cos(e6) - I6xy*de1*cos(e2)*sin(e3) - I6xy*de1*cos(e3)*sin(e2) - (I6xx*de2*cos(e4)*sin(e5))/2 - (I6xx*de3*cos(e4)*sin(e5))/2 + (I6yy*de2*cos(e4)*sin(e5))/2 + (I6yy*de3*cos(e4)*sin(e5))/2 - I6yz*de2*cos(e6)*sin(e4) - I6yz*de3*cos(e6)*sin(e4) + I6yz*de5*cos(e5)*sin(e6) + (I6zz*de2*cos(e4)*sin(e5))/2 + (I6zz*de3*cos(e4)*sin(e5))/2 - I6zx*de2*sin(e4)*sin(e6) - I6zx*de3*sin(e4)*sin(e6) - de5*m6*y6^2*sin(e5) - de5*m6*x6^2*cos(e6)^2*sin(e5) + de5*m6*y6^2*cos(e6)^2*sin(e5) - de4*m6*x6*y6*cos(e5)^2 - 2*de4*m6*x6*y6*cos(e6)^2 - I6yz*de4*cos(e5)*cos(e6)*sin(e5) - I6xy*de2*cos(e5)*sin(e4)*sin(e5) - I6xy*de3*cos(e5)*sin(e4)*sin(e5) + 2*I6xy*de5*cos(e6)*sin(e5)*sin(e6) - I6zx*de4*cos(e5)*sin(e5)*sin(e6) + de2*m6*x6^2*cos(e4)*sin(e5) + de3*m6*x6^2*cos(e4)*sin(e5) + I6xy*de1*cos(e2)*cos(e5)^2*sin(e3) + I6xy*de1*cos(e3)*cos(e5)^2*sin(e2) + 2*I6xy*de1*cos(e2)*cos(e6)^2*sin(e3) + 2*I6xy*de1*cos(e3)*cos(e6)^2*sin(e2) + I6xx*de2*cos(e4)*cos(e6)^2*sin(e5) + I6xx*de3*cos(e4)*cos(e6)^2*sin(e5) - I6xx*de4*cos(e5)^2*cos(e6)*sin(e6) - I6yy*de2*cos(e4)*cos(e6)^2*sin(e5) - I6yy*de3*cos(e4)*cos(e6)^2*sin(e5) + I6yz*de2*cos(e5)^2*cos(e6)*sin(e4) + I6yz*de3*cos(e5)^2*cos(e6)*sin(e4) + I6yy*de4*cos(e5)^2*cos(e6)*sin(e6) + I6zx*de2*cos(e5)^2*sin(e4)*sin(e6) + I6zx*de3*cos(e5)^2*sin(e4)*sin(e6) + I6yz*de1*cos(e2)*cos(e3)*cos(e4)*cos(e6) + I6zx*de1*cos(e2)*cos(e3)*cos(e4)*sin(e6) - (I6xx*de1*cos(e2)*cos(e3)*sin(e4)*sin(e5))/2 - I6xx*de1*cos(e2)*cos(e6)*sin(e3)*sin(e6) - I6xx*de1*cos(e3)*cos(e6)*sin(e2)*sin(e6) + 2*I6xy*de2*cos(e4)*cos(e6)*sin(e5)*sin(e6) + 2*I6xy*de3*cos(e4)*cos(e6)*sin(e5)*sin(e6) + (I6yy*de1*cos(e2)*cos(e3)*sin(e4)*sin(e5))/2 - I6yz*de1*cos(e4)*cos(e6)*sin(e2)*sin(e3) + I6yy*de1*cos(e2)*cos(e6)*sin(e3)*sin(e6) + I6yy*de1*cos(e3)*cos(e6)*sin(e2)*sin(e6) + (I6zz*de1*cos(e2)*cos(e3)*sin(e4)*sin(e5))/2 - I6zx*de1*cos(e4)*sin(e2)*sin(e3)*sin(e6) + (I6xx*de1*sin(e2)*sin(e3)*sin(e4)*sin(e5))/2 - (I6yy*de1*sin(e2)*sin(e3)*sin(e4)*sin(e5))/2 - (I6zz*de1*sin(e2)*sin(e3)*sin(e4)*sin(e5))/2 + 2*de4*m6*x6*y6*cos(e5)^2*cos(e6)^2 + 2*I6xy*de2*cos(e5)*cos(e6)^2*sin(e4)*sin(e5) + 2*I6xy*de3*cos(e5)*cos(e6)^2*sin(e4)*sin(e5) - de5*m6*x6*z6*cos(e5)*cos(e6) - de1*m6*x6*y6*cos(e2)*sin(e3) - de1*m6*x6*y6*cos(e3)*sin(e2) - de2*m6*y6*z6*cos(e6)*sin(e4) - de3*m6*y6*z6*cos(e6)*sin(e4) + de5*m6*y6*z6*cos(e5)*sin(e6) - de2*m6*x6^2*cos(e4)*cos(e6)^2*sin(e5) - de3*m6*x6^2*cos(e4)*cos(e6)^2*sin(e5) + de4*m6*x6^2*cos(e5)^2*cos(e6)*sin(e6) + de2*m6*y6^2*cos(e4)*cos(e6)^2*sin(e5) + de3*m6*y6^2*cos(e4)*cos(e6)^2*sin(e5) - de4*m6*y6^2*cos(e5)^2*cos(e6)*sin(e6) - de2*m6*x6*z6*sin(e4)*sin(e6) - de3*m6*x6*z6*sin(e4)*sin(e6) - 2*I6xy*de1*cos(e2)*cos(e5)^2*cos(e6)^2*sin(e3) - 2*I6xy*de1*cos(e3)*cos(e5)^2*cos(e6)^2*sin(e2) + I6xy*de1*cos(e2)*cos(e3)*cos(e4)*cos(e5)*sin(e5) + I6yz*de1*cos(e2)*cos(e5)*cos(e6)*sin(e3)*sin(e5) + I6yz*de1*cos(e3)*cos(e5)*cos(e6)*sin(e2)*sin(e5) - I6xy*de1*cos(e4)*cos(e5)*sin(e2)*sin(e3)*sin(e5) - I6xx*de2*cos(e5)*cos(e6)*sin(e4)*sin(e5)*sin(e6) - I6xx*de3*cos(e5)*cos(e6)*sin(e4)*sin(e5)*sin(e6) + I6yy*de2*cos(e5)*cos(e6)*sin(e4)*sin(e5)*sin(e6) + I6yy*de3*cos(e5)*cos(e6)*sin(e4)*sin(e5)*sin(e6) + I6zx*de1*cos(e2)*cos(e5)*sin(e3)*sin(e5)*sin(e6) + I6zx*de1*cos(e3)*cos(e5)*sin(e2)*sin(e5)*sin(e6) + de1*m6*x6^2*cos(e2)*cos(e3)*sin(e4)*sin(e5) + de1*m6*x6^2*cos(e2)*cos(e6)*sin(e3)*sin(e6) + de1*m6*x6^2*cos(e3)*cos(e6)*sin(e2)*sin(e6) - de1*m6*y6^2*cos(e2)*cos(e6)*sin(e3)*sin(e6) - de1*m6*y6^2*cos(e3)*cos(e6)*sin(e2)*sin(e6) - I6yz*de1*cos(e2)*cos(e3)*cos(e4)*cos(e5)^2*cos(e6) - I6zx*de1*cos(e2)*cos(e3)*cos(e4)*cos(e5)^2*sin(e6) - de1*m6*x6^2*sin(e2)*sin(e3)*sin(e4)*sin(e5) + I6xx*de1*cos(e2)*cos(e3)*cos(e6)^2*sin(e4)*sin(e5) + I6xx*de1*cos(e2)*cos(e5)^2*cos(e6)*sin(e3)*sin(e6) + I6xx*de1*cos(e3)*cos(e5)^2*cos(e6)*sin(e2)*sin(e6) - I6yy*de1*cos(e2)*cos(e3)*cos(e6)^2*sin(e4)*sin(e5) + I6yz*de1*cos(e4)*cos(e5)^2*cos(e6)*sin(e2)*sin(e3) - I6yy*de1*cos(e2)*cos(e5)^2*cos(e6)*sin(e3)*sin(e6) - I6yy*de1*cos(e3)*cos(e5)^2*cos(e6)*sin(e2)*sin(e6) + I6zx*de1*cos(e4)*cos(e5)^2*sin(e2)*sin(e3)*sin(e6) - de4*m6*y6*z6*cos(e5)*cos(e6)*sin(e5) - I6xx*de1*cos(e6)^2*sin(e2)*sin(e3)*sin(e4)*sin(e5) + I6yy*de1*cos(e6)^2*sin(e2)*sin(e3)*sin(e4)*sin(e5) - de2*m6*x6*y6*cos(e5)*sin(e4)*sin(e5) - de3*m6*x6*y6*cos(e5)*sin(e4)*sin(e5) + 2*de5*m6*x6*y6*cos(e6)*sin(e5)*sin(e6) - de4*m6*x6*z6*cos(e5)*sin(e5)*sin(e6) + de1*m6*x6*y6*cos(e2)*cos(e5)^2*sin(e3) + de1*m6*x6*y6*cos(e3)*cos(e5)^2*sin(e2) + 2*de1*m6*x6*y6*cos(e2)*cos(e6)^2*sin(e3) + 2*de1*m6*x6*y6*cos(e3)*cos(e6)^2*sin(e2) + de2*m6*y6*z6*cos(e5)^2*cos(e6)*sin(e4) + de3*m6*y6*z6*cos(e5)^2*cos(e6)*sin(e4) + de2*m6*x6*z6*cos(e5)^2*sin(e4)*sin(e6) + de3*m6*x6*z6*cos(e5)^2*sin(e4)*sin(e6) - 2*I6xy*de1*cos(e6)*sin(e2)*sin(e3)*sin(e4)*sin(e5)*sin(e6) - 2*de1*m6*x6*y6*cos(e2)*cos(e5)^2*cos(e6)^2*sin(e3) - 2*de1*m6*x6*y6*cos(e3)*cos(e5)^2*cos(e6)^2*sin(e2) + de2*m6*x6^2*cos(e5)*cos(e6)*sin(e4)*sin(e5)*sin(e6) + de3*m6*x6^2*cos(e5)*cos(e6)*sin(e4)*sin(e5)*sin(e6) - de2*m6*y6^2*cos(e5)*cos(e6)*sin(e4)*sin(e5)*sin(e6) - de3*m6*y6^2*cos(e5)*cos(e6)*sin(e4)*sin(e5)*sin(e6) - 2*I6xy*de1*cos(e2)*cos(e3)*cos(e4)*cos(e5)*cos(e6)^2*sin(e5) + de1*m6*y6*z6*cos(e2)*cos(e3)*cos(e4)*cos(e6) + 2*I6xy*de1*cos(e4)*cos(e5)*cos(e6)^2*sin(e2)*sin(e3)*sin(e5) + de1*m6*x6*z6*cos(e2)*cos(e3)*cos(e4)*sin(e6) + 2*de2*m6*x6*y6*cos(e4)*cos(e6)*sin(e5)*sin(e6) + 2*de3*m6*x6*y6*cos(e4)*cos(e6)*sin(e5)*sin(e6) - de1*m6*y6*z6*cos(e4)*cos(e6)*sin(e2)*sin(e3) - de1*m6*x6^2*cos(e2)*cos(e3)*cos(e6)^2*sin(e4)*sin(e5) - de1*m6*x6^2*cos(e2)*cos(e5)^2*cos(e6)*sin(e3)*sin(e6) - de1*m6*x6^2*cos(e3)*cos(e5)^2*cos(e6)*sin(e2)*sin(e6) + de1*m6*y6^2*cos(e2)*cos(e3)*cos(e6)^2*sin(e4)*sin(e5) + de1*m6*y6^2*cos(e2)*cos(e5)^2*cos(e6)*sin(e3)*sin(e6) + de1*m6*y6^2*cos(e3)*cos(e5)^2*cos(e6)*sin(e2)*sin(e6) - de1*m6*x6*z6*cos(e4)*sin(e2)*sin(e3)*sin(e6) + de1*m6*x6^2*cos(e6)^2*sin(e2)*sin(e3)*sin(e4)*sin(e5) - de1*m6*y6^2*cos(e6)^2*sin(e2)*sin(e3)*sin(e4)*sin(e5) + 2*de2*m6*x6*y6*cos(e5)*cos(e6)^2*sin(e4)*sin(e5) + 2*de3*m6*x6*y6*cos(e5)*cos(e6)^2*sin(e4)*sin(e5) + 2*I6xy*de1*cos(e2)*cos(e3)*cos(e6)*sin(e4)*sin(e5)*sin(e6) + de1*m6*x6*y6*cos(e2)*cos(e3)*cos(e4)*cos(e5)*sin(e5) + de1*m6*y6*z6*cos(e2)*cos(e5)*cos(e6)*sin(e3)*sin(e5) + de1*m6*y6*z6*cos(e3)*cos(e5)*cos(e6)*sin(e2)*sin(e5) - de1*m6*x6*y6*cos(e4)*cos(e5)*sin(e2)*sin(e3)*sin(e5) + de1*m6*x6*z6*cos(e2)*cos(e5)*sin(e3)*sin(e5)*sin(e6) + de1*m6*x6*z6*cos(e3)*cos(e5)*sin(e2)*sin(e5)*sin(e6) - de1*m6*y6*z6*cos(e2)*cos(e3)*cos(e4)*cos(e5)^2*cos(e6) - de1*m6*x6*z6*cos(e2)*cos(e3)*cos(e4)*cos(e5)^2*sin(e6) + de1*m6*y6*z6*cos(e4)*cos(e5)^2*cos(e6)*sin(e2)*sin(e3) + de1*m6*x6*z6*cos(e4)*cos(e5)^2*sin(e2)*sin(e3)*sin(e6) + I6xx*de1*cos(e2)*cos(e3)*cos(e4)*cos(e5)*cos(e6)*sin(e5)*sin(e6) - I6yy*de1*cos(e2)*cos(e3)*cos(e4)*cos(e5)*cos(e6)*sin(e5)*sin(e6) - I6xx*de1*cos(e4)*cos(e5)*cos(e6)*sin(e2)*sin(e3)*sin(e5)*sin(e6) + I6yy*de1*cos(e4)*cos(e5)*cos(e6)*sin(e2)*sin(e3)*sin(e5)*sin(e6) + 2*de1*m6*x6*y6*cos(e2)*cos(e3)*cos(e6)*sin(e4)*sin(e5)*sin(e6) - 2*de1*m6*x6*y6*cos(e6)*sin(e2)*sin(e3)*sin(e4)*sin(e5)*sin(e6) - 2*de1*m6*x6*y6*cos(e2)*cos(e3)*cos(e4)*cos(e5)*cos(e6)^2*sin(e5) + 2*de1*m6*x6*y6*cos(e4)*cos(e5)*cos(e6)^2*sin(e2)*sin(e3)*sin(e5) - de1*m6*x6^2*cos(e2)*cos(e3)*cos(e4)*cos(e5)*cos(e6)*sin(e5)*sin(e6) + de1*m6*y6^2*cos(e2)*cos(e3)*cos(e4)*cos(e5)*cos(e6)*sin(e5)*sin(e6) + de1*m6*x6^2*cos(e4)*cos(e5)*cos(e6)*sin(e2)*sin(e3)*sin(e5)*sin(e6) - de1*m6*y6^2*cos(e4)*cos(e5)*cos(e6)*sin(e2)*sin(e3)*sin(e5)*sin(e6),2*I6xy*de5*cos(e6)^2 - I6xy*de5 - (I6xx*de5*sin(2*e6))/2 + (I6yy*de5*sin(2*e6))/2 - I6xy*de2*cos(e4) - I6xy*de3*cos(e4) - (I6xx*de4*sin(e5))/2 + (I6yy*de4*sin(e5))/2 - (I6zz*de4*sin(e5))/2 + I6xx*de4*cos(e6)^2*sin(e5) - I6yy*de4*cos(e6)^2*sin(e5) - de5*m6*x6*y6 + (de5*m6*x6^2*sin(2*e6))/2 - (de5*m6*y6^2*sin(2*e6))/2 - I6zx*de4*cos(e5)*cos(e6) + (I6xx*de2*cos(e5)*sin(e4))/2 + (I6xx*de3*cos(e5)*sin(e4))/2 - (I6yy*de2*cos(e5)*sin(e4))/2 - (I6yy*de3*cos(e5)*sin(e4))/2 + I6yz*de4*cos(e5)*sin(e6) + (I6zz*de2*cos(e5)*sin(e4))/2 + (I6zz*de3*cos(e5)*sin(e4))/2 - de4*m6*y6^2*sin(e5) + 2*I6xy*de2*cos(e4)*cos(e6)^2 + 2*I6xy*de3*cos(e4)*cos(e6)^2 - de4*m6*x6^2*cos(e6)^2*sin(e5) + de4*m6*y6^2*cos(e6)^2*sin(e5) + 2*de5*m6*x6*y6*cos(e6)^2 - I6xy*de1*cos(e2)*cos(e3)*sin(e4) - I6xx*de2*cos(e4)*cos(e6)*sin(e6) - I6xx*de3*cos(e4)*cos(e6)*sin(e6) + I6yy*de2*cos(e4)*cos(e6)*sin(e6) + I6yy*de3*cos(e4)*cos(e6)*sin(e6) + (I6xx*de1*cos(e2)*sin(e3)*sin(e5))/2 + (I6xx*de1*cos(e3)*sin(e2)*sin(e5))/2 + 2*I6xy*de4*cos(e6)*sin(e5)*sin(e6) - (I6yy*de1*cos(e2)*sin(e3)*sin(e5))/2 - (I6yy*de1*cos(e3)*sin(e2)*sin(e5))/2 + (I6zz*de1*cos(e2)*sin(e3)*sin(e5))/2 + (I6zz*de1*cos(e3)*sin(e2)*sin(e5))/2 - I6zx*de2*cos(e6)*sin(e4)*sin(e5) - I6zx*de3*cos(e6)*sin(e4)*sin(e5) + I6xy*de1*sin(e2)*sin(e3)*sin(e4) + I6yz*de2*sin(e4)*sin(e5)*sin(e6) + I6yz*de3*sin(e4)*sin(e5)*sin(e6) + de2*m6*y6^2*cos(e5)*sin(e4) + de3*m6*y6^2*cos(e5)*sin(e4) - I6xx*de2*cos(e5)*cos(e6)^2*sin(e4) - I6xx*de3*cos(e5)*cos(e6)^2*sin(e4) + I6yy*de2*cos(e5)*cos(e6)^2*sin(e4) + I6yy*de3*cos(e5)*cos(e6)^2*sin(e4) - de2*m6*x6*y6*cos(e4) - de3*m6*x6*y6*cos(e4) + 2*de2*m6*x6*y6*cos(e4)*cos(e6)^2 + 2*de3*m6*x6*y6*cos(e4)*cos(e6)^2 - (I6xx*de1*cos(e2)*cos(e3)*cos(e4)*cos(e5))/2 + (I6yy*de1*cos(e2)*cos(e3)*cos(e4)*cos(e5))/2 - (I6zz*de1*cos(e2)*cos(e3)*cos(e4)*cos(e5))/2 + I6zx*de1*cos(e2)*cos(e5)*cos(e6)*sin(e3) + I6zx*de1*cos(e3)*cos(e5)*cos(e6)*sin(e2) + (I6xx*de1*cos(e4)*cos(e5)*sin(e2)*sin(e3))/2 - 2*I6xy*de2*cos(e5)*cos(e6)*sin(e4)*sin(e6) - 2*I6xy*de3*cos(e5)*cos(e6)*sin(e4)*sin(e6) - (I6yy*de1*cos(e4)*cos(e5)*sin(e2)*sin(e3))/2 - I6yz*de1*cos(e2)*cos(e5)*sin(e3)*sin(e6) - I6yz*de1*cos(e3)*cos(e5)*sin(e2)*sin(e6) + (I6zz*de1*cos(e4)*cos(e5)*sin(e2)*sin(e3))/2 + de2*m6*x6^2*cos(e4)*cos(e6)*sin(e6) + de3*m6*x6^2*cos(e4)*cos(e6)*sin(e6) - de2*m6*y6^2*cos(e4)*cos(e6)*sin(e6) - de3*m6*y6^2*cos(e4)*cos(e6)*sin(e6) + de1*m6*y6^2*cos(e2)*sin(e3)*sin(e5) + de1*m6*y6^2*cos(e3)*sin(e2)*sin(e5) + 2*I6xy*de1*cos(e2)*cos(e3)*cos(e6)^2*sin(e4) - I6xx*de1*cos(e2)*cos(e6)^2*sin(e3)*sin(e5) - I6xx*de1*cos(e3)*cos(e6)^2*sin(e2)*sin(e5) + I6yy*de1*cos(e2)*cos(e6)^2*sin(e3)*sin(e5) + I6yy*de1*cos(e3)*cos(e6)^2*sin(e2)*sin(e5) - de4*m6*x6*z6*cos(e5)*cos(e6) - 2*I6xy*de1*cos(e6)^2*sin(e2)*sin(e3)*sin(e4) + de4*m6*y6*z6*cos(e5)*sin(e6) + de2*m6*x6^2*cos(e5)*cos(e6)^2*sin(e4) + de3*m6*x6^2*cos(e5)*cos(e6)^2*sin(e4) - de2*m6*y6^2*cos(e5)*cos(e6)^2*sin(e4) - de3*m6*y6^2*cos(e5)*cos(e6)^2*sin(e4) + I6zx*de1*cos(e2)*cos(e3)*cos(e4)*cos(e6)*sin(e5) - I6xx*de1*cos(e2)*cos(e3)*cos(e6)*sin(e4)*sin(e6) + I6yy*de1*cos(e2)*cos(e3)*cos(e6)*sin(e4)*sin(e6) - I6yz*de1*cos(e2)*cos(e3)*cos(e4)*sin(e5)*sin(e6) - 2*I6xy*de1*cos(e2)*cos(e6)*sin(e3)*sin(e5)*sin(e6) - 2*I6xy*de1*cos(e3)*cos(e6)*sin(e2)*sin(e5)*sin(e6) - I6zx*de1*cos(e4)*cos(e6)*sin(e2)*sin(e3)*sin(e5) - de1*m6*y6^2*cos(e2)*cos(e3)*cos(e4)*cos(e5) + I6xx*de1*cos(e6)*sin(e2)*sin(e3)*sin(e4)*sin(e6) - I6yy*de1*cos(e6)*sin(e2)*sin(e3)*sin(e4)*sin(e6) + I6yz*de1*cos(e4)*sin(e2)*sin(e3)*sin(e5)*sin(e6) + de1*m6*y6^2*cos(e4)*cos(e5)*sin(e2)*sin(e3) + I6xx*de1*cos(e2)*cos(e3)*cos(e4)*cos(e5)*cos(e6)^2 - I6yy*de1*cos(e2)*cos(e3)*cos(e4)*cos(e5)*cos(e6)^2 - I6xx*de1*cos(e4)*cos(e5)*cos(e6)^2*sin(e2)*sin(e3) + I6yy*de1*cos(e4)*cos(e5)*cos(e6)^2*sin(e2)*sin(e3) - de1*m6*x6*y6*cos(e2)*cos(e3)*sin(e4) + 2*de4*m6*x6*y6*cos(e6)*sin(e5)*sin(e6) - de2*m6*x6*z6*cos(e6)*sin(e4)*sin(e5) - de3*m6*x6*z6*cos(e6)*sin(e4)*sin(e5) + de1*m6*x6^2*cos(e2)*cos(e6)^2*sin(e3)*sin(e5) + de1*m6*x6^2*cos(e3)*cos(e6)^2*sin(e2)*sin(e5) - de1*m6*y6^2*cos(e2)*cos(e6)^2*sin(e3)*sin(e5) - de1*m6*y6^2*cos(e3)*cos(e6)^2*sin(e2)*sin(e5) + de1*m6*x6*y6*sin(e2)*sin(e3)*sin(e4) + de2*m6*y6*z6*sin(e4)*sin(e5)*sin(e6) + de3*m6*y6*z6*sin(e4)*sin(e5)*sin(e6) + de1*m6*x6^2*cos(e2)*cos(e3)*cos(e6)*sin(e4)*sin(e6) - de1*m6*y6^2*cos(e2)*cos(e3)*cos(e6)*sin(e4)*sin(e6) - de1*m6*x6^2*cos(e6)*sin(e2)*sin(e3)*sin(e4)*sin(e6) + de1*m6*y6^2*cos(e6)*sin(e2)*sin(e3)*sin(e4)*sin(e6) - de1*m6*x6^2*cos(e2)*cos(e3)*cos(e4)*cos(e5)*cos(e6)^2 + de1*m6*y6^2*cos(e2)*cos(e3)*cos(e4)*cos(e5)*cos(e6)^2 + de1*m6*x6*z6*cos(e2)*cos(e5)*cos(e6)*sin(e3) + de1*m6*x6*z6*cos(e3)*cos(e5)*cos(e6)*sin(e2) - 2*de2*m6*x6*y6*cos(e5)*cos(e6)*sin(e4)*sin(e6) - 2*de3*m6*x6*y6*cos(e5)*cos(e6)*sin(e4)*sin(e6) - de1*m6*y6*z6*cos(e2)*cos(e5)*sin(e3)*sin(e6) - de1*m6*y6*z6*cos(e3)*cos(e5)*sin(e2)*sin(e6) + de1*m6*x6^2*cos(e4)*cos(e5)*cos(e6)^2*sin(e2)*sin(e3) - de1*m6*y6^2*cos(e4)*cos(e5)*cos(e6)^2*sin(e2)*sin(e3) + 2*de1*m6*x6*y6*cos(e2)*cos(e3)*cos(e6)^2*sin(e4) + 2*I6xy*de1*cos(e2)*cos(e3)*cos(e4)*cos(e5)*cos(e6)*sin(e6) - 2*de1*m6*x6*y6*cos(e6)^2*sin(e2)*sin(e3)*sin(e4) - 2*I6xy*de1*cos(e4)*cos(e5)*cos(e6)*sin(e2)*sin(e3)*sin(e6) + de1*m6*x6*z6*cos(e2)*cos(e3)*cos(e4)*cos(e6)*sin(e5) - de1*m6*y6*z6*cos(e2)*cos(e3)*cos(e4)*sin(e5)*sin(e6) - 2*de1*m6*x6*y6*cos(e2)*cos(e6)*sin(e3)*sin(e5)*sin(e6) - 2*de1*m6*x6*y6*cos(e3)*cos(e6)*sin(e2)*sin(e5)*sin(e6) - de1*m6*x6*z6*cos(e4)*cos(e6)*sin(e2)*sin(e3)*sin(e5) + de1*m6*y6*z6*cos(e4)*sin(e2)*sin(e3)*sin(e5)*sin(e6) - 2*de1*m6*x6*y6*cos(e4)*cos(e5)*cos(e6)*sin(e2)*sin(e3)*sin(e6) + 2*de1*m6*x6*y6*cos(e2)*cos(e3)*cos(e4)*cos(e5)*cos(e6)*sin(e6),(de5*(2*m6*(y6*cos(e6) + x6*sin(e6))*(sin(e2 + e3)*cos(e5) + cos(e2 + e3)*cos(e4)*sin(e5))*(y6*(cos(e2 + e3)*sin(e4)*sin(e6) + sin(e2 + e3)*cos(e6)*sin(e5) - cos(e2 + e3)*cos(e4)*cos(e5)*cos(e6)) - x6*(cos(e2 + e3)*cos(e6)*sin(e4) - sin(e2 + e3)*sin(e5)*sin(e6) + cos(e2 + e3)*cos(e4)*cos(e5)*sin(e6))) + 2*m6*(y6*cos(e6) + x6*sin(e6))*(x6*(cos(e6)*(cos(e4)*sin(e1) - sin(e2 + e3)*cos(e1)*sin(e4)) - sin(e6)*(cos(e2 + e3)*cos(e1)*sin(e5) + cos(e5)*sin(e1)*sin(e4) + sin(e2 + e3)*cos(e1)*cos(e4)*cos(e5))) - y6*(sin(e6)*(cos(e4)*sin(e1) - sin(e2 + e3)*cos(e1)*sin(e4)) + cos(e6)*(cos(e2 + e3)*cos(e1)*sin(e5) + cos(e5)*sin(e1)*sin(e4) + sin(e2 + e3)*cos(e1)*cos(e4)*cos(e5))))*(sin(e1)*sin(e4)*sin(e5) - cos(e2 + e3)*cos(e1)*cos(e5) + sin(e2 + e3)*cos(e1)*cos(e4)*sin(e5)) + 2*m6*(y6*cos(e6) + x6*sin(e6))*(x6*(cos(e1)*cos(e4)*cos(e6) + sin(e2 + e3)*cos(e6)*sin(e1)*sin(e4) + cos(e2 + e3)*sin(e1)*sin(e5)*sin(e6) - cos(e1)*cos(e5)*sin(e4)*sin(e6) + sin(e2 + e3)*cos(e4)*cos(e5)*sin(e1)*sin(e6)) - y6*(sin(e6)*(cos(e1)*cos(e4) + sin(e2 + e3)*sin(e1)*sin(e4)) - cos(e6)*(cos(e2 + e3)*sin(e1)*sin(e5) - cos(e1)*cos(e5)*sin(e4) + sin(e2 + e3)*cos(e4)*cos(e5)*sin(e1))))*(cos(e2 + e3)*cos(e5)*sin(e1) + cos(e1)*sin(e4)*sin(e5) - sin(e2 + e3)*cos(e4)*sin(e1)*sin(e5))))/2 - (de4*(2*m6*(x6*(cos(e2 + e3)*cos(e4)*cos(e6) - cos(e2 + e3)*cos(e5)*sin(e4)*sin(e6)) - y6*(cos(e2 + e3)*cos(e4)*sin(e6) + cos(e2 + e3)*cos(e5)*cos(e6)*sin(e4)))*(x6*(sin(e6)*(sin(e2 + e3)*sin(e5) - cos(e2 + e3)*cos(e4)*cos(e5)) - cos(e2 + e3)*cos(e6)*sin(e4)) + y6*(cos(e6)*(sin(e2 + e3)*sin(e5) - cos(e2 + e3)*cos(e4)*cos(e5)) + cos(e2 + e3)*sin(e4)*sin(e6))) + 2*m6*(x6*(cos(e6)*(sin(e1)*sin(e4) + sin(e2 + e3)*cos(e1)*cos(e4)) + cos(e5)*sin(e6)*(cos(e4)*sin(e1) - sin(e2 + e3)*cos(e1)*sin(e4))) - y6*(sin(e6)*(sin(e1)*sin(e4) + sin(e2 + e3)*cos(e1)*cos(e4)) - cos(e5)*cos(e6)*(cos(e4)*sin(e1) - sin(e2 + e3)*cos(e1)*sin(e4))))*(x6*(cos(e6)*(cos(e4)*sin(e1) - sin(e2 + e3)*cos(e1)*sin(e4)) - sin(e6)*(cos(e5)*(sin(e1)*sin(e4) + sin(e2 + e3)*cos(e1)*cos(e4)) + cos(e2 + e3)*cos(e1)*sin(e5))) - y6*(sin(e6)*(cos(e4)*sin(e1) - sin(e2 + e3)*cos(e1)*sin(e4)) + cos(e6)*(cos(e5)*(sin(e1)*sin(e4) + sin(e2 + e3)*cos(e1)*cos(e4)) + cos(e2 + e3)*cos(e1)*sin(e5)))) + 2*m6*(x6*(cos(e6)*(cos(e1)*sin(e4) - sin(e2 + e3)*cos(e4)*sin(e1)) + cos(e5)*sin(e6)*(cos(e1)*cos(e4) + sin(e2 + e3)*sin(e1)*sin(e4))) - y6*(sin(e6)*(cos(e1)*sin(e4) - sin(e2 + e3)*cos(e4)*sin(e1)) - cos(e5)*cos(e6)*(cos(e1)*cos(e4) + sin(e2 + e3)*sin(e1)*sin(e4))))*(x6*(cos(e6)*(cos(e1)*cos(e4) + sin(e2 + e3)*sin(e1)*sin(e4)) - sin(e6)*(cos(e5)*(cos(e1)*sin(e4) - sin(e2 + e3)*cos(e4)*sin(e1)) - cos(e2 + e3)*sin(e1)*sin(e5))) - y6*(sin(e6)*(cos(e1)*cos(e4) + sin(e2 + e3)*sin(e1)*sin(e4)) + cos(e6)*(cos(e5)*(cos(e1)*sin(e4) - sin(e2 + e3)*cos(e4)*sin(e1)) - cos(e2 + e3)*sin(e1)*sin(e5))))))/2 + (de2*(2*m6*(x6*(sin(e6)*(sin(e2 + e3)*sin(e5) - cos(e2 + e3)*cos(e4)*cos(e5)) - cos(e2 + e3)*cos(e6)*sin(e4)) + y6*(cos(e6)*(sin(e2 + e3)*sin(e5) - cos(e2 + e3)*cos(e4)*cos(e5)) + cos(e2 + e3)*sin(e4)*sin(e6)))*(x6*(sin(e6)*(cos(e2 + e3)*sin(e5) + sin(e2 + e3)*cos(e4)*cos(e5)) + sin(e2 + e3)*cos(e6)*sin(e4)) + y6*(cos(e6)*(cos(e2 + e3)*sin(e5) + sin(e2 + e3)*cos(e4)*cos(e5)) - sin(e2 + e3)*sin(e4)*sin(e6))) - 2*m6*(x6*(cos(e6)*(cos(e1)*cos(e4) + sin(e2 + e3)*sin(e1)*sin(e4)) - sin(e6)*(cos(e5)*(cos(e1)*sin(e4) - sin(e2 + e3)*cos(e4)*sin(e1)) - cos(e2 + e3)*sin(e1)*sin(e5))) - y6*(sin(e6)*(cos(e1)*cos(e4) + sin(e2 + e3)*sin(e1)*sin(e4)) + cos(e6)*(cos(e5)*(cos(e1)*sin(e4) - sin(e2 + e3)*cos(e4)*sin(e1)) - cos(e2 + e3)*sin(e1)*sin(e5))))*(x6*(sin(e6)*(sin(e2 + e3)*sin(e1)*sin(e5) - cos(e2 + e3)*cos(e4)*cos(e5)*sin(e1)) - cos(e2 + e3)*cos(e6)*sin(e1)*sin(e4)) + y6*(cos(e6)*(sin(e2 + e3)*sin(e1)*sin(e5) - cos(e2 + e3)*cos(e4)*cos(e5)*sin(e1)) + cos(e2 + e3)*sin(e1)*sin(e4)*sin(e6))) + 2*m6*(x6*(sin(e6)*(sin(e2 + e3)*cos(e1)*sin(e5) - cos(e2 + e3)*cos(e1)*cos(e4)*cos(e5)) - cos(e2 + e3)*cos(e1)*cos(e6)*sin(e4)) + y6*(cos(e6)*(sin(e2 + e3)*cos(e1)*sin(e5) - cos(e2 + e3)*cos(e1)*cos(e4)*cos(e5)) + cos(e2 + e3)*cos(e1)*sin(e4)*sin(e6)))*(x6*(cos(e6)*(cos(e4)*sin(e1) - sin(e2 + e3)*cos(e1)*sin(e4)) - sin(e6)*(cos(e5)*(sin(e1)*sin(e4) + sin(e2 + e3)*cos(e1)*cos(e4)) + cos(e2 + e3)*cos(e1)*sin(e5))) - y6*(sin(e6)*(cos(e4)*sin(e1) - sin(e2 + e3)*cos(e1)*sin(e4)) + cos(e6)*(cos(e5)*(sin(e1)*sin(e4) + sin(e2 + e3)*cos(e1)*cos(e4)) + cos(e2 + e3)*cos(e1)*sin(e5))))))/2 + (de3*(2*m6*(x6*(sin(e6)*(sin(e2 + e3)*sin(e5) - cos(e2 + e3)*cos(e4)*cos(e5)) - cos(e2 + e3)*cos(e6)*sin(e4)) + y6*(cos(e6)*(sin(e2 + e3)*sin(e5) - cos(e2 + e3)*cos(e4)*cos(e5)) + cos(e2 + e3)*sin(e4)*sin(e6)))*(x6*(sin(e6)*(cos(e2 + e3)*sin(e5) + sin(e2 + e3)*cos(e4)*cos(e5)) + sin(e2 + e3)*cos(e6)*sin(e4)) + y6*(cos(e6)*(cos(e2 + e3)*sin(e5) + sin(e2 + e3)*cos(e4)*cos(e5)) - sin(e2 + e3)*sin(e4)*sin(e6))) - 2*m6*(x6*(cos(e6)*(cos(e1)*cos(e4) + sin(e2 + e3)*sin(e1)*sin(e4)) - sin(e6)*(cos(e5)*(cos(e1)*sin(e4) - sin(e2 + e3)*cos(e4)*sin(e1)) - cos(e2 + e3)*sin(e1)*sin(e5))) - y6*(sin(e6)*(cos(e1)*cos(e4) + sin(e2 + e3)*sin(e1)*sin(e4)) + cos(e6)*(cos(e5)*(cos(e1)*sin(e4) - sin(e2 + e3)*cos(e4)*sin(e1)) - cos(e2 + e3)*sin(e1)*sin(e5))))*(x6*(sin(e6)*(sin(e2 + e3)*sin(e1)*sin(e5) - cos(e2 + e3)*cos(e4)*cos(e5)*sin(e1)) - cos(e2 + e3)*cos(e6)*sin(e1)*sin(e4)) + y6*(cos(e6)*(sin(e2 + e3)*sin(e1)*sin(e5) - cos(e2 + e3)*cos(e4)*cos(e5)*sin(e1)) + cos(e2 + e3)*sin(e1)*sin(e4)*sin(e6))) + 2*m6*(x6*(sin(e6)*(sin(e2 + e3)*cos(e1)*sin(e5) - cos(e2 + e3)*cos(e1)*cos(e4)*cos(e5)) - cos(e2 + e3)*cos(e1)*cos(e6)*sin(e4)) + y6*(cos(e6)*(sin(e2 + e3)*cos(e1)*sin(e5) - cos(e2 + e3)*cos(e1)*cos(e4)*cos(e5)) + cos(e2 + e3)*cos(e1)*sin(e4)*sin(e6)))*(x6*(cos(e6)*(cos(e4)*sin(e1) - sin(e2 + e3)*cos(e1)*sin(e4)) - sin(e6)*(cos(e5)*(sin(e1)*sin(e4) + sin(e2 + e3)*cos(e1)*cos(e4)) + cos(e2 + e3)*cos(e1)*sin(e5))) - y6*(sin(e6)*(cos(e4)*sin(e1) - sin(e2 + e3)*cos(e1)*sin(e4)) + cos(e6)*(cos(e5)*(sin(e1)*sin(e4) + sin(e2 + e3)*cos(e1)*cos(e4)) + cos(e2 + e3)*cos(e1)*sin(e5))))))/2 - (de6*(2*m6*(x6*(sin(e6)*(cos(e4)*sin(e1) - sin(e2 + e3)*cos(e1)*sin(e4)) + cos(e6)*(cos(e5)*(sin(e1)*sin(e4) + sin(e2 + e3)*cos(e1)*cos(e4)) + cos(e2 + e3)*cos(e1)*sin(e5))) + y6*(cos(e6)*(cos(e4)*sin(e1) - sin(e2 + e3)*cos(e1)*sin(e4)) - sin(e6)*(cos(e5)*(sin(e1)*sin(e4) + sin(e2 + e3)*cos(e1)*cos(e4)) + cos(e2 + e3)*cos(e1)*sin(e5))))*(x6*(cos(e6)*(cos(e4)*sin(e1) - sin(e2 + e3)*cos(e1)*sin(e4)) - sin(e6)*(cos(e5)*(sin(e1)*sin(e4) + sin(e2 + e3)*cos(e1)*cos(e4)) + cos(e2 + e3)*cos(e1)*sin(e5))) - y6*(sin(e6)*(cos(e4)*sin(e1) - sin(e2 + e3)*cos(e1)*sin(e4)) + cos(e6)*(cos(e5)*(sin(e1)*sin(e4) + sin(e2 + e3)*cos(e1)*cos(e4)) + cos(e2 + e3)*cos(e1)*sin(e5)))) - 2*m6*(x6*(sin(e6)*(sin(e2 + e3)*sin(e5) - cos(e2 + e3)*cos(e4)*cos(e5)) - cos(e2 + e3)*cos(e6)*sin(e4)) + y6*(cos(e6)*(sin(e2 + e3)*sin(e5) - cos(e2 + e3)*cos(e4)*cos(e5)) + cos(e2 + e3)*sin(e4)*sin(e6)))*(x6*(cos(e6)*(sin(e2 + e3)*sin(e5) - cos(e2 + e3)*cos(e4)*cos(e5)) + cos(e2 + e3)*sin(e4)*sin(e6)) - y6*(sin(e6)*(sin(e2 + e3)*sin(e5) - cos(e2 + e3)*cos(e4)*cos(e5)) - cos(e2 + e3)*cos(e6)*sin(e4))) + 2*m6*(x6*(sin(e6)*(cos(e1)*cos(e4) + sin(e2 + e3)*sin(e1)*sin(e4)) + cos(e6)*(cos(e5)*(cos(e1)*sin(e4) - sin(e2 + e3)*cos(e4)*sin(e1)) - cos(e2 + e3)*sin(e1)*sin(e5))) + y6*(cos(e6)*(cos(e1)*cos(e4) + sin(e2 + e3)*sin(e1)*sin(e4)) - sin(e6)*(cos(e5)*(cos(e1)*sin(e4) - sin(e2 + e3)*cos(e4)*sin(e1)) - cos(e2 + e3)*sin(e1)*sin(e5))))*(x6*(cos(e6)*(cos(e1)*cos(e4) + sin(e2 + e3)*sin(e1)*sin(e4)) - sin(e6)*(cos(e5)*(cos(e1)*sin(e4) - sin(e2 + e3)*cos(e4)*sin(e1)) - cos(e2 + e3)*sin(e1)*sin(e5))) - y6*(sin(e6)*(cos(e1)*cos(e4) + sin(e2 + e3)*sin(e1)*sin(e4)) + cos(e6)*(cos(e5)*(cos(e1)*sin(e4) - sin(e2 + e3)*cos(e4)*sin(e1)) - cos(e2 + e3)*sin(e1)*sin(e5))))))/2];

G=...
[0;
g*(a2*m3*sin(e2) + a2*m4*sin(e2) + a2*m5*sin(e2) + a2*m6*sin(e2) + m2*y2*cos(e2) + m2*x2*sin(e2) + d4*m4*cos(e2 + e3) + d4*m5*cos(e2 + e3) + d4*m6*cos(e2 + e3) + a3*m4*sin(e2 + e3) + a3*m5*sin(e2 + e3) + a3*m6*sin(e2 + e3) + m3*y3*cos(e2 + e3) + m4*z4*cos(e2 + e3) + m3*x3*sin(e2 + e3) + m5*y5*cos(e2 + e3)*cos(e5) + m6*z6*cos(e2 + e3)*cos(e5) + m4*x4*sin(e2 + e3)*cos(e4) + m5*x5*cos(e2 + e3)*sin(e5) - m4*y4*sin(e2 + e3)*sin(e4) + m5*z5*sin(e2 + e3)*sin(e4) + m5*x5*sin(e2 + e3)*cos(e4)*cos(e5) + m6*x6*cos(e2 + e3)*cos(e6)*sin(e5) - m5*y5*sin(e2 + e3)*cos(e4)*sin(e5) - m6*y6*sin(e2 + e3)*cos(e6)*sin(e4) - m6*y6*cos(e2 + e3)*sin(e5)*sin(e6) - m6*z6*sin(e2 + e3)*cos(e4)*sin(e5) - m6*x6*sin(e2 + e3)*sin(e4)*sin(e6) + m6*x6*sin(e2 + e3)*cos(e4)*cos(e5)*cos(e6) - m6*y6*sin(e2 + e3)*cos(e4)*cos(e5)*sin(e6));
g*(d4*m4*cos(e2 + e3) + d4*m5*cos(e2 + e3) + d4*m6*cos(e2 + e3) + a3*m4*sin(e2 + e3) + a3*m5*sin(e2 + e3) + a3*m6*sin(e2 + e3) + m3*y3*cos(e2 + e3) + m4*z4*cos(e2 + e3) + m3*x3*sin(e2 + e3) + m5*y5*cos(e2 + e3)*cos(e5) + m6*z6*cos(e2 + e3)*cos(e5) + m4*x4*sin(e2 + e3)*cos(e4) + m5*x5*cos(e2 + e3)*sin(e5) - m4*y4*sin(e2 + e3)*sin(e4) + m5*z5*sin(e2 + e3)*sin(e4) + m5*x5*sin(e2 + e3)*cos(e4)*cos(e5) + m6*x6*cos(e2 + e3)*cos(e6)*sin(e5) - m5*y5*sin(e2 + e3)*cos(e4)*sin(e5) - m6*y6*sin(e2 + e3)*cos(e6)*sin(e4) - m6*y6*cos(e2 + e3)*sin(e5)*sin(e6) - m6*z6*sin(e2 + e3)*cos(e4)*sin(e5) - m6*x6*sin(e2 + e3)*sin(e4)*sin(e6) + m6*x6*sin(e2 + e3)*cos(e4)*cos(e5)*cos(e6) - m6*y6*sin(e2 + e3)*cos(e4)*cos(e5)*sin(e6));
g*cos(e2 + e3)*(m4*y4*cos(e4) - m5*z5*cos(e4) + m4*x4*sin(e4) + m6*y6*cos(e4)*cos(e6) + m5*x5*cos(e5)*sin(e4) + m6*x6*cos(e4)*sin(e6) - m5*y5*sin(e4)*sin(e5) - m6*z6*sin(e4)*sin(e5) + m6*x6*cos(e5)*cos(e6)*sin(e4) - m6*y6*cos(e5)*sin(e4)*sin(e6));
g*(m5*x5*sin(e2 + e3)*cos(e5) - m5*y5*sin(e2 + e3)*sin(e5) - m6*z6*sin(e2 + e3)*sin(e5) + m5*y5*cos(e2 + e3)*cos(e4)*cos(e5) + m6*z6*cos(e2 + e3)*cos(e4)*cos(e5) + m5*x5*cos(e2 + e3)*cos(e4)*sin(e5) + m6*x6*sin(e2 + e3)*cos(e5)*cos(e6) - m6*y6*sin(e2 + e3)*cos(e5)*sin(e6) + m6*x6*cos(e2 + e3)*cos(e4)*cos(e6)*sin(e5) - m6*y6*cos(e2 + e3)*cos(e4)*sin(e5)*sin(e6));
g*m6*(x6*cos(e2 + e3)*cos(e6)*sin(e4) - y6*cos(e2 + e3)*sin(e4)*sin(e6) - y6*sin(e2 + e3)*cos(e6)*sin(e5) - x6*sin(e2 + e3)*sin(e5)*sin(e6) + y6*cos(e2 + e3)*cos(e4)*cos(e5)*cos(e6) + x6*cos(e2 + e3)*cos(e4)*cos(e5)*sin(e6))];

J = ...
[ d4*sin(e1)*sin(e2)*sin(e3) - a2*sin(e1)*sin(e2) - d4*cos(e2)*cos(e3)*sin(e1) - a3*cos(e2)*sin(e1)*sin(e3) - a3*cos(e3)*sin(e1)*sin(e2) - d7*cos(e1)*sin(e4)*sin(e5) - a1*sin(e1) - d7*cos(e2)*cos(e3)*cos(e5)*sin(e1) + d7*cos(e5)*sin(e1)*sin(e2)*sin(e3) + d7*cos(e2)*cos(e4)*sin(e1)*sin(e3)*sin(e5) + d7*cos(e3)*cos(e4)*sin(e1)*sin(e2)*sin(e5), -cos(e1)*(d4*cos(e2)*sin(e3) - a3*cos(e2)*cos(e3) - a2*cos(e2) + d4*cos(e3)*sin(e2) + a3*sin(e2)*sin(e3) + d7*cos(e2)*cos(e5)*sin(e3) + d7*cos(e3)*cos(e5)*sin(e2) + d7*cos(e2)*cos(e3)*cos(e4)*sin(e5) - d7*cos(e4)*sin(e2)*sin(e3)*sin(e5)), -cos(e1)*(d4*cos(e2)*sin(e3) - a3*cos(e2)*cos(e3) + d4*cos(e3)*sin(e2) + a3*sin(e2)*sin(e3) + d7*cos(e2)*cos(e5)*sin(e3) + d7*cos(e3)*cos(e5)*sin(e2) + d7*cos(e2)*cos(e3)*cos(e4)*sin(e5) - d7*cos(e4)*sin(e2)*sin(e3)*sin(e5)), d7*sin(e5)*(cos(e1)*cos(e2)*sin(e3)*sin(e4) - cos(e4)*sin(e1) + cos(e1)*cos(e3)*sin(e2)*sin(e4)), d7*cos(e1)*sin(e2)*sin(e3)*sin(e5) - d7*cos(e1)*cos(e2)*cos(e3)*sin(e5) - d7*cos(e5)*sin(e1)*sin(e4) - d7*cos(e1)*cos(e2)*cos(e4)*cos(e5)*sin(e3) - d7*cos(e1)*cos(e3)*cos(e4)*cos(e5)*sin(e2),                                                                                                                            0;
  a1*cos(e1) + a2*cos(e1)*sin(e2) + d4*cos(e1)*cos(e2)*cos(e3) + a3*cos(e1)*cos(e2)*sin(e3) + a3*cos(e1)*cos(e3)*sin(e2) - d4*cos(e1)*sin(e2)*sin(e3) - d7*sin(e1)*sin(e4)*sin(e5) + d7*cos(e1)*cos(e2)*cos(e3)*cos(e5) - d7*cos(e1)*cos(e5)*sin(e2)*sin(e3) - d7*cos(e1)*cos(e2)*cos(e4)*sin(e3)*sin(e5) - d7*cos(e1)*cos(e3)*cos(e4)*sin(e2)*sin(e5), -sin(e1)*(d4*cos(e2)*sin(e3) - a3*cos(e2)*cos(e3) - a2*cos(e2) + d4*cos(e3)*sin(e2) + a3*sin(e2)*sin(e3) + d7*cos(e2)*cos(e5)*sin(e3) + d7*cos(e3)*cos(e5)*sin(e2) + d7*cos(e2)*cos(e3)*cos(e4)*sin(e5) - d7*cos(e4)*sin(e2)*sin(e3)*sin(e5)), -sin(e1)*(d4*cos(e2)*sin(e3) - a3*cos(e2)*cos(e3) + d4*cos(e3)*sin(e2) + a3*sin(e2)*sin(e3) + d7*cos(e2)*cos(e5)*sin(e3) + d7*cos(e3)*cos(e5)*sin(e2) + d7*cos(e2)*cos(e3)*cos(e4)*sin(e5) - d7*cos(e4)*sin(e2)*sin(e3)*sin(e5)), d7*sin(e5)*(cos(e1)*cos(e4) + cos(e2)*sin(e1)*sin(e3)*sin(e4) + cos(e3)*sin(e1)*sin(e2)*sin(e4)), d7*cos(e1)*cos(e5)*sin(e4) - d7*cos(e2)*cos(e3)*sin(e1)*sin(e5) + d7*sin(e1)*sin(e2)*sin(e3)*sin(e5) - d7*cos(e2)*cos(e4)*cos(e5)*sin(e1)*sin(e3) - d7*cos(e3)*cos(e4)*cos(e5)*sin(e1)*sin(e2),                                                                                                                            0;
                                                                                                                                                                                                                                                                                                                                                     0,            d4*sin(e2)*sin(e3) - d4*cos(e2)*cos(e3) - a3*cos(e2)*sin(e3) - a3*cos(e3)*sin(e2) - a2*sin(e2) - d7*cos(e2)*cos(e3)*cos(e5) + d7*cos(e5)*sin(e2)*sin(e3) + d7*cos(e2)*cos(e4)*sin(e3)*sin(e5) + d7*cos(e3)*cos(e4)*sin(e2)*sin(e5),            d4*sin(e2)*sin(e3) - a3*cos(e2)*sin(e3) - a3*cos(e3)*sin(e2) - d4*cos(e2)*cos(e3) - d7*cos(e2)*cos(e3)*cos(e5) + d7*cos(e5)*sin(e2)*sin(e3) + d7*cos(e2)*cos(e4)*sin(e3)*sin(e5) + d7*cos(e3)*cos(e4)*sin(e2)*sin(e5),                                                                  d7*cos(e2 + e3)*sin(e4)*sin(e5),                                                              d7*cos(e2)*sin(e3)*sin(e5) + d7*cos(e3)*sin(e2)*sin(e5) - d7*cos(e2)*cos(e3)*cos(e4)*cos(e5) + d7*cos(e4)*cos(e5)*sin(e2)*sin(e3),                                                                                                                            0;
                                                                                                                                                                                                                                                                                                                                                     0,                                                                                                                                                                                                                                      -sin(e1),                                                                                                                                                                                                                         -sin(e1),                                                                             cos(e2 + e3)*cos(e1),                                                                                                            cos(e1)*cos(e2)*sin(e3)*sin(e4) - cos(e4)*sin(e1) + cos(e1)*cos(e3)*sin(e2)*sin(e4), cos(e2 + e3)*cos(e1)*cos(e5) - sin(e5)*(sin(e1)*sin(e4) + cos(e1)*cos(e2)*cos(e4)*sin(e3) + cos(e1)*cos(e3)*cos(e4)*sin(e2));
                                                                                                                                                                                                                                                                                                                                                     0,                                                                                                                                                                                                                                       cos(e1),                                                                                                                                                                                                                          cos(e1),                                                                             cos(e2 + e3)*sin(e1),                                                                                                            cos(e1)*cos(e4) + cos(e2)*sin(e1)*sin(e3)*sin(e4) + cos(e3)*sin(e1)*sin(e2)*sin(e4), cos(e2 + e3)*cos(e5)*sin(e1) - sin(e5)*(cos(e2)*cos(e4)*sin(e1)*sin(e3) - cos(e1)*sin(e4) + cos(e3)*cos(e4)*sin(e1)*sin(e2));                                                                                                                                                                                                                                                                                                                                                   1,                                                                                                                                                                                                                                             0,                                                                                                                                                                                                                                0,                                                                                    -sin(e2 + e3),                                                                                                                                                                           cos(e2 + e3)*sin(e4),                                                                        - sin(e2 + e3)*cos(e5) - cos(e2 + e3)*cos(e4)*sin(e5)];
%%
de = [de1;de2;de3;de4;de5;de6];
F = c*sign(de) + b*de + J'*Fe ;
dde = M\(t-C*de-G-F);
